simulink model "ABB_1010"  (R2024a)
(part 16 of 16)

et304 = Lx2*Lycm6*dQ1*dQ6*m6*t5*t6*t7*t9*-2.0+Lx2*Lycm6*dQ2*dQ4*m6*t3*t5*t9*t11*2.0+Lx2*Lycm6*dQ2*dQ5*m6*t3*t4*t10*t11*2.0+Lx2*Lycm6*dQ3*dQ4*m6*t3*t5*t9*t11*2.0+Lx2*Lycm6*dQ3*dQ5*m6*t3*t4*t10*t11*2.0+Lx2*Lycm6*dQ4*dQ6*m6*t5*t6*t8*t9*2.0+Lx2*Lycm6*dQ5*dQ6*m6*t4*t6*t8*t10*2.0+Lx2*Lycm6*dQ1*dQ5*m6*t7*t9*t10*t11*2.0-Lx2*Lycm6*dQ4*dQ5*m6*t8*t9*t10*t11*2.0;
et305 = t42+t45+t48+t49+t50+t51+t52+t53+t54+t55+t56+t57+t58+t59+t60+t61+t72+t73+t74+t75+t76+t77+t78+t79+t80+t81+t82+t83+t86+t92+t93+t95+t96+t97+t98+t99+t100+t101+t102+t103+t108+t109+t110+t111+t114+t115+t116+t117+t118+t127+t128+t131+t132+t137+t138+t139+t140+t141+t142+t143+t144+t145+t146+t147+t152+t153+t154+t157+t158+t160+t161+t163+t164+t165+t166+t167+t168+t169+t170+t171+t172+t173+t174+t175+t176+t177+t178+t179+t180+t181+t182+t183+t184+t185+t186+t187+t188+t189+t190+t191+t192+t199+t201+t208+t211+t212+t227+t228+t229+t230+t231+t232+t233+t234+t235+t236+t252+t253+t254+t255+t256+t257+t262+t263+t264+t265+t266+t277+t278+t279+t280+t281+t282+t289+t290+t291+t292+t293+t294+t295+t296+t297+t298+t299+t300+t301+t302+t303+t304+t305+t306+t307+t308+t309+t310+t311+t312+t313+t314+t316+t318+t320+t321+t322+t323+t324+t325+t326+t327+t328+t329+t330+t331+t332+t333+t334+t335+t336+t337+t338+t339+t340+t341+t342+t343+t344+t345+t346+t347+t348+t349+t350+t351+t352+t353+t354+t355+t356+t357+t358;
et306 = t363+t364+t365+t366+t369+t370+t371+t372+t380+t382+t383+t384+t385+t386+t387+t388+t389+t401+t402+t403+t404+t409+t410+t411+t412+t413+t414+t415+t416+t417+t418+t419+t420+t421+t422+t423+t424+t425+t426+t427+t428+t429+t430+t431+t436+t437+t438+t439+t440+t441+t442+t443+t446+t447+t450+t451+t454+t459+t460+t461+t463+t464+t465+t471+t472+t473+t474+t476+t477+t478+t479+t480+t481+t492+t493+t494+t495+t496+t497+t498+t499+t500+t501+t503+t506+t509+t510+t511+t512+t513+t516+t518+t519+t521+t522+t524+t525+t527+t528+t542+t543+t544+t545+t546+t547+t548+t549+t551+t552+t556+t557+t558+t559+t560+t561+t562+t563+t564+t565+t566+t567+t568+t569+t570+t571+t572+t573+t574+t575+t576+t577+t578+t579+t580+t581+t582+t583+t584+t585+t586+t587+t588+t589+t590+t591+t592+t593+t595+t596+t597+t598+t599+t600+t607+t608+t609+t610+t611+t612+t613+t614+t615+t616+t617+t618+t619+t620+t621+t622+t623+t624+t625+t626+t627+t628+t629+t630+t631+t632+t633+t634+t635+t636+t637+t638+t639+t640+t641+t642+t643+t644+t645+t646+t647+t648+t649+t650+t651+t654+t655;
et307 = t656+t657+t658+t659+t660+t668+t674+t675+t676+t677+t686+t687+t691+t692+t693+t694+t695+t696+t697+t701+t702+t703+t704+t705+t706+t707+t708+t709+t710+t711+t712+t713+t714+t715+t716+t724+t736+t737+t742+t743+t744+t745+t746+t747+t756+t757+t758+t761+t762+t763+t765+t767+t768+t770+t772+t773+t774+t776+t777+t778+t779+t780+t781+t782+t783+t787+t788+t789+t790+t791+t792+t793+t794+t795+t806+t807+t808+t809+t816+t819+t820+t821+t822+t823+t824+t825+t826+t827+t830+t833+t834+t836+t837+t843+t844+t845+t846+t847+t848+t849+t850+t851+t852+t853+t854+t855+t856+t857+t858+t859+t860+t861+t862+t863+t864+t865+t866+t867+t868+t869+t870+t871+t872+t873+t874+t875+t876+t877+t878+t879+t880+t881+t882+t883+t884+t885+t886+t887+t888+t889+t890+t891+t892+t893+t894+t895+t896+t897+t898+t899+t900+t901+t902+t903+t904+t905+t906+t907+t909+t910+t911+t912+t913+t914+t915+t916+t917+t918+t919+t920+t921+t922+t923+t924+t925+t926+t927+t928+t929+t930+t931+t932+t933+t934+t935+t936+t937+t938+t939+t940+t941+t942+t943+t944+t955+t957+t958+t960+t961+t967;
et308 = t968+t970+t973+t976+t979+t982+t983+t984+t985+t986+t987+t988+t989+t990+t991+t992+t993+t994+t995+t996+t997+t998+t999+t1000+t1001+t1002+t1003+t1004+t1005+t1006+t1007+t1008+t1009+t1010+t1015+t1016+t1017+t1018+t1019+t1020+t1023+t1024+t1031+t1032+t1033+t1034+t1039+t1042+t1043+t1044+t1045+t1046+t1049+t1050+t1058+t1059+t1060+t1061+t1062+t1063+t1066+t1067+t1068+t1069+t1070+t1071+t1074+t1077+t1079+t1082+t1083+t1084+t1085+t1086+t1087+t1088+t1090+t1091+t1092+t1093+t1094+t1095+t1096+t1097+t1098+t1099+t1100+t1101+t1102+t1103+t1104+t1105+t1106+t1107+t1108+t1109+t1110+t1111+t1112+t1113+t1114+t1115+t1125+t1126+t1127+t1128+t1129+t1130+t1131+t1132+t1133+t1134+t1135+t1136+t1137+t1140+t1143+t1144+t1147+t1150+t1151+t1152+t1153+t1154+t1155+t1156+t1174+t1175+t1177+t1178+t1182+t1183+t1185+t1186+t1187+t1188+t1189+t1190+t1197+t1200+t1201+t1202+t1203+t1204+t1205+t1206+t1207+t1208+t1209+t1210+t1211+t1212+t1213+t1214+t1215+t1216+t1218+t1219+t1220+t1221+t1222+t1223+t1224+t1225+t1226+t1227+t1228+t1229+t1230+t1231+t1232+t1233+t1234+t1235+t1245+t1246+t1247+t1248+t1249+t1250+t1251+t1252+t1253+t1254+t1258+t1260+t1263+t1264+t1265+t1266+t1267+t1268+t1269+t1270+t1271+t1272+t1273+t1274+t1275+t1276;
et309 = t1277+t1278+t1279+t1280+t1281+t1282+t1283+t1284+t1285+t1286+t1287+t1288+t1289+t1293+t1294+t1295+t1296+t1297+t1298+t1299+t1300+t1301+t1302+t1303+t1304+t1305+t1306+t1307+t1308+t1309+t1310+t1311+t1312+t1313+t1314+t1315+t1316+t1317+t1318+t1319+t1321+t1322+t1323+t1324+t1331+t1332+t1333+t1334+t1335+t1336+t1337+t1341+t1342+t1343+t1344+t1345+t1346+t1347+t1348+t1349+t1350+t1351+t1352+t1355+t1356+t1362+t1363+t1364+t1365+t1366+t1367+t1368+t1369+t1370+t1371+t1372+t1373+t1374+t1375+t1376+t1377+t1378+t1379+t1380+t1381+t1382+t1383+t1384+t1396+t1401+t1402+t1403+t1404+t1405+t1406+t1407+t1408+t1409+t1410+t1411+t1412+t1416+t1417+t1418+t1419+t1420+t1434+t1435+t1436+t1437+t1438+t1439+t1440+t1441+t1449+t1450+t1451+t1455+t1456+t1457+t1460+t1461+t1462+t1463+t1465+t1466+t1467+t1468+t1469+t1470+t1471+t1472+t1473+t1474+t1475+t1476+t1477+t1478+t1479+t1480+t1481+t1482+t1484+t1485+t1486+t1487+t1488+t1489+t1490+t1491+t1492+t1493+t1494+t1495+t1496+t1498+t1499+t1500+t1501+t1502+t1503+t1504+t1505+t1506+t1507+t1508+t1509+t1510+t1511+t1512+t1513+t1514+t1515+t1516+t1517+t1518+t1519+t1520+t1521+t1522+t1530+t1531+t1532+t1533+t1534+t1535+t1536+t1537+t1538+t1539+t1540+t1541+t1542+t1543+t1545+t1546+t1547+t1548+t1549+t1550;
et310 = t1557+t1558+t1561+t1562+t1563+t1564+t1565+t1566+t1573+t1574+t1575+t1578+t1579+t1580+t1586+t1587+t1594+t1595+t1596+t1597+t1598+t1599+t1600+t1601+t1602+t1603+t1604+t1605+t1606+t1607+t1608+t1609+t1610+t1611+t1612+t1613+t1614+t1615+t1618+t1619+t1620+t1621+t1622+t1623+t1624+t1625+t1626+t1627+t1628+t1629+t1645+t1646+t1647+t1648+t1649+t1650+t1651+t1652+t1653+t1654+t1655+t1656+t1657+t1658+t1662+t1663+t1664+t1665+t1667+t1668+t1669+t1670+t1671+t1676+t1677+t1678+t1683+t1685+t1686+t1687+t1688+t1689+t1690+t1691+t1692+t1693+t1694+t1695+t1696+t1697+t1698+t1699+t1700+t1701+t1706+t1707+t1708+t1709+t1710+t1711+t1712+t1713+t1714+t1715+t1716+t1717+t1718+t1719+t1720+t1721+t1722+t1727+t1728+t1729+t1730+t1731+t1732+t1735+t1736+t1737+t1738+t1739+t1740;
et311 = Ixx5*dQ2*dQ5*t9+Ixx5*dQ3*dQ5*t9+Ixx6*dQ2*dQ5*t9+Ixx6*dQ3*dQ5*t9+Ixx6*dQ5*dQ6*t10-Ixx4*dQ2*dQ3*t39+Ixx6*dQ2*dQ3*t39+Ixx5*dQ4*dQ5*t40-Ixx6*dQ4*dQ6*t41+Iyy5*dQ2*dQ5*t9+Iyy5*dQ3*dQ5*t9+Iyy6*dQ2*dQ5*t9+Iyy6*dQ3*dQ5*t9-Iyy6*dQ5*dQ6*t10+Iyy4*dQ2*dQ3*t39+Iyy5*dQ2*dQ3*t39+Iyy6*dQ4*dQ5*t40+Iyy6*dQ4*dQ6*t41-Izz5*dQ2*dQ5*t9-Izz5*dQ3*dQ5*t9-Izz6*dQ2*dQ5*t9-Izz6*dQ3*dQ5*t9-Izz6*dQ5*dQ6*t10-Izz5*dQ2*dQ3*t39-Izz6*dQ2*dQ3*t39-Izz5*dQ4*dQ5*t40-Izz6*dQ4*dQ5*t40-Lx4*Lycm4*dQ2*dQ3*m4*2.0-Lx4*Lycm5*dQ2*dQ3*m5*2.0-Lxcm4*Lycm4*dQ2*dQ3*m4*2.0-Lxcm6*Lycm6*dQ4*dQ6*m6*2.0-Lxcm5*Lzcm5*dQ4*dQ5*m5*2.0;
et312 = -Ixx4*dQ1*dQ2*t2*t8-Ixx4*dQ1*dQ2*t3*t7-Ixx4*dQ1*dQ3*t2*t8-Ixx4*dQ1*dQ3*t3*t7-Ixx5*dQ1*dQ2*t2*t8-Ixx5*dQ1*dQ2*t3*t7-Ixx5*dQ1*dQ3*t2*t8-Ixx5*dQ1*dQ3*t3*t7+Ixx6*dQ1*dQ2*t2*t8+Ixx6*dQ1*dQ2*t3*t7+Ixx6*dQ1*dQ3*t2*t8+Ixx6*dQ1*dQ3*t3*t7+Ixx6*dQ2*dQ6*t4*t10+Ixx6*dQ3*dQ6*t4*t10-Ixx5*dQ2*dQ5*t9*t35*2.0-Ixx5*dQ3*dQ5*t9*t35*2.0-Ixx6*dQ5*dQ6*t10*t36*2.0+Iyy4*dQ1*dQ2*t2*t8+Iyy4*dQ1*dQ2*t3*t7+Iyy4*dQ1*dQ3*t2*t8+Iyy4*dQ1*dQ3*t3*t7+Iyy5*dQ1*dQ2*t2*t8+Iyy5*dQ1*dQ2*t3*t7+Iyy5*dQ1*dQ3*t2*t8+Iyy5*dQ1*dQ3*t3*t7-Iyy6*dQ1*dQ2*t2*t8-Iyy6*dQ1*dQ2*t3*t7-Iyy6*dQ1*dQ3*t2*t8;
et313 = -Iyy6*dQ1*dQ3*t3*t7-Iyy6*dQ2*dQ6*t4*t10-Iyy6*dQ3*dQ6*t4*t10-Iyy6*dQ2*dQ5*t9*t35*2.0-Iyy6*dQ3*dQ5*t9*t35*2.0+Iyy6*dQ5*dQ6*t10*t36*2.0-Izz4*dQ1*dQ2*t2*t8-Izz4*dQ1*dQ2*t3*t7-Izz4*dQ1*dQ3*t2*t8-Izz4*dQ1*dQ3*t3*t7-Izz5*dQ1*dQ2*t2*t8-Izz5*dQ1*dQ2*t3*t7-Izz5*dQ1*dQ3*t2*t8-Izz5*dQ1*dQ3*t3*t7-Izz6*dQ1*dQ2*t2*t8-Izz6*dQ1*dQ2*t3*t7-Izz6*dQ1*dQ3*t2*t8-Izz6*dQ1*dQ3*t3*t7-Izz6*dQ2*dQ6*t4*t10-Izz6*dQ3*dQ6*t4*t10+Izz5*dQ2*dQ5*t9*t35*2.0+Izz5*dQ3*dQ5*t9*t35*2.0+Izz6*dQ2*dQ5*t9*t35*2.0+Izz6*dQ3*dQ5*t9*t35*2.0+dQ2*dQ5*m6*t9*t22*2.0;
et314 = dQ3*dQ5*m6*t9*t22*2.0-dQ5*dQ6*m6*t10*t18*2.0+dQ2*dQ5*m5*t9*t25*2.0+dQ3*dQ5*m5*t9*t25*2.0+dQ2*dQ5*m6*t9*t26*2.0+dQ3*dQ5*m6*t9*t26*2.0+dQ2*dQ3*m4*t14*t39+dQ2*dQ3*m5*t14*t39+dQ2*dQ3*m4*t16*t39+dQ2*dQ3*m6*t14*t39-dQ2*dQ3*m4*t19*t39-dQ2*dQ3*m6*t18*t39-dQ2*dQ3*m5*t20*t39-dQ4*dQ5*m5*t17*t40+dQ2*dQ3*m6*t22*t39+dQ2*dQ3*m5*t25*t39+dQ4*dQ6*m6*t18*t41+dQ2*dQ3*m6*t26*t39-dQ4*dQ5*m6*t21*t40+dQ4*dQ5*m6*t22*t40-dQ4*dQ6*m6*t21*t41+dQ4*dQ5*m5*t25*t40+dQ4*dQ5*m6*t26*t40-t4*t6*t10*t11*t149*2.0-t4*t6*t10*t11*t150*2.0+t4*t6*t10*t11*t153*2.0+t4*t6*t10*t11*t154*2.0+t4*t6*t10*t11*t595+t4*t6*t10*t11*t596;
et315 = Lx3*Lx4*dQ2*dQ3*m4*t9*2.0+Lx3*Lx4*dQ2*dQ3*m5*t9*2.0+Lx3*Lx4*dQ2*dQ3*m6*t9*2.0+Lx3*Lxcm4*dQ2*dQ3*m4*t9*2.0-Lx4*Lxcm6*dQ2*dQ3*m6*t11*2.0-Lx4*Lxcm5*dQ4*dQ5*m5*t10*2.0+Lx4*Lxcm4*dQ2*dQ3*m4*t39*2.0+Lx3*Lycm4*dQ2*dQ3*m4*t4*2.0+Lx3*Lycm5*dQ2*dQ3*m5*t4*2.0-Lx4*Lycm6*dQ2*dQ3*m6*t6*2.0+Lx4*Lycm4*dQ2*dQ3*m4*t34*4.0+Lx4*Lycm5*dQ2*dQ3*m5*t34*4.0-Lxcm5*Lycm5*dQ2*dQ3*m5*t5*2.0+Lxcm6*Lycm6*dQ2*dQ3*m6*t5*2.0+Lxcm4*Lycm4*dQ2*dQ3*m4*t34*4.0+Lxcm6*Lycm6*dQ4*dQ6*m6*t35*2.0+Lxcm6*Lycm6*dQ4*dQ6*m6*t36*4.0+Lx4*Lz6*dQ4*dQ5*m6*t5*2.0+Lx4*Lzcm5*dQ4*dQ5*m5*t5*2.0+Lx4*Lzcm6*dQ4*dQ5*m6*t5*2.0-Lxcm6*Lz6*dQ4*dQ5*m6*t6*2.0-Lxcm6*Lzcm6*dQ4*dQ5*m6*t6*2.0+Lxcm5*Lzcm5*dQ4*dQ5*m5*t35*4.0+Lycm6*Lz6*dQ4*dQ5*m6*t11*2.0;
et316 = Lycm5*Lzcm5*dQ2*dQ3*m5*t10*-2.0+Lycm6*Lzcm6*dQ4*dQ5*m6*t11*2.0+Lz6*Lzcm6*dQ2*dQ5*m6*t9*4.0+Lz6*Lzcm6*dQ3*dQ5*m6*t9*4.0+Lz6*Lzcm6*dQ2*dQ3*m6*t39*2.0+Lz6*Lzcm6*dQ4*dQ5*m6*t40*2.0-Ixx5*dQ1*dQ5*t2*t4*t8-Ixx5*dQ1*dQ5*t3*t4*t7-Ixx6*dQ1*dQ5*t2*t4*t8-Ixx6*dQ1*dQ5*t3*t4*t7+Ixx6*dQ2*dQ3*t5*t6*t11*2.0+Ixx4*dQ1*dQ2*t2*t8*t34*2.0+Ixx4*dQ1*dQ2*t3*t7*t34*2.0+Ixx4*dQ1*dQ3*t2*t8*t34*2.0+Ixx4*dQ1*dQ3*t3*t7*t34*2.0-Ixx6*dQ1*dQ2*t2*t8*t34*2.0-Ixx6*dQ1*dQ2*t3*t7*t34*2.0-Ixx6*dQ1*dQ3*t2*t8*t34*2.0-Ixx6*dQ1*dQ3*t3*t7*t34*2.0-Ixx6*dQ1*dQ2*t2*t8*t36*2.0-Ixx6*dQ1*dQ2*t3*t7*t36*2.0-Ixx6*dQ1*dQ3*t2*t8*t36*2.0-Ixx6*dQ1*dQ3*t3*t7*t36*2.0;
et317 = Ixx5*dQ2*dQ3*t4*t9*t35*-2.0-Ixx6*dQ2*dQ3*t4*t9*t36*2.0-Ixx6*dQ2*dQ6*t4*t10*t36*2.0-Ixx6*dQ3*dQ6*t4*t10*t36*2.0+Ixx6*dQ4*dQ5*t5*t10*t36*2.0+Ixx6*dQ4*dQ6*t6*t11*t35*2.0-Ixx6*dQ2*dQ5*t9*t35*t36*2.0-Ixx6*dQ3*dQ5*t9*t35*t36*2.0-Iyy5*dQ1*dQ5*t2*t4*t8-Iyy5*dQ1*dQ5*t3*t4*t7-Iyy6*dQ1*dQ5*t2*t4*t8-Iyy6*dQ1*dQ5*t3*t4*t7-Iyy6*dQ2*dQ3*t5*t6*t11*2.0-Iyy4*dQ1*dQ2*t2*t8*t34*2.0-Iyy4*dQ1*dQ2*t3*t7*t34*2.0-Iyy4*dQ1*dQ3*t2*t8*t34*2.0-Iyy4*dQ1*dQ3*t3*t7*t34*2.0-Iyy5*dQ1*dQ2*t2*t8*t34*2.0-Iyy5*dQ1*dQ2*t3*t7*t34*2.0-Iyy5*dQ1*dQ3*t2*t8*t34*2.0-Iyy5*dQ1*dQ3*t3*t7*t34*2.0+Iyy6*dQ1*dQ2*t2*t8*t36*2.0;
et318 = Iyy6*dQ1*dQ2*t3*t7*t36*2.0+Iyy6*dQ1*dQ3*t2*t8*t36*2.0+Iyy6*dQ1*dQ3*t3*t7*t36*2.0-Iyy6*dQ2*dQ3*t4*t9*t35*2.0+Iyy6*dQ2*dQ3*t4*t9*t36*2.0+Iyy6*dQ2*dQ6*t4*t10*t36*2.0+Iyy6*dQ3*dQ6*t4*t10*t36*2.0-Iyy6*dQ4*dQ5*t5*t10*t36*2.0-Iyy6*dQ4*dQ6*t6*t11*t35*2.0+Iyy6*dQ2*dQ5*t9*t35*t36*2.0+Iyy6*dQ3*dQ5*t9*t35*t36*2.0+Izz5*dQ1*dQ5*t2*t4*t8+Izz5*dQ1*dQ5*t3*t4*t7+Izz6*dQ1*dQ5*t2*t4*t8+Izz6*dQ1*dQ5*t3*t4*t7+Izz5*dQ1*dQ2*t2*t8*t34*2.0+Izz5*dQ1*dQ2*t3*t7*t34*2.0+Izz5*dQ1*dQ3*t2*t8*t34*2.0+Izz5*dQ1*dQ3*t3*t7*t34*2.0+Izz6*dQ1*dQ2*t2*t8*t34*2.0+Izz6*dQ1*dQ2*t3*t7*t34*2.0+Izz6*dQ1*dQ3*t2*t8*t34*2.0+Izz6*dQ1*dQ3*t3*t7*t34*2.0+Izz5*dQ2*dQ3*t4*t9*t35*2.0+Izz6*dQ2*dQ3*t4*t9*t35*2.0;
et319 = dQ1*dQ2*m4*t2*t8*t19*-2.0-dQ1*dQ2*m4*t3*t7*t19*2.0-dQ1*dQ2*m6*t2*t8*t18*2.0-dQ1*dQ2*m6*t3*t7*t18*2.0-dQ1*dQ3*m4*t2*t8*t19*2.0-dQ1*dQ3*m4*t3*t7*t19*2.0-dQ1*dQ2*m5*t2*t8*t20*2.0-dQ1*dQ2*m5*t3*t7*t20*2.0-dQ1*dQ3*m6*t2*t8*t18*2.0-dQ1*dQ3*m6*t3*t7*t18*2.0-dQ1*dQ3*m5*t2*t8*t20*2.0-dQ1*dQ3*m5*t3*t7*t20*2.0-dQ2*dQ6*m6*t4*t10*t18*2.0-dQ3*dQ6*m6*t4*t10*t18*2.0+dQ2*dQ5*m5*t9*t17*t35*2.0+dQ3*dQ5*m5*t9*t17*t35*2.0+dQ2*dQ5*m6*t9*t21*t35*2.0-dQ2*dQ5*m6*t9*t22*t35*2.0+dQ3*dQ5*m6*t9*t21*t35*2.0-dQ3*dQ5*m6*t9*t22*t35*2.0-dQ2*dQ5*m5*t9*t25*t35*2.0+dQ5*dQ6*m6*t10*t18*t36*2.0;
et320 = dQ3*dQ5*m5*t9*t25*t35*-2.0-dQ2*dQ5*m6*t9*t26*t35*2.0-dQ3*dQ5*m6*t9*t26*t35*2.0-dQ5*dQ6*m6*t10*t21*t36*2.0-Lx2*Lx4*dQ1*dQ2*m4*t4*t7*2.0-Lx2*Lx4*dQ1*dQ2*m5*t4*t7*2.0-Lx2*Lx4*dQ1*dQ2*m6*t4*t7*2.0-Lx2*Lxcm4*dQ1*dQ2*m4*t4*t7*2.0+Lx3*Lxcm5*dQ2*dQ3*m5*t5*t9*2.0+Lx3*Lxcm6*dQ2*dQ3*m6*t4*t11*2.0+Lx4*Lxcm5*dQ2*dQ5*m5*t5*t9*2.0+Lx4*Lxcm5*dQ3*dQ5*m5*t5*t9*2.0-Lx4*Lxcm6*dQ4*dQ5*m6*t6*t10*2.0-Lx4*Lxcm6*dQ4*dQ6*m6*t5*t11*2.0+Lx4*Lxcm6*dQ2*dQ3*m6*t11*t34*4.0+Lx2*Lycm4*dQ1*dQ2*m4*t7*t9*2.0+Lx3*Lycm6*dQ2*dQ3*m6*t4*t6*2.0+Lx2*Lycm5*dQ1*dQ2*m5*t7*t9*2.0-Lx4*Lycm6*dQ4*dQ6*m6*t5*t6*2.0+Lx4*Lycm6*dQ4*dQ5*m6*t10*t11*2.0+Lx4*Lycm6*dQ2*dQ3*m6*t6*t34*4.0;
et321 = Lxcm6*Lycm6*dQ1*dQ6*m6*t2*t3*-2.0+Lxcm5*Lycm5*dQ2*dQ5*m5*t4*t5*2.0+Lxcm5*Lycm5*dQ3*dQ5*m5*t4*t5*2.0-Lxcm6*Lycm6*dQ2*dQ5*m6*t4*t5*2.0-Lxcm6*Lycm6*dQ3*dQ5*m6*t4*t5*2.0+Lxcm6*Lycm6*dQ1*dQ6*m6*t7*t8*2.0+Lxcm5*Lycm5*dQ2*dQ3*m5*t5*t34*4.0-Lxcm6*Lycm6*dQ2*dQ3*m6*t5*t34*4.0-Lxcm6*Lycm6*dQ2*dQ3*m6*t5*t36*4.0-Lxcm6*Lycm6*dQ4*dQ6*m6*t35*t36*4.0+Lx3*Lz6*dQ2*dQ3*m6*t9*t10*2.0+Lx4*Lz6*dQ2*dQ5*m6*t9*t10*2.0+Lx4*Lz6*dQ3*dQ5*m6*t9*t10*2.0+Lx3*Lzcm5*dQ2*dQ3*m5*t9*t10*2.0+Lx3*Lzcm6*dQ2*dQ3*m6*t9*t10*2.0+Lx4*Lzcm5*dQ2*dQ5*m5*t9*t10*2.0+Lx4*Lzcm5*dQ3*dQ5*m5*t9*t10*2.0+Lx4*Lzcm6*dQ2*dQ5*m6*t9*t10*2.0+Lx4*Lzcm6*dQ3*dQ5*m6*t9*t10*2.0-Lxcm6*Lz6*dQ2*dQ3*m6*t10*t11*2.0-Lxcm6*Lz6*dQ2*dQ6*m6*t9*t11*2.0;
et322 = Lxcm6*Lz6*dQ3*dQ6*m6*t9*t11*-2.0+Lxcm6*Lz6*dQ4*dQ5*m6*t6*t35*4.0-Lxcm5*Lzcm5*dQ1*dQ5*m5*t2*t3*2.0+Lxcm5*Lzcm5*dQ1*dQ5*m5*t7*t8*2.0-Lxcm6*Lzcm6*dQ2*dQ3*m6*t10*t11*2.0-Lxcm6*Lzcm6*dQ2*dQ6*m6*t9*t11*2.0-Lxcm6*Lzcm6*dQ3*dQ6*m6*t9*t11*2.0+Lxcm6*Lzcm6*dQ4*dQ5*m6*t6*t35*4.0-Lycm6*Lz6*dQ2*dQ3*m6*t6*t10*2.0-Lycm6*Lz6*dQ2*dQ6*m6*t6*t9*2.0-Lycm6*Lz6*dQ3*dQ6*m6*t6*t9*2.0-Lycm6*Lz6*dQ4*dQ5*m6*t11*t35*4.0+Lycm5*Lzcm5*dQ2*dQ5*m5*t4*t10*2.0+Lycm5*Lzcm5*dQ3*dQ5*m5*t4*t10*2.0-Lycm6*Lzcm6*dQ2*dQ3*m6*t6*t10*2.0-Lycm6*Lzcm6*dQ2*dQ6*m6*t6*t9*2.0-Lycm6*Lzcm6*dQ3*dQ6*m6*t6*t9*2.0+Lycm5*Lzcm5*dQ2*dQ3*m5*t10*t34*4.0-Lycm6*Lzcm6*dQ4*dQ5*m6*t11*t35*4.0-Lz6*Lzcm6*dQ2*dQ5*m6*t9*t35*4.0;
et323 = Lz6*Lzcm6*dQ3*dQ5*m6*t9*t35*-4.0+Ixx5*dQ1*dQ5*t2*t3*t5*t10*2.0-Ixx6*dQ1*dQ6*t2*t3*t6*t11*2.0-Ixx6*dQ2*dQ5*t4*t5*t6*t11*2.0-Ixx6*dQ3*dQ5*t4*t5*t6*t11*2.0-Ixx5*dQ1*dQ5*t5*t7*t8*t10*2.0+Ixx6*dQ1*dQ6*t2*t8*t9*t10+Ixx6*dQ1*dQ6*t3*t7*t9*t10+Ixx6*dQ1*dQ6*t6*t7*t8*t11*2.0+Ixx5*dQ1*dQ5*t2*t4*t8*t35*2.0+Ixx5*dQ1*dQ5*t3*t4*t7*t35*2.0-Ixx6*dQ2*dQ3*t5*t6*t11*t34*4.0+Ixx5*dQ1*dQ2*t2*t8*t34*t35*2.0+Ixx5*dQ1*dQ2*t3*t7*t34*t35*2.0+Ixx5*dQ1*dQ3*t2*t8*t34*t35*2.0+Ixx5*dQ1*dQ3*t3*t7*t34*t35*2.0+Ixx6*dQ1*dQ2*t2*t8*t34*t36*2.0+Ixx6*dQ1*dQ2*t3*t7*t34*t36*2.0+Ixx6*dQ1*dQ3*t2*t8*t34*t36*2.0+Ixx6*dQ1*dQ3*t3*t7*t34*t36*2.0-Ixx6*dQ2*dQ3*t4*t9*t35*t36*2.0;
et324 = Iyy6*dQ1*dQ5*t2*t3*t5*t10*2.0+Iyy6*dQ1*dQ6*t2*t3*t6*t11*2.0+Iyy6*dQ2*dQ5*t4*t5*t6*t11*2.0+Iyy6*dQ3*dQ5*t4*t5*t6*t11*2.0-Iyy6*dQ1*dQ5*t5*t7*t8*t10*2.0-Iyy6*dQ1*dQ6*t2*t8*t9*t10-Iyy6*dQ1*dQ6*t3*t7*t9*t10-Iyy6*dQ1*dQ6*t6*t7*t8*t11*2.0+Iyy6*dQ1*dQ5*t2*t4*t8*t35*2.0+Iyy6*dQ1*dQ5*t3*t4*t7*t35*2.0+Iyy6*dQ2*dQ3*t5*t6*t11*t34*4.0+Iyy6*dQ1*dQ2*t2*t8*t34*t35*2.0+Iyy6*dQ1*dQ2*t3*t7*t34*t35*2.0-Iyy6*dQ1*dQ2*t2*t8*t34*t36*2.0-Iyy6*dQ1*dQ2*t3*t7*t34*t36*2.0+Iyy6*dQ1*dQ3*t2*t8*t34*t35*2.0+Iyy6*dQ1*dQ3*t3*t7*t34*t35*2.0-Iyy6*dQ1*dQ3*t2*t8*t34*t36*2.0-Iyy6*dQ1*dQ3*t3*t7*t34*t36*2.0+Iyy6*dQ2*dQ3*t4*t9*t35*t36*2.0-Izz5*dQ1*dQ5*t2*t3*t5*t10*2.0;
et325 = Izz6*dQ1*dQ5*t2*t3*t5*t10*-2.0+Izz5*dQ1*dQ5*t5*t7*t8*t10*2.0+Izz6*dQ1*dQ5*t5*t7*t8*t10*2.0-Izz6*dQ1*dQ6*t2*t8*t9*t10-Izz6*dQ1*dQ6*t3*t7*t9*t10-Izz5*dQ1*dQ5*t2*t4*t8*t35*2.0-Izz5*dQ1*dQ5*t3*t4*t7*t35*2.0-Izz6*dQ1*dQ5*t2*t4*t8*t35*2.0-Izz6*dQ1*dQ5*t3*t4*t7*t35*2.0-Izz5*dQ1*dQ2*t2*t8*t34*t35*2.0-Izz5*dQ1*dQ2*t3*t7*t34*t35*2.0-Izz5*dQ1*dQ3*t2*t8*t34*t35*2.0-Izz5*dQ1*dQ3*t3*t7*t34*t35*2.0-Izz6*dQ1*dQ2*t2*t8*t34*t35*2.0-Izz6*dQ1*dQ2*t3*t7*t34*t35*2.0-Izz6*dQ1*dQ3*t2*t8*t34*t35*2.0-Izz6*dQ1*dQ3*t3*t7*t34*t35*2.0-dQ1*dQ5*m6*t2*t4*t8*t22*2.0-dQ1*dQ5*m6*t3*t4*t7*t22*2.0-dQ1*dQ5*m5*t2*t4*t8*t25*2.0;
et326 = dQ1*dQ5*m5*t3*t4*t7*t25*-2.0-dQ2*dQ3*m6*t5*t6*t11*t18*2.0-dQ1*dQ5*m6*t2*t4*t8*t26*2.0-dQ1*dQ5*m6*t3*t4*t7*t26*2.0+dQ2*dQ3*m6*t5*t6*t11*t21*2.0-dQ1*dQ2*m4*t2*t8*t14*t34*2.0-dQ1*dQ2*m4*t3*t7*t14*t34*2.0-dQ1*dQ2*m5*t2*t8*t14*t34*2.0-dQ1*dQ2*m5*t3*t7*t14*t34*2.0-dQ1*dQ3*m4*t2*t8*t14*t34*2.0-dQ1*dQ3*m4*t3*t7*t14*t34*2.0-dQ1*dQ2*m4*t2*t8*t16*t34*2.0-dQ1*dQ2*m4*t3*t7*t16*t34*2.0-dQ1*dQ2*m6*t2*t8*t14*t34*2.0-dQ1*dQ2*m6*t3*t7*t14*t34*2.0-dQ1*dQ3*m5*t2*t8*t14*t34*2.0-dQ1*dQ3*m5*t3*t7*t14*t34*2.0-dQ1*dQ3*m4*t2*t8*t16*t34*2.0-dQ1*dQ3*m4*t3*t7*t16*t34*2.0-dQ1*dQ3*m6*t2*t8*t14*t34*2.0;
et327 = dQ1*dQ3*m6*t3*t7*t14*t34*-2.0+dQ1*dQ2*m4*t2*t8*t19*t34*2.0+dQ1*dQ2*m4*t3*t7*t19*t34*2.0+dQ1*dQ2*m6*t2*t8*t18*t34*2.0+dQ1*dQ2*m6*t3*t7*t18*t34*2.0+dQ1*dQ3*m4*t2*t8*t19*t34*2.0+dQ1*dQ3*m4*t3*t7*t19*t34*2.0+dQ1*dQ2*m5*t2*t8*t20*t34*2.0+dQ1*dQ2*m5*t3*t7*t20*t34*2.0+dQ1*dQ3*m6*t2*t8*t18*t34*2.0+dQ1*dQ3*m6*t3*t7*t18*t34*2.0+dQ1*dQ2*m6*t2*t8*t18*t36*2.0+dQ1*dQ2*m6*t3*t7*t18*t36*2.0+dQ1*dQ3*m5*t2*t8*t20*t34*2.0+dQ1*dQ3*m5*t3*t7*t20*t34*2.0+dQ1*dQ3*m6*t2*t8*t18*t36*2.0+dQ1*dQ3*m6*t3*t7*t18*t36*2.0-dQ1*dQ2*m6*t2*t8*t22*t34*2.0-dQ1*dQ2*m6*t3*t7*t22*t34*2.0+dQ2*dQ3*m5*t4*t9*t17*t35*2.0-dQ1*dQ2*m6*t2*t8*t21*t36*2.0;
et328 = dQ1*dQ2*m6*t3*t7*t21*t36*-2.0-dQ1*dQ3*m6*t2*t8*t22*t34*2.0-dQ1*dQ3*m6*t3*t7*t22*t34*2.0-dQ1*dQ2*m5*t2*t8*t25*t34*2.0-dQ1*dQ2*m5*t3*t7*t25*t34*2.0-dQ1*dQ3*m6*t2*t8*t21*t36*2.0-dQ1*dQ3*m6*t3*t7*t21*t36*2.0-dQ1*dQ3*m5*t2*t8*t25*t34*2.0-dQ1*dQ3*m5*t3*t7*t25*t34*2.0+dQ2*dQ3*m6*t4*t9*t18*t36*2.0-dQ1*dQ2*m6*t2*t8*t26*t34*2.0-dQ1*dQ2*m6*t3*t7*t26*t34*2.0-dQ1*dQ3*m6*t2*t8*t26*t34*2.0-dQ1*dQ3*m6*t3*t7*t26*t34*2.0+dQ2*dQ3*m6*t4*t9*t21*t35*2.0-dQ2*dQ3*m6*t4*t9*t21*t36*2.0-dQ2*dQ3*m6*t4*t9*t22*t35*2.0+dQ2*dQ6*m6*t4*t10*t18*t36*2.0-dQ2*dQ3*m5*t4*t9*t25*t35*2.0+dQ3*dQ6*m6*t4*t10*t18*t36*2.0;
et329 = dQ4*dQ5*m6*t5*t10*t18*t36*-2.0-dQ2*dQ3*m6*t4*t9*t26*t35*2.0-dQ2*dQ6*m6*t4*t10*t21*t36*2.0-dQ3*dQ6*m6*t4*t10*t21*t36*2.0-dQ4*dQ6*m6*t6*t11*t18*t35*2.0+dQ4*dQ5*m6*t5*t10*t21*t36*2.0+dQ4*dQ6*m6*t6*t11*t21*t35*2.0+dQ2*dQ5*m6*t9*t18*t35*t36*2.0+dQ3*dQ5*m6*t9*t18*t35*t36*2.0-dQ2*dQ5*m6*t9*t21*t35*t36*2.0-dQ3*dQ5*m6*t9*t21*t35*t36*2.0-Lx3*Lx4*dQ1*dQ2*m4*t2*t4*t8*2.0-Lx3*Lx4*dQ1*dQ2*m4*t3*t4*t7*2.0-Lx3*Lx4*dQ1*dQ2*m5*t2*t4*t8*2.0-Lx3*Lx4*dQ1*dQ2*m5*t3*t4*t7*2.0-Lx3*Lx4*dQ1*dQ3*m4*t2*t4*t8*2.0-Lx3*Lx4*dQ1*dQ3*m4*t3*t4*t7*2.0-Lx3*Lx4*dQ1*dQ2*m6*t2*t4*t8*2.0-Lx3*Lx4*dQ1*dQ2*m6*t3*t4*t7*2.0;
et330 = Lx3*Lx4*dQ1*dQ3*m5*t2*t4*t8*-2.0-Lx3*Lx4*dQ1*dQ3*m5*t3*t4*t7*2.0-Lx3*Lx4*dQ1*dQ3*m6*t2*t4*t8*2.0-Lx3*Lx4*dQ1*dQ3*m6*t3*t4*t7*2.0-Lx3*Lxcm4*dQ1*dQ2*m4*t2*t4*t8*2.0-Lx3*Lxcm4*dQ1*dQ2*m4*t3*t4*t7*2.0-Lx3*Lxcm4*dQ1*dQ3*m4*t2*t4*t8*2.0-Lx3*Lxcm4*dQ1*dQ3*m4*t3*t4*t7*2.0-Lx2*Lxcm5*dQ1*dQ2*m5*t4*t5*t7*2.0-Lx4*Lxcm5*dQ1*dQ5*m5*t2*t3*t10*2.0+Lx4*Lxcm5*dQ2*dQ3*m5*t4*t5*t9*4.0+Lx3*Lxcm6*dQ2*dQ3*m6*t5*t6*t9*2.0+Lx4*Lxcm6*dQ2*dQ5*m6*t5*t6*t9*2.0+Lx2*Lxcm6*dQ1*dQ2*m6*t7*t9*t11*2.0+Lx4*Lxcm6*dQ3*dQ5*m6*t5*t6*t9*2.0+Lx4*Lxcm5*dQ1*dQ5*m5*t7*t8*t10*2.0-Lx4*Lxcm6*dQ2*dQ6*m6*t9*t10*t11*2.0-Lx4*Lxcm6*dQ3*dQ6*m6*t9*t10*t11*2.0;
et331 = Lx4*Lxcm4*dQ1*dQ2*m4*t2*t8*t34*-4.0-Lx4*Lxcm4*dQ1*dQ2*m4*t3*t7*t34*4.0-Lx4*Lxcm4*dQ1*dQ3*m4*t2*t8*t34*4.0-Lx4*Lxcm4*dQ1*dQ3*m4*t3*t7*t34*4.0+Lx3*Lycm4*dQ1*dQ2*m4*t2*t8*t9*2.0+Lx3*Lycm4*dQ1*dQ2*m4*t3*t7*t9*2.0+Lx3*Lycm4*dQ1*dQ3*m4*t2*t8*t9*2.0+Lx3*Lycm4*dQ1*dQ3*m4*t3*t7*t9*2.0+Lx3*Lycm5*dQ1*dQ2*m5*t2*t8*t9*2.0+Lx3*Lycm5*dQ1*dQ2*m5*t3*t7*t9*2.0+Lx3*Lycm5*dQ1*dQ3*m5*t2*t8*t9*2.0+Lx3*Lycm5*dQ1*dQ3*m5*t3*t7*t9*2.0+Lx2*Lycm6*dQ1*dQ2*m6*t6*t7*t9*2.0-Lx3*Lycm6*dQ2*dQ3*m6*t5*t9*t11*2.0-Lx4*Lycm6*dQ2*dQ5*m6*t5*t9*t11*2.0-Lx4*Lycm6*dQ2*dQ6*m6*t6*t9*t10*2.0-Lx4*Lycm6*dQ3*dQ5*m6*t5*t9*t11*2.0-Lx4*Lycm6*dQ3*dQ6*m6*t6*t9*t10*2.0+Lxcm6*Lycm6*dQ2*dQ6*m6*t5*t9*t10*2.0;
et332 = Lxcm6*Lycm6*dQ3*dQ6*m6*t5*t9*t10*2.0-Lxcm6*Lycm6*dQ5*dQ6*m6*t6*t10*t11*4.0+Lxcm6*Lycm6*dQ1*dQ6*m6*t2*t3*t35*2.0+Lxcm6*Lycm6*dQ1*dQ6*m6*t2*t3*t36*4.0+Lxcm6*Lycm6*dQ2*dQ5*m6*t4*t5*t36*4.0+Lxcm6*Lycm6*dQ3*dQ5*m6*t4*t5*t36*4.0-Lxcm6*Lycm6*dQ1*dQ6*m6*t7*t8*t35*2.0-Lxcm6*Lycm6*dQ1*dQ6*m6*t7*t8*t36*4.0+Lxcm6*Lycm6*dQ2*dQ3*m6*t5*t34*t36*8.0+Lx4*Lz6*dQ1*dQ5*m6*t2*t3*t5*2.0-Lx2*Lz6*dQ1*dQ2*m6*t4*t7*t10*2.0-Lx4*Lz6*dQ1*dQ5*m6*t5*t7*t8*2.0+Lx4*Lz6*dQ2*dQ3*m6*t4*t9*t10*4.0+Lx4*Lzcm4*dQ1*dQ2*m4*t2*t3*t4*2.0+Lx4*Lzcm4*dQ1*dQ3*m4*t2*t3*t4*2.0+Lx4*Lzcm5*dQ1*dQ5*m5*t2*t3*t5*2.0+Lx4*Lzcm6*dQ1*dQ5*m6*t2*t3*t5*2.0-Lx4*Lzcm4*dQ1*dQ2*m4*t4*t7*t8*2.0-Lx4*Lzcm4*dQ1*dQ3*m4*t4*t7*t8*2.0;
et333 = Lxcm6*Lz6*dQ1*dQ5*m6*t2*t3*t6*-2.0-Lx2*Lzcm5*dQ1*dQ2*m5*t4*t7*t10*2.0-Lx2*Lzcm6*dQ1*dQ2*m6*t4*t7*t10*2.0-Lx4*Lzcm5*dQ1*dQ5*m5*t5*t7*t8*2.0+Lx4*Lzcm5*dQ2*dQ3*m5*t4*t9*t10*4.0-Lx4*Lzcm6*dQ1*dQ5*m6*t5*t7*t8*2.0+Lx4*Lzcm6*dQ2*dQ3*m6*t4*t9*t10*4.0+Lxcm6*Lz6*dQ1*dQ5*m6*t6*t7*t8*2.0+Lxcm6*Lz6*dQ2*dQ5*m6*t4*t10*t11*2.0+Lxcm6*Lz6*dQ3*dQ5*m6*t4*t10*t11*2.0-Lxcm6*Lz6*dQ4*dQ6*m6*t5*t10*t11*2.0+Lxcm6*Lz6*dQ2*dQ3*m6*t10*t11*t34*4.0+Lxcm6*Lz6*dQ2*dQ6*m6*t9*t11*t35*2.0+Lxcm6*Lz6*dQ3*dQ6*m6*t9*t11*t35*2.0+Lxcm4*Lzcm4*dQ1*dQ2*m4*t2*t3*t4*2.0+Lxcm4*Lzcm4*dQ1*dQ3*m4*t2*t3*t4*2.0-Lxcm5*Lzcm5*dQ1*dQ2*m5*t2*t3*t4*2.0-Lxcm5*Lzcm5*dQ1*dQ3*m5*t2*t3*t4*2.0-Lxcm4*Lzcm4*dQ1*dQ2*m4*t4*t7*t8*2.0;
et334 = Lxcm4*Lzcm4*dQ1*dQ3*m4*t4*t7*t8*-2.0-Lxcm6*Lzcm6*dQ1*dQ5*m6*t2*t3*t6*2.0+Lxcm5*Lzcm5*dQ1*dQ2*m5*t4*t7*t8*2.0+Lxcm5*Lzcm5*dQ1*dQ3*m5*t4*t7*t8*2.0+Lxcm6*Lzcm6*dQ1*dQ5*m6*t6*t7*t8*2.0+Lxcm5*Lzcm5*dQ2*dQ5*m5*t5*t9*t10*4.0+Lxcm5*Lzcm5*dQ3*dQ5*m5*t5*t9*t10*4.0+Lxcm6*Lzcm6*dQ2*dQ5*m6*t4*t10*t11*2.0+Lxcm6*Lzcm6*dQ3*dQ5*m6*t4*t10*t11*2.0-Lxcm6*Lzcm6*dQ4*dQ6*m6*t5*t10*t11*2.0+Lxcm5*Lzcm5*dQ1*dQ5*m5*t2*t3*t35*4.0-Lxcm5*Lzcm5*dQ1*dQ5*m5*t7*t8*t35*4.0+Lxcm6*Lzcm6*dQ2*dQ3*m6*t10*t11*t34*4.0+Lxcm6*Lzcm6*dQ2*dQ6*m6*t9*t11*t35*2.0+Lxcm6*Lzcm6*dQ3*dQ6*m6*t9*t11*t35*2.0+Lycm6*Lz6*dQ1*dQ5*m6*t2*t3*t11*2.0+Lycm6*Lz6*dQ2*dQ5*m6*t4*t6*t10*2.0+Lycm6*Lz6*dQ3*dQ5*m6*t4*t6*t10*2.0-Lycm6*Lz6*dQ4*dQ6*m6*t5*t6*t10*2.0;
et335 = Lycm6*Lz6*dQ1*dQ5*m6*t7*t8*t11*-2.0+Lycm6*Lz6*dQ2*dQ3*m6*t6*t10*t34*4.0+Lycm6*Lz6*dQ2*dQ6*m6*t6*t9*t35*2.0+Lycm6*Lz6*dQ3*dQ6*m6*t6*t9*t35*2.0-Lycm4*Lzcm4*dQ1*dQ2*m4*t2*t3*t9*2.0-Lycm4*Lzcm4*dQ1*dQ3*m4*t2*t3*t9*2.0+Lycm4*Lzcm4*dQ1*dQ2*m4*t7*t8*t9*2.0+Lycm4*Lzcm4*dQ1*dQ3*m4*t7*t8*t9*2.0+Lycm6*Lzcm6*dQ1*dQ5*m6*t2*t3*t11*2.0+Lycm6*Lzcm6*dQ2*dQ5*m6*t4*t6*t10*2.0+Lycm6*Lzcm6*dQ3*dQ5*m6*t4*t6*t10*2.0-Lycm6*Lzcm6*dQ4*dQ6*m6*t5*t6*t10*2.0-Lycm6*Lzcm6*dQ1*dQ5*m6*t7*t8*t11*2.0+Lycm6*Lzcm6*dQ2*dQ3*m6*t6*t10*t34*4.0+Lycm6*Lzcm6*dQ2*dQ6*m6*t6*t9*t35*2.0+Lycm6*Lzcm6*dQ3*dQ6*m6*t6*t9*t35*2.0-Lz6*Lzcm6*dQ1*dQ5*m6*t2*t4*t8*4.0-Lz6*Lzcm6*dQ1*dQ5*m6*t3*t4*t7*4.0-Lz6*Lzcm6*dQ1*dQ2*m6*t2*t8*t34*4.0;
et336 = Lz6*Lzcm6*dQ1*dQ2*m6*t3*t7*t34*-4.0-Lz6*Lzcm6*dQ1*dQ3*m6*t2*t8*t34*4.0-Lz6*Lzcm6*dQ1*dQ3*m6*t3*t7*t34*4.0-Lz6*Lzcm6*dQ2*dQ3*m6*t4*t9*t35*4.0+Ixx5*dQ1*dQ2*t2*t3*t4*t5*t10*2.0+Ixx5*dQ1*dQ3*t2*t3*t4*t5*t10*2.0-Ixx5*dQ1*dQ2*t4*t5*t7*t8*t10*2.0-Ixx5*dQ1*dQ3*t4*t5*t7*t8*t10*2.0+Ixx6*dQ2*dQ6*t5*t6*t9*t10*t11*2.0+Ixx6*dQ3*dQ6*t5*t6*t9*t10*t11*2.0+Ixx6*dQ1*dQ5*t2*t3*t5*t10*t36*2.0+Ixx6*dQ1*dQ6*t2*t3*t6*t11*t35*2.0-Ixx6*dQ1*dQ5*t5*t7*t8*t10*t36*2.0-Ixx6*dQ1*dQ6*t2*t8*t9*t10*t36*2.0-Ixx6*dQ1*dQ6*t3*t7*t9*t10*t36*2.0-Ixx6*dQ1*dQ6*t6*t7*t8*t11*t35*2.0+Ixx6*dQ1*dQ5*t2*t4*t8*t35*t36*2.0+Ixx6*dQ1*dQ5*t3*t4*t7*t35*t36*2.0+Ixx6*dQ1*dQ2*t2*t8*t34*t35*t36*2.0;
et337 = Ixx6*dQ1*dQ2*t3*t7*t34*t35*t36*2.0+Ixx6*dQ1*dQ3*t2*t8*t34*t35*t36*2.0+Ixx6*dQ1*dQ3*t3*t7*t34*t35*t36*2.0+Iyy6*dQ1*dQ2*t2*t3*t4*t5*t10*2.0+Iyy6*dQ1*dQ3*t2*t3*t4*t5*t10*2.0-Iyy6*dQ1*dQ2*t4*t5*t7*t8*t10*2.0-Iyy6*dQ1*dQ3*t4*t5*t7*t8*t10*2.0-Iyy6*dQ2*dQ6*t5*t6*t9*t10*t11*2.0-Iyy6*dQ3*dQ6*t5*t6*t9*t10*t11*2.0-Iyy6*dQ1*dQ5*t2*t3*t5*t10*t36*2.0-Iyy6*dQ1*dQ6*t2*t3*t6*t11*t35*2.0+Iyy6*dQ1*dQ5*t5*t7*t8*t10*t36*2.0+Iyy6*dQ1*dQ6*t2*t8*t9*t10*t36*2.0+Iyy6*dQ1*dQ6*t3*t7*t9*t10*t36*2.0+Iyy6*dQ1*dQ6*t6*t7*t8*t11*t35*2.0-Iyy6*dQ1*dQ5*t2*t4*t8*t35*t36*2.0-Iyy6*dQ1*dQ5*t3*t4*t7*t35*t36*2.0-Iyy6*dQ1*dQ2*t2*t8*t34*t35*t36*2.0-Iyy6*dQ1*dQ2*t3*t7*t34*t35*t36*2.0;
et338 = Iyy6*dQ1*dQ3*t2*t8*t34*t35*t36*-2.0-Iyy6*dQ1*dQ3*t3*t7*t34*t35*t36*2.0-Izz5*dQ1*dQ2*t2*t3*t4*t5*t10*2.0-Izz5*dQ1*dQ3*t2*t3*t4*t5*t10*2.0-Izz6*dQ1*dQ2*t2*t3*t4*t5*t10*2.0-Izz6*dQ1*dQ3*t2*t3*t4*t5*t10*2.0+Izz5*dQ1*dQ2*t4*t5*t7*t8*t10*2.0+Izz5*dQ1*dQ3*t4*t5*t7*t8*t10*2.0+Izz6*dQ1*dQ2*t4*t5*t7*t8*t10*2.0+Izz6*dQ1*dQ3*t4*t5*t7*t8*t10*2.0-dQ1*dQ5*m5*t2*t3*t5*t10*t17*2.0-dQ1*dQ5*m6*t2*t3*t5*t10*t21*2.0+dQ1*dQ6*m6*t2*t3*t6*t11*t18*2.0+dQ1*dQ5*m6*t2*t3*t5*t10*t22*2.0+dQ1*dQ5*m5*t2*t3*t5*t10*t25*2.0-dQ1*dQ6*m6*t2*t3*t6*t11*t21*2.0+dQ2*dQ5*m6*t4*t5*t6*t11*t18*2.0+dQ1*dQ5*m5*t5*t7*t8*t10*t17*2.0+dQ1*dQ5*m6*t2*t3*t5*t10*t26*2.0;
et339 = dQ3*dQ5*m6*t4*t5*t6*t11*t18*2.0-dQ1*dQ6*m6*t2*t8*t9*t10*t18*2.0-dQ1*dQ6*m6*t3*t7*t9*t10*t18*2.0-dQ2*dQ5*m6*t4*t5*t6*t11*t21*2.0-dQ3*dQ5*m6*t4*t5*t6*t11*t21*2.0+dQ1*dQ5*m6*t5*t7*t8*t10*t21*2.0-dQ1*dQ6*m6*t6*t7*t8*t11*t18*2.0-dQ1*dQ5*m6*t5*t7*t8*t10*t22*2.0-dQ1*dQ5*m5*t5*t7*t8*t10*t25*2.0+dQ1*dQ6*m6*t6*t7*t8*t11*t21*2.0-dQ1*dQ5*m6*t5*t7*t8*t10*t26*2.0-dQ1*dQ5*m5*t2*t4*t8*t17*t35*2.0-dQ1*dQ5*m5*t3*t4*t7*t17*t35*2.0-dQ1*dQ5*m6*t2*t4*t8*t21*t35*2.0-dQ1*dQ5*m6*t3*t4*t7*t21*t35*2.0+dQ1*dQ5*m6*t2*t4*t8*t22*t35*2.0+dQ1*dQ5*m6*t3*t4*t7*t22*t35*2.0+dQ1*dQ5*m5*t2*t4*t8*t25*t35*2.0;
et340 = dQ1*dQ5*m5*t3*t4*t7*t25*t35*2.0+dQ2*dQ3*m6*t5*t6*t11*t18*t34*4.0+dQ1*dQ5*m6*t2*t4*t8*t26*t35*2.0+dQ1*dQ5*m6*t3*t4*t7*t26*t35*2.0-dQ2*dQ3*m6*t5*t6*t11*t21*t34*4.0-dQ1*dQ2*m5*t2*t8*t17*t34*t35*2.0-dQ1*dQ2*m5*t3*t7*t17*t34*t35*2.0-dQ1*dQ3*m5*t2*t8*t17*t34*t35*2.0-dQ1*dQ3*m5*t3*t7*t17*t34*t35*2.0-dQ1*dQ2*m6*t2*t8*t18*t34*t36*2.0-dQ1*dQ2*m6*t3*t7*t18*t34*t36*2.0-dQ1*dQ3*m6*t2*t8*t18*t34*t36*2.0-dQ1*dQ3*m6*t3*t7*t18*t34*t36*2.0-dQ1*dQ2*m6*t2*t8*t21*t34*t35*2.0-dQ1*dQ2*m6*t3*t7*t21*t34*t35*2.0+dQ1*dQ2*m6*t2*t8*t21*t34*t36*2.0+dQ1*dQ2*m6*t2*t8*t22*t34*t35*2.0+dQ1*dQ2*m6*t3*t7*t21*t34*t36*2.0;
et341 = dQ1*dQ2*m6*t3*t7*t22*t34*t35*2.0-dQ1*dQ3*m6*t2*t8*t21*t34*t35*2.0-dQ1*dQ3*m6*t3*t7*t21*t34*t35*2.0+dQ1*dQ3*m6*t2*t8*t21*t34*t36*2.0+dQ1*dQ3*m6*t2*t8*t22*t34*t35*2.0+dQ1*dQ3*m6*t3*t7*t21*t34*t36*2.0+dQ1*dQ3*m6*t3*t7*t22*t34*t35*2.0+dQ1*dQ2*m5*t2*t8*t25*t34*t35*2.0+dQ1*dQ2*m5*t3*t7*t25*t34*t35*2.0+dQ1*dQ3*m5*t2*t8*t25*t34*t35*2.0+dQ1*dQ3*m5*t3*t7*t25*t34*t35*2.0+dQ2*dQ3*m6*t4*t9*t18*t35*t36*2.0+dQ1*dQ2*m6*t2*t8*t26*t34*t35*2.0+dQ1*dQ2*m6*t3*t7*t26*t34*t35*2.0+dQ1*dQ3*m6*t2*t8*t26*t34*t35*2.0+dQ1*dQ3*m6*t3*t7*t26*t34*t35*2.0-dQ2*dQ3*m6*t4*t9*t21*t35*t36*2.0-Ixx6*dQ1*dQ2*t2*t3*t6*t9*t10*t11*2.0-Ixx6*dQ1*dQ3*t2*t3*t6*t9*t10*t11*2.0;
et342 = Ixx6*dQ1*dQ5*t2*t5*t6*t8*t9*t11*-2.0-Ixx6*dQ1*dQ5*t3*t5*t6*t7*t9*t11*2.0+Ixx6*dQ1*dQ2*t6*t7*t8*t9*t10*t11*2.0+Ixx6*dQ1*dQ3*t6*t7*t8*t9*t10*t11*2.0+Ixx6*dQ1*dQ2*t2*t3*t4*t5*t10*t36*2.0+Ixx6*dQ1*dQ3*t2*t3*t4*t5*t10*t36*2.0-Ixx6*dQ1*dQ2*t4*t5*t7*t8*t10*t36*2.0-Ixx6*dQ1*dQ3*t4*t5*t7*t8*t10*t36*2.0+Iyy6*dQ1*dQ2*t2*t3*t6*t9*t10*t11*2.0+Iyy6*dQ1*dQ3*t2*t3*t6*t9*t10*t11*2.0+Iyy6*dQ1*dQ5*t2*t5*t6*t8*t9*t11*2.0+Iyy6*dQ1*dQ5*t3*t5*t6*t7*t9*t11*2.0-Iyy6*dQ1*dQ2*t6*t7*t8*t9*t10*t11*2.0-Iyy6*dQ1*dQ3*t6*t7*t8*t9*t10*t11*2.0-Iyy6*dQ1*dQ2*t2*t3*t4*t5*t10*t36*2.0-Iyy6*dQ1*dQ3*t2*t3*t4*t5*t10*t36*2.0+Iyy6*dQ1*dQ2*t4*t5*t7*t8*t10*t36*2.0;
et343 = Iyy6*dQ1*dQ3*t4*t5*t7*t8*t10*t36*2.0-dQ1*dQ2*m5*t2*t3*t4*t5*t10*t17*2.0-dQ1*dQ3*m5*t2*t3*t4*t5*t10*t17*2.0-dQ1*dQ2*m6*t2*t3*t4*t5*t10*t21*2.0+dQ1*dQ2*m6*t2*t3*t4*t5*t10*t22*2.0-dQ1*dQ3*m6*t2*t3*t4*t5*t10*t21*2.0+dQ1*dQ3*m6*t2*t3*t4*t5*t10*t22*2.0+dQ1*dQ2*m5*t2*t3*t4*t5*t10*t25*2.0+dQ1*dQ3*m5*t2*t3*t4*t5*t10*t25*2.0+dQ1*dQ2*m5*t4*t5*t7*t8*t10*t17*2.0+dQ1*dQ2*m6*t2*t3*t4*t5*t10*t26*2.0+dQ1*dQ3*m5*t4*t5*t7*t8*t10*t17*2.0+dQ1*dQ3*m6*t2*t3*t4*t5*t10*t26*2.0+dQ1*dQ2*m6*t4*t5*t7*t8*t10*t21*2.0-dQ1*dQ2*m6*t4*t5*t7*t8*t10*t22*2.0+dQ1*dQ3*m6*t4*t5*t7*t8*t10*t21*2.0-dQ1*dQ3*m6*t4*t5*t7*t8*t10*t22*2.0;
et344 = dQ1*dQ2*m5*t4*t5*t7*t8*t10*t25*-2.0-dQ1*dQ3*m5*t4*t5*t7*t8*t10*t25*2.0-dQ1*dQ2*m6*t4*t5*t7*t8*t10*t26*2.0-dQ1*dQ3*m6*t4*t5*t7*t8*t10*t26*2.0-dQ2*dQ6*m6*t5*t6*t9*t10*t11*t18*2.0-dQ3*dQ6*m6*t5*t6*t9*t10*t11*t18*2.0+dQ2*dQ6*m6*t5*t6*t9*t10*t11*t21*2.0+dQ3*dQ6*m6*t5*t6*t9*t10*t11*t21*2.0-dQ1*dQ5*m6*t2*t3*t5*t10*t18*t36*2.0-dQ1*dQ6*m6*t2*t3*t6*t11*t18*t35*2.0+dQ1*dQ5*m6*t2*t3*t5*t10*t21*t36*2.0+dQ1*dQ6*m6*t2*t3*t6*t11*t21*t35*2.0+dQ1*dQ5*m6*t5*t7*t8*t10*t18*t36*2.0+dQ1*dQ6*m6*t2*t8*t9*t10*t18*t36*2.0+dQ1*dQ6*m6*t3*t7*t9*t10*t18*t36*2.0+dQ1*dQ6*m6*t6*t7*t8*t11*t18*t35*2.0-dQ1*dQ5*m6*t5*t7*t8*t10*t21*t36*2.0;
et345 = dQ1*dQ6*m6*t2*t8*t9*t10*t21*t36*-2.0-dQ1*dQ6*m6*t3*t7*t9*t10*t21*t36*2.0-dQ1*dQ6*m6*t6*t7*t8*t11*t21*t35*2.0-dQ1*dQ5*m6*t2*t4*t8*t18*t35*t36*2.0-dQ1*dQ5*m6*t3*t4*t7*t18*t35*t36*2.0+dQ1*dQ5*m6*t2*t4*t8*t21*t35*t36*2.0+dQ1*dQ5*m6*t3*t4*t7*t21*t35*t36*2.0-dQ1*dQ2*m6*t2*t8*t18*t34*t35*t36*2.0-dQ1*dQ2*m6*t3*t7*t18*t34*t35*t36*2.0-dQ1*dQ3*m6*t2*t8*t18*t34*t35*t36*2.0-dQ1*dQ3*m6*t3*t7*t18*t34*t35*t36*2.0+dQ1*dQ2*m6*t2*t8*t21*t34*t35*t36*2.0+dQ1*dQ2*m6*t3*t7*t21*t34*t35*t36*2.0+dQ1*dQ3*m6*t2*t8*t21*t34*t35*t36*2.0+dQ1*dQ3*m6*t3*t7*t21*t34*t35*t36*2.0-Lx3*Lxcm5*dQ1*dQ2*m5*t2*t4*t5*t8*2.0-Lx3*Lxcm5*dQ1*dQ2*m5*t3*t4*t5*t7*2.0;
et346 = Lx3*Lxcm5*dQ1*dQ3*m5*t2*t4*t5*t8*-2.0-Lx3*Lxcm5*dQ1*dQ3*m5*t3*t4*t5*t7*2.0-Lx4*Lxcm5*dQ1*dQ2*m5*t2*t3*t4*t10*2.0-Lx4*Lxcm5*dQ1*dQ3*m5*t2*t3*t4*t10*2.0-Lx2*Lxcm6*dQ1*dQ2*m6*t4*t5*t6*t7*2.0-Lx4*Lxcm5*dQ1*dQ5*m5*t2*t4*t5*t8*2.0-Lx4*Lxcm5*dQ1*dQ5*m5*t3*t4*t5*t7*2.0-Lx4*Lxcm6*dQ1*dQ5*m6*t2*t3*t6*t10*2.0-Lx4*Lxcm6*dQ1*dQ6*m6*t2*t3*t5*t11*2.0+Lx4*Lxcm6*dQ2*dQ3*m6*t4*t5*t6*t9*4.0+Lx4*Lxcm5*dQ1*dQ2*m5*t4*t7*t8*t10*2.0+Lx4*Lxcm5*dQ1*dQ3*m5*t4*t7*t8*t10*2.0+Lx3*Lxcm6*dQ1*dQ2*m6*t2*t8*t9*t11*2.0+Lx3*Lxcm6*dQ1*dQ2*m6*t3*t7*t9*t11*2.0+Lx3*Lxcm6*dQ1*dQ3*m6*t2*t8*t9*t11*2.0+Lx3*Lxcm6*dQ1*dQ3*m6*t3*t7*t9*t11*2.0+Lx4*Lxcm6*dQ1*dQ5*m6*t6*t7*t8*t10*2.0;
et347 = Lx4*Lxcm6*dQ1*dQ6*m6*t5*t7*t8*t11*2.0-Lx4*Lxcm5*dQ1*dQ2*m5*t2*t5*t8*t34*4.0-Lx4*Lxcm5*dQ1*dQ2*m5*t3*t5*t7*t34*4.0-Lx4*Lxcm5*dQ1*dQ3*m5*t2*t5*t8*t34*4.0-Lx4*Lxcm5*dQ1*dQ3*m5*t3*t5*t7*t34*4.0+Lx4*Lycm4*dQ1*dQ2*m4*t2*t4*t8*t9*4.0+Lx4*Lycm4*dQ1*dQ2*m4*t3*t4*t7*t9*4.0+Lx4*Lycm4*dQ1*dQ3*m4*t2*t4*t8*t9*4.0+Lx4*Lycm4*dQ1*dQ3*m4*t3*t4*t7*t9*4.0-Lx4*Lycm6*dQ1*dQ6*m6*t2*t3*t5*t6*2.0+Lx4*Lycm5*dQ1*dQ2*m5*t2*t4*t8*t9*4.0+Lx4*Lycm5*dQ1*dQ2*m5*t3*t4*t7*t9*4.0+Lx4*Lycm5*dQ1*dQ3*m5*t2*t4*t8*t9*4.0+Lx4*Lycm5*dQ1*dQ3*m5*t3*t4*t7*t9*4.0+Lx3*Lycm6*dQ1*dQ2*m6*t2*t6*t8*t9*2.0+Lx3*Lycm6*dQ1*dQ2*m6*t3*t6*t7*t9*2.0+Lx2*Lycm6*dQ1*dQ2*m6*t4*t5*t7*t11*2.0;
et348 = Lx3*Lycm6*dQ1*dQ3*m6*t2*t6*t8*t9*2.0+Lx3*Lycm6*dQ1*dQ3*m6*t3*t6*t7*t9*2.0+Lx4*Lycm6*dQ1*dQ5*m6*t2*t3*t10*t11*2.0+Lx4*Lycm6*dQ1*dQ6*m6*t5*t6*t7*t8*2.0-Lx4*Lycm6*dQ2*dQ3*m6*t4*t5*t9*t11*4.0-Lx4*Lycm6*dQ1*dQ5*m6*t7*t8*t10*t11*2.0+Lxcm4*Lycm4*dQ1*dQ2*m4*t2*t4*t8*t9*4.0+Lxcm4*Lycm4*dQ1*dQ2*m4*t3*t4*t7*t9*4.0+Lxcm4*Lycm4*dQ1*dQ3*m4*t2*t4*t8*t9*4.0+Lxcm4*Lycm4*dQ1*dQ3*m4*t3*t4*t7*t9*4.0+Lxcm5*Lycm5*dQ1*dQ2*m5*t2*t3*t9*t10*2.0+Lxcm5*Lycm5*dQ1*dQ3*m5*t2*t3*t9*t10*2.0+Lxcm5*Lycm5*dQ1*dQ5*m5*t2*t5*t8*t9*2.0+Lxcm5*Lycm5*dQ1*dQ5*m5*t3*t5*t7*t9*2.0-Lxcm6*Lycm6*dQ1*dQ2*m6*t2*t3*t9*t10*2.0-Lxcm6*Lycm6*dQ1*dQ3*m6*t2*t3*t9*t10*2.0-Lxcm6*Lycm6*dQ1*dQ2*m6*t2*t6*t8*t11*4.0;
et349 = Lxcm6*Lycm6*dQ1*dQ2*m6*t3*t6*t7*t11*-4.0-Lxcm6*Lycm6*dQ1*dQ5*m6*t2*t5*t8*t9*2.0-Lxcm6*Lycm6*dQ1*dQ5*m6*t3*t5*t7*t9*2.0-Lxcm6*Lycm6*dQ1*dQ3*m6*t2*t6*t8*t11*4.0-Lxcm6*Lycm6*dQ1*dQ3*m6*t3*t6*t7*t11*4.0-Lxcm5*Lycm5*dQ1*dQ2*m5*t7*t8*t9*t10*2.0-Lxcm5*Lycm5*dQ1*dQ3*m5*t7*t8*t9*t10*2.0-Lxcm6*Lycm6*dQ2*dQ3*m6*t4*t6*t9*t11*4.0+Lxcm6*Lycm6*dQ1*dQ2*m6*t7*t8*t9*t10*2.0+Lxcm6*Lycm6*dQ1*dQ3*m6*t7*t8*t9*t10*2.0-Lxcm6*Lycm6*dQ2*dQ6*m6*t4*t6*t10*t11*4.0-Lxcm6*Lycm6*dQ3*dQ6*m6*t4*t6*t10*t11*4.0+Lxcm6*Lycm6*dQ4*dQ5*m6*t5*t6*t10*t11*4.0-Lxcm6*Lycm6*dQ2*dQ5*m6*t6*t9*t11*t35*4.0-Lxcm6*Lycm6*dQ2*dQ6*m6*t5*t9*t10*t36*4.0-Lxcm6*Lycm6*dQ3*dQ5*m6*t6*t9*t11*t35*4.0;
et350 = Lxcm6*Lycm6*dQ3*dQ6*m6*t5*t9*t10*t36*-4.0-Lxcm6*Lycm6*dQ1*dQ6*m6*t2*t3*t35*t36*4.0+Lxcm6*Lycm6*dQ1*dQ6*m6*t7*t8*t35*t36*4.0+Lx4*Lz6*dQ1*dQ2*m6*t2*t3*t4*t5*2.0+Lx4*Lz6*dQ1*dQ3*m6*t2*t3*t4*t5*2.0-Lx3*Lz6*dQ1*dQ2*m6*t2*t4*t8*t10*2.0-Lx3*Lz6*dQ1*dQ2*m6*t3*t4*t7*t10*2.0-Lx3*Lz6*dQ1*dQ3*m6*t2*t4*t8*t10*2.0-Lx3*Lz6*dQ1*dQ3*m6*t3*t4*t7*t10*2.0-Lx4*Lz6*dQ1*dQ2*m6*t4*t5*t7*t8*2.0-Lx4*Lz6*dQ1*dQ3*m6*t4*t5*t7*t8*2.0-Lx4*Lz6*dQ1*dQ5*m6*t2*t4*t8*t10*2.0-Lx4*Lz6*dQ1*dQ5*m6*t3*t4*t7*t10*2.0-Lx4*Lz6*dQ1*dQ2*m6*t2*t8*t10*t34*4.0-Lx4*Lz6*dQ1*dQ2*m6*t3*t7*t10*t34*4.0-Lx4*Lz6*dQ1*dQ3*m6*t2*t8*t10*t34*4.0;
out1 = ft_4({Ixx5,Ixx6,Iyy5,Iyy6,Izz5,Izz6,Lx2,Lx3,Lx4,Lxcm5,Lxcm6,Lycm5,Lycm6,Lz6,Lzcm5,Lzcm6,dQ1,dQ2,dQ3,dQ4,dQ5,dQ6,et290,et291,et292,et293,et294,et295,et296,et297,et298,et299,et300,et301,et302,et303,et304,et305,et306,et307,et308,et309,et310,et311,et312,et313,et314,et315,et316,et317,et318,et319,et320,et321,et322,et323,et324,et325,et326,et327,et328,et329,et330,et331,et332,et333,et334,et335,et336,et337,et338,et339,et340,et341,et342,et343,et344,et345,et346,et347,et348,et349,et350,m5,m6,t10,t100,t101,t108,t109,t1092,t1093,t11,t112,t113,t115,t116,t117,t118,t1239,t1240,t127,t128,t149,t150,t153,t154,t157,t158,t17,t171,t172,t18,t2,t21,t22,t25,t26,t260,t261,t265,t266,t3,t34,t349,t35,t350,t36,t4,t40,t41,t473,t474,t494,t495,t5,t514,t515,t599,t6,t600,t605,t606,t694,t695,t7,t8,t800,t801,t82,t83,t84,t85,t9,t90,t91,t92,t93,t947,t948,t967,t968,t98,t99});
end
function out1 = ft_4(ct)
[Ixx5,Ixx6,Iyy5,Iyy6,Izz5,Izz6,Lx2,Lx3,Lx4,Lxcm5,Lxcm6,Lycm5,Lycm6,Lz6,Lzcm5,Lzcm6,dQ1,dQ2,dQ3,dQ4,dQ5,dQ6,et290,et291,et292,et293,et294,et295,et296,et297,et298,et299,et300,et301,et302,et303,et304,et305,et306,et307,et308,et309,et310,et311,et312,et313,et314,et315,et316,et317,et318,et319,et320,et321,et322,et323,et324,et325,et326,et327,et328,et329,et330,et331,et332,et333,et334,et335,et336,et337,et338,et339,et340,et341,et342,et343,et344,et345,et346,et347,et348,et349,et350,m5,m6,t10,t100,t101,t108,t109,t1092,t1093,t11,t112,t113,t115,t116,t117,t118,t1239,t1240,t127,t128,t149,t150,t153,t154,t157,t158,t17,t171,t172,t18,t2,t21,t22,t25,t26,t260,t261,t265,t266,t3,t34,t349,t35,t350,t36,t4,t40,t41,t473,t474,t494,t495,t5,t514,t515,t599,t6,t600,t605,t606,t694,t695,t7,t8,t800,t801,t82,t83,t84,t85,t9,t90,t91,t92,t93,t947,t948,t967,t968,t98,t99] = ct{:};
et351 = Lx4*Lz6*dQ1*dQ3*m6*t3*t7*t10*t34*-4.0+Lx4*Lzcm5*dQ1*dQ2*m5*t2*t3*t4*t5*2.0+Lx4*Lzcm5*dQ1*dQ3*m5*t2*t3*t4*t5*2.0+Lx4*Lzcm6*dQ1*dQ2*m6*t2*t3*t4*t5*2.0+Lx4*Lzcm6*dQ1*dQ3*m6*t2*t3*t4*t5*2.0-Lxcm6*Lz6*dQ1*dQ2*m6*t2*t3*t4*t6*2.0-Lxcm6*Lz6*dQ1*dQ3*m6*t2*t3*t4*t6*2.0-Lx3*Lzcm5*dQ1*dQ2*m5*t2*t4*t8*t10*2.0-Lx3*Lzcm5*dQ1*dQ2*m5*t3*t4*t7*t10*2.0-Lx3*Lzcm5*dQ1*dQ3*m5*t2*t4*t8*t10*2.0-Lx3*Lzcm5*dQ1*dQ3*m5*t3*t4*t7*t10*2.0-Lx4*Lzcm5*dQ1*dQ2*m5*t4*t5*t7*t8*2.0-Lx3*Lzcm6*dQ1*dQ2*m6*t2*t4*t8*t10*2.0-Lx3*Lzcm6*dQ1*dQ2*m6*t3*t4*t7*t10*2.0-Lx4*Lzcm5*dQ1*dQ3*m5*t4*t5*t7*t8*2.0-Lx3*Lzcm6*dQ1*dQ3*m6*t2*t4*t8*t10*2.0-Lx3*Lzcm6*dQ1*dQ3*m6*t3*t4*t7*t10*2.0;
et352 = Lx4*Lzcm6*dQ1*dQ2*m6*t4*t5*t7*t8*-2.0-Lx4*Lzcm5*dQ1*dQ5*m5*t2*t4*t8*t10*2.0-Lx4*Lzcm5*dQ1*dQ5*m5*t3*t4*t7*t10*2.0-Lx4*Lzcm6*dQ1*dQ3*m6*t4*t5*t7*t8*2.0-Lx4*Lzcm6*dQ1*dQ5*m6*t2*t4*t8*t10*2.0-Lx4*Lzcm6*dQ1*dQ5*m6*t3*t4*t7*t10*2.0+Lxcm6*Lz6*dQ1*dQ2*m6*t4*t6*t7*t8*2.0+Lxcm6*Lz6*dQ1*dQ3*m6*t4*t6*t7*t8*2.0+Lxcm6*Lz6*dQ1*dQ6*m6*t2*t4*t8*t11*2.0+Lxcm6*Lz6*dQ1*dQ6*m6*t3*t4*t7*t11*2.0+Lxcm6*Lz6*dQ2*dQ5*m6*t5*t6*t9*t10*4.0+Lxcm6*Lz6*dQ3*dQ5*m6*t5*t6*t9*t10*4.0+Lxcm6*Lz6*dQ1*dQ5*m6*t2*t3*t6*t35*4.0-Lx4*Lzcm5*dQ1*dQ2*m5*t2*t8*t10*t34*4.0-Lx4*Lzcm5*dQ1*dQ2*m5*t3*t7*t10*t34*4.0-Lx4*Lzcm5*dQ1*dQ3*m5*t2*t8*t10*t34*4.0-Lx4*Lzcm5*dQ1*dQ3*m5*t3*t7*t10*t34*4.0;
et353 = Lx4*Lzcm6*dQ1*dQ2*m6*t2*t8*t10*t34*-4.0-Lx4*Lzcm6*dQ1*dQ2*m6*t3*t7*t10*t34*4.0-Lx4*Lzcm6*dQ1*dQ3*m6*t2*t8*t10*t34*4.0-Lx4*Lzcm6*dQ1*dQ3*m6*t3*t7*t10*t34*4.0-Lxcm6*Lz6*dQ1*dQ5*m6*t6*t7*t8*t35*4.0-Lxcm6*Lzcm6*dQ1*dQ2*m6*t2*t3*t4*t6*2.0-Lxcm6*Lzcm6*dQ1*dQ3*m6*t2*t3*t4*t6*2.0+Lxcm6*Lzcm6*dQ1*dQ2*m6*t4*t6*t7*t8*2.0+Lxcm6*Lzcm6*dQ1*dQ3*m6*t4*t6*t7*t8*2.0+Lxcm5*Lzcm5*dQ2*dQ3*m5*t4*t5*t9*t10*4.0+Lxcm6*Lzcm6*dQ1*dQ6*m6*t2*t4*t8*t11*2.0+Lxcm6*Lzcm6*dQ1*dQ6*m6*t3*t4*t7*t11*2.0+Lxcm6*Lzcm6*dQ2*dQ5*m6*t5*t6*t9*t10*4.0+Lxcm6*Lzcm6*dQ3*dQ5*m6*t5*t6*t9*t10*4.0+Lxcm5*Lzcm5*dQ1*dQ2*m5*t2*t3*t4*t35*4.0+Lxcm5*Lzcm5*dQ1*dQ3*m5*t2*t3*t4*t35*4.0+Lxcm6*Lzcm6*dQ1*dQ5*m6*t2*t3*t6*t35*4.0;
et354 = Lxcm5*Lzcm5*dQ1*dQ2*m5*t4*t7*t8*t35*-4.0-Lxcm5*Lzcm5*dQ1*dQ3*m5*t4*t7*t8*t35*4.0-Lxcm6*Lzcm6*dQ1*dQ5*m6*t6*t7*t8*t35*4.0+Lycm6*Lz6*dQ1*dQ2*m6*t2*t3*t4*t11*2.0+Lycm6*Lz6*dQ1*dQ3*m6*t2*t3*t4*t11*2.0+Lycm6*Lz6*dQ1*dQ6*m6*t2*t4*t6*t8*2.0+Lycm6*Lz6*dQ1*dQ6*m6*t3*t4*t6*t7*2.0-Lycm6*Lz6*dQ1*dQ2*m6*t4*t7*t8*t11*2.0-Lycm6*Lz6*dQ1*dQ3*m6*t4*t7*t8*t11*2.0-Lycm6*Lz6*dQ2*dQ5*m6*t5*t9*t10*t11*4.0-Lycm6*Lz6*dQ3*dQ5*m6*t5*t9*t10*t11*4.0-Lycm6*Lz6*dQ1*dQ5*m6*t2*t3*t11*t35*4.0+Lycm6*Lz6*dQ1*dQ5*m6*t7*t8*t11*t35*4.0-Lycm5*Lzcm5*dQ1*dQ2*m5*t2*t3*t5*t9*2.0-Lycm5*Lzcm5*dQ1*dQ3*m5*t2*t3*t5*t9*2.0+Lycm6*Lzcm6*dQ1*dQ2*m6*t2*t3*t4*t11*2.0+Lycm6*Lzcm6*dQ1*dQ3*m6*t2*t3*t4*t11*2.0;
et355 = Lycm6*Lzcm6*dQ1*dQ6*m6*t2*t4*t6*t8*2.0+Lycm6*Lzcm6*dQ1*dQ6*m6*t3*t4*t6*t7*2.0+Lycm5*Lzcm5*dQ1*dQ2*m5*t5*t7*t8*t9*2.0+Lycm5*Lzcm5*dQ1*dQ3*m5*t5*t7*t8*t9*2.0+Lycm5*Lzcm5*dQ1*dQ5*m5*t2*t8*t9*t10*2.0+Lycm5*Lzcm5*dQ1*dQ5*m5*t3*t7*t9*t10*2.0-Lycm6*Lzcm6*dQ1*dQ2*m6*t4*t7*t8*t11*2.0-Lycm6*Lzcm6*dQ1*dQ3*m6*t4*t7*t8*t11*2.0-Lycm6*Lzcm6*dQ2*dQ5*m6*t5*t9*t10*t11*4.0-Lycm6*Lzcm6*dQ3*dQ5*m6*t5*t9*t10*t11*4.0-Lycm6*Lzcm6*dQ1*dQ5*m6*t2*t3*t11*t35*4.0+Lycm6*Lzcm6*dQ1*dQ5*m6*t7*t8*t11*t35*4.0+Lz6*Lzcm6*dQ1*dQ5*m6*t2*t3*t5*t10*4.0-Lz6*Lzcm6*dQ1*dQ5*m6*t5*t7*t8*t10*4.0+Lz6*Lzcm6*dQ1*dQ5*m6*t2*t4*t8*t35*4.0+Lz6*Lzcm6*dQ1*dQ5*m6*t3*t4*t7*t35*4.0+Lz6*Lzcm6*dQ1*dQ2*m6*t2*t8*t34*t35*4.0;
et356 = Lz6*Lzcm6*dQ1*dQ2*m6*t3*t7*t34*t35*4.0+Lz6*Lzcm6*dQ1*dQ3*m6*t2*t8*t34*t35*4.0+Lz6*Lzcm6*dQ1*dQ3*m6*t3*t7*t34*t35*4.0-Lx3*Lxcm6*dQ1*dQ2*m6*t2*t4*t5*t6*t8*2.0-Lx3*Lxcm6*dQ1*dQ2*m6*t3*t4*t5*t6*t7*2.0-Lx3*Lxcm6*dQ1*dQ3*m6*t2*t4*t5*t6*t8*2.0-Lx3*Lxcm6*dQ1*dQ3*m6*t3*t4*t5*t6*t7*2.0-Lx4*Lxcm6*dQ1*dQ2*m6*t2*t3*t4*t6*t10*2.0-Lx4*Lxcm6*dQ1*dQ3*m6*t2*t3*t4*t6*t10*2.0-Lx4*Lxcm6*dQ1*dQ5*m6*t2*t4*t5*t6*t8*2.0-Lx4*Lxcm6*dQ1*dQ5*m6*t3*t4*t5*t6*t7*2.0+Lx4*Lxcm6*dQ1*dQ2*m6*t2*t4*t8*t9*t11*4.0+Lx4*Lxcm6*dQ1*dQ2*m6*t3*t4*t7*t9*t11*4.0+Lx4*Lxcm6*dQ1*dQ2*m6*t4*t6*t7*t8*t10*2.0+Lx4*Lxcm6*dQ1*dQ3*m6*t2*t4*t8*t9*t11*4.0+Lx4*Lxcm6*dQ1*dQ3*m6*t3*t4*t7*t9*t11*4.0;
et357 = Lx4*Lxcm6*dQ1*dQ3*m6*t4*t6*t7*t8*t10*2.0+Lx4*Lxcm6*dQ1*dQ6*m6*t2*t4*t8*t10*t11*2.0+Lx4*Lxcm6*dQ1*dQ6*m6*t3*t4*t7*t10*t11*2.0-Lx4*Lxcm6*dQ1*dQ2*m6*t2*t5*t6*t8*t34*4.0-Lx4*Lxcm6*dQ1*dQ2*m6*t3*t5*t6*t7*t34*4.0-Lx4*Lxcm6*dQ1*dQ3*m6*t2*t5*t6*t8*t34*4.0-Lx4*Lxcm6*dQ1*dQ3*m6*t3*t5*t6*t7*t34*4.0+Lx3*Lycm6*dQ1*dQ2*m6*t2*t4*t5*t8*t11*2.0+Lx3*Lycm6*dQ1*dQ2*m6*t3*t4*t5*t7*t11*2.0+Lx4*Lycm6*dQ1*dQ2*m6*t2*t4*t6*t8*t9*4.0+Lx4*Lycm6*dQ1*dQ2*m6*t3*t4*t6*t7*t9*4.0+Lx3*Lycm6*dQ1*dQ3*m6*t2*t4*t5*t8*t11*2.0+Lx3*Lycm6*dQ1*dQ3*m6*t3*t4*t5*t7*t11*2.0+Lx4*Lycm6*dQ1*dQ2*m6*t2*t3*t4*t10*t11*2.0+Lx4*Lycm6*dQ1*dQ3*m6*t2*t4*t6*t8*t9*4.0+Lx4*Lycm6*dQ1*dQ3*m6*t3*t4*t6*t7*t9*4.0;
et358 = Lx4*Lycm6*dQ1*dQ3*m6*t2*t3*t4*t10*t11*2.0+Lx4*Lycm6*dQ1*dQ5*m6*t2*t4*t5*t8*t11*2.0+Lx4*Lycm6*dQ1*dQ5*m6*t3*t4*t5*t7*t11*2.0+Lx4*Lycm6*dQ1*dQ6*m6*t2*t4*t6*t8*t10*2.0+Lx4*Lycm6*dQ1*dQ6*m6*t3*t4*t6*t7*t10*2.0-Lx4*Lycm6*dQ1*dQ2*m6*t4*t7*t8*t10*t11*2.0-Lx4*Lycm6*dQ1*dQ3*m6*t4*t7*t8*t10*t11*2.0+Lx4*Lycm6*dQ1*dQ2*m6*t2*t5*t8*t11*t34*4.0+Lx4*Lycm6*dQ1*dQ2*m6*t3*t5*t7*t11*t34*4.0+Lx4*Lycm6*dQ1*dQ3*m6*t2*t5*t8*t11*t34*4.0+Lx4*Lycm6*dQ1*dQ3*m6*t3*t5*t7*t11*t34*4.0+Lxcm5*Lycm5*dQ1*dQ2*m5*t2*t4*t5*t8*t9*4.0+Lxcm5*Lycm5*dQ1*dQ2*m5*t3*t4*t5*t7*t9*4.0+Lxcm5*Lycm5*dQ1*dQ3*m5*t2*t4*t5*t8*t9*4.0+Lxcm5*Lycm5*dQ1*dQ3*m5*t3*t4*t5*t7*t9*4.0-Lxcm6*Lycm6*dQ1*dQ2*m6*t2*t4*t5*t8*t9*4.0;
et359 = Lxcm6*Lycm6*dQ1*dQ2*m6*t3*t4*t5*t7*t9*-4.0-Lxcm6*Lycm6*dQ1*dQ3*m6*t2*t4*t5*t8*t9*4.0-Lxcm6*Lycm6*dQ1*dQ3*m6*t3*t4*t5*t7*t9*4.0-Lxcm6*Lycm6*dQ1*dQ6*m6*t2*t4*t5*t8*t10*2.0-Lxcm6*Lycm6*dQ1*dQ6*m6*t3*t4*t5*t7*t10*2.0+Lxcm6*Lycm6*dQ1*dQ2*m6*t2*t3*t9*t10*t36*4.0+Lxcm6*Lycm6*dQ1*dQ2*m6*t2*t6*t8*t11*t34*4.0+Lxcm6*Lycm6*dQ1*dQ2*m6*t3*t6*t7*t11*t34*4.0+Lxcm6*Lycm6*dQ1*dQ3*m6*t2*t3*t9*t10*t36*4.0+Lxcm6*Lycm6*dQ1*dQ3*m6*t2*t6*t8*t11*t34*4.0+Lxcm6*Lycm6*dQ1*dQ3*m6*t3*t6*t7*t11*t34*4.0+Lxcm6*Lycm6*dQ1*dQ5*m6*t2*t5*t8*t9*t36*4.0+Lxcm6*Lycm6*dQ1*dQ5*m6*t3*t5*t7*t9*t36*4.0-Lxcm6*Lycm6*dQ2*dQ3*m6*t4*t6*t9*t11*t35*4.0-Lxcm6*Lycm6*dQ1*dQ2*m6*t7*t8*t9*t10*t36*4.0-Lxcm6*Lycm6*dQ1*dQ3*m6*t7*t8*t9*t10*t36*4.0;
et360 = Lxcm6*Lz6*dQ1*dQ2*m6*t2*t3*t5*t9*t11*-2.0-Lxcm6*Lz6*dQ1*dQ3*m6*t2*t3*t5*t9*t11*2.0-Lxcm6*Lz6*dQ1*dQ6*m6*t2*t3*t5*t10*t11*2.0+Lxcm6*Lz6*dQ2*dQ3*m6*t4*t5*t6*t9*t10*4.0+Lxcm6*Lz6*dQ1*dQ2*m6*t5*t7*t8*t9*t11*2.0+Lxcm6*Lz6*dQ1*dQ3*m6*t5*t7*t8*t9*t11*2.0+Lxcm6*Lz6*dQ1*dQ5*m6*t2*t8*t9*t10*t11*2.0+Lxcm6*Lz6*dQ1*dQ5*m6*t3*t7*t9*t10*t11*2.0+Lxcm6*Lz6*dQ1*dQ6*m6*t5*t7*t8*t10*t11*2.0+Lxcm6*Lz6*dQ1*dQ2*m6*t2*t3*t4*t6*t35*4.0+Lxcm6*Lz6*dQ1*dQ3*m6*t2*t3*t4*t6*t35*4.0-Lxcm6*Lz6*dQ1*dQ2*m6*t4*t6*t7*t8*t35*4.0-Lxcm6*Lz6*dQ1*dQ3*m6*t4*t6*t7*t8*t35*4.0-Lxcm6*Lz6*dQ1*dQ6*m6*t2*t4*t8*t11*t35*2.0-Lxcm6*Lz6*dQ1*dQ6*m6*t3*t4*t7*t11*t35*2.0-Lxcm5*Lzcm5*dQ1*dQ5*m5*t2*t4*t5*t8*t10*4.0;
et361 = Lxcm5*Lzcm5*dQ1*dQ5*m5*t3*t4*t5*t7*t10*-4.0-Lxcm6*Lzcm6*dQ1*dQ2*m6*t2*t3*t5*t9*t11*2.0-Lxcm6*Lzcm6*dQ1*dQ3*m6*t2*t3*t5*t9*t11*2.0-Lxcm6*Lzcm6*dQ1*dQ6*m6*t2*t3*t5*t10*t11*2.0+Lxcm6*Lzcm6*dQ2*dQ3*m6*t4*t5*t6*t9*t10*4.0+Lxcm6*Lzcm6*dQ1*dQ2*m6*t5*t7*t8*t9*t11*2.0+Lxcm6*Lzcm6*dQ1*dQ3*m6*t5*t7*t8*t9*t11*2.0+Lxcm6*Lzcm6*dQ1*dQ5*m6*t2*t8*t9*t10*t11*2.0+Lxcm6*Lzcm6*dQ1*dQ5*m6*t3*t7*t9*t10*t11*2.0+Lxcm6*Lzcm6*dQ1*dQ6*m6*t5*t7*t8*t10*t11*2.0+Lxcm6*Lzcm6*dQ1*dQ2*m6*t2*t3*t4*t6*t35*4.0+Lxcm6*Lzcm6*dQ1*dQ3*m6*t2*t3*t4*t6*t35*4.0-Lxcm5*Lzcm5*dQ1*dQ2*m5*t2*t5*t8*t10*t34*4.0-Lxcm5*Lzcm5*dQ1*dQ2*m5*t3*t5*t7*t10*t34*4.0-Lxcm5*Lzcm5*dQ1*dQ3*m5*t2*t5*t8*t10*t34*4.0-Lxcm5*Lzcm5*dQ1*dQ3*m5*t3*t5*t7*t10*t34*4.0;
et362 = Lxcm6*Lzcm6*dQ1*dQ2*m6*t4*t6*t7*t8*t35*-4.0-Lxcm6*Lzcm6*dQ1*dQ3*m6*t4*t6*t7*t8*t35*4.0-Lxcm6*Lzcm6*dQ1*dQ6*m6*t2*t4*t8*t11*t35*2.0-Lxcm6*Lzcm6*dQ1*dQ6*m6*t3*t4*t7*t11*t35*2.0-Lycm6*Lz6*dQ1*dQ2*m6*t2*t3*t5*t6*t9*2.0-Lycm6*Lz6*dQ1*dQ3*m6*t2*t3*t5*t6*t9*2.0-Lycm6*Lz6*dQ1*dQ6*m6*t2*t3*t5*t6*t10*2.0+Lycm6*Lz6*dQ1*dQ2*m6*t5*t6*t7*t8*t9*2.0+Lycm6*Lz6*dQ1*dQ3*m6*t5*t6*t7*t8*t9*2.0+Lycm6*Lz6*dQ1*dQ5*m6*t2*t6*t8*t9*t10*2.0+Lycm6*Lz6*dQ1*dQ5*m6*t3*t6*t7*t9*t10*2.0+Lycm6*Lz6*dQ1*dQ6*m6*t5*t6*t7*t8*t10*2.0-Lycm6*Lz6*dQ2*dQ3*m6*t4*t5*t9*t10*t11*4.0-Lycm6*Lz6*dQ1*dQ2*m6*t2*t3*t4*t11*t35*4.0-Lycm6*Lz6*dQ1*dQ3*m6*t2*t3*t4*t11*t35*4.0;
et363 = Lycm6*Lz6*dQ1*dQ6*m6*t2*t4*t6*t8*t35*-2.0-Lycm6*Lz6*dQ1*dQ6*m6*t3*t4*t6*t7*t35*2.0+Lycm6*Lz6*dQ1*dQ2*m6*t4*t7*t8*t11*t35*4.0+Lycm6*Lz6*dQ1*dQ3*m6*t4*t7*t8*t11*t35*4.0-Lycm6*Lzcm6*dQ1*dQ2*m6*t2*t3*t5*t6*t9*2.0-Lycm6*Lzcm6*dQ1*dQ3*m6*t2*t3*t5*t6*t9*2.0+Lycm5*Lzcm5*dQ1*dQ2*m5*t2*t4*t8*t9*t10*4.0+Lycm5*Lzcm5*dQ1*dQ2*m5*t3*t4*t7*t9*t10*4.0-Lycm6*Lzcm6*dQ1*dQ6*m6*t2*t3*t5*t6*t10*2.0+Lycm5*Lzcm5*dQ1*dQ3*m5*t2*t4*t8*t9*t10*4.0+Lycm5*Lzcm5*dQ1*dQ3*m5*t3*t4*t7*t9*t10*4.0+Lycm6*Lzcm6*dQ1*dQ2*m6*t5*t6*t7*t8*t9*2.0+Lycm6*Lzcm6*dQ1*dQ3*m6*t5*t6*t7*t8*t9*2.0+Lycm6*Lzcm6*dQ1*dQ5*m6*t2*t6*t8*t9*t10*2.0+Lycm6*Lzcm6*dQ1*dQ5*m6*t3*t6*t7*t9*t10*2.0+Lycm6*Lzcm6*dQ1*dQ6*m6*t5*t6*t7*t8*t10*2.0;
et364 = Lycm6*Lzcm6*dQ2*dQ3*m6*t4*t5*t9*t10*t11*-4.0-Lycm6*Lzcm6*dQ1*dQ2*m6*t2*t3*t4*t11*t35*4.0-Lycm6*Lzcm6*dQ1*dQ3*m6*t2*t3*t4*t11*t35*4.0-Lycm6*Lzcm6*dQ1*dQ6*m6*t2*t4*t6*t8*t35*2.0-Lycm6*Lzcm6*dQ1*dQ6*m6*t3*t4*t6*t7*t35*2.0+Lycm6*Lzcm6*dQ1*dQ2*m6*t4*t7*t8*t11*t35*4.0+Lycm6*Lzcm6*dQ1*dQ3*m6*t4*t7*t8*t11*t35*4.0+Lz6*Lzcm6*dQ1*dQ2*m6*t2*t3*t4*t5*t10*4.0+Lz6*Lzcm6*dQ1*dQ3*m6*t2*t3*t4*t5*t10*4.0-Lz6*Lzcm6*dQ1*dQ2*m6*t4*t5*t7*t8*t10*4.0-Lz6*Lzcm6*dQ1*dQ3*m6*t4*t5*t7*t8*t10*4.0-Ixx6*dQ1*dQ2*t2*t4*t5*t6*t8*t9*t11*4.0-Ixx6*dQ1*dQ2*t3*t4*t5*t6*t7*t9*t11*4.0-Ixx6*dQ1*dQ3*t2*t4*t5*t6*t8*t9*t11*4.0-Ixx6*dQ1*dQ3*t3*t4*t5*t6*t7*t9*t11*4.0;
et365 = Iyy6*dQ1*dQ2*t2*t4*t5*t6*t8*t9*t11*4.0+Iyy6*dQ1*dQ2*t3*t4*t5*t6*t7*t9*t11*4.0+Iyy6*dQ1*dQ3*t2*t4*t5*t6*t8*t9*t11*4.0+Iyy6*dQ1*dQ3*t3*t4*t5*t6*t7*t9*t11*4.0+dQ1*dQ2*m6*t2*t3*t6*t9*t10*t11*t18*2.0+dQ1*dQ3*m6*t2*t3*t6*t9*t10*t11*t18*2.0-dQ1*dQ2*m6*t2*t3*t6*t9*t10*t11*t21*2.0+dQ1*dQ5*m6*t2*t5*t6*t8*t9*t11*t18*2.0+dQ1*dQ5*m6*t3*t5*t6*t7*t9*t11*t18*2.0-dQ1*dQ3*m6*t2*t3*t6*t9*t10*t11*t21*2.0-dQ1*dQ5*m6*t2*t5*t6*t8*t9*t11*t21*2.0-dQ1*dQ5*m6*t3*t5*t6*t7*t9*t11*t21*2.0-dQ1*dQ2*m6*t6*t7*t8*t9*t10*t11*t18*2.0-dQ1*dQ3*m6*t6*t7*t8*t9*t10*t11*t18*2.0+dQ1*dQ2*m6*t6*t7*t8*t9*t10*t11*t21*2.0+dQ1*dQ3*m6*t6*t7*t8*t9*t10*t11*t21*2.0;
et366 = dQ1*dQ2*m6*t2*t3*t4*t5*t10*t18*t36*-2.0-dQ1*dQ3*m6*t2*t3*t4*t5*t10*t18*t36*2.0+dQ1*dQ2*m6*t2*t3*t4*t5*t10*t21*t36*2.0+dQ1*dQ3*m6*t2*t3*t4*t5*t10*t21*t36*2.0+dQ1*dQ2*m6*t4*t5*t7*t8*t10*t18*t36*2.0+dQ1*dQ3*m6*t4*t5*t7*t8*t10*t18*t36*2.0-dQ1*dQ2*m6*t4*t5*t7*t8*t10*t21*t36*2.0-dQ1*dQ3*m6*t4*t5*t7*t8*t10*t21*t36*2.0+dQ1*dQ2*m6*t2*t4*t5*t6*t8*t9*t11*t18*4.0+dQ1*dQ2*m6*t3*t4*t5*t6*t7*t9*t11*t18*4.0+dQ1*dQ3*m6*t2*t4*t5*t6*t8*t9*t11*t18*4.0+dQ1*dQ3*m6*t3*t4*t5*t6*t7*t9*t11*t18*4.0-dQ1*dQ2*m6*t2*t4*t5*t6*t8*t9*t11*t21*4.0-dQ1*dQ2*m6*t3*t4*t5*t6*t7*t9*t11*t21*4.0-dQ1*dQ3*m6*t2*t4*t5*t6*t8*t9*t11*t21*4.0;
et367 = dQ1*dQ3*m6*t3*t4*t5*t6*t7*t9*t11*t21*-4.0-dQ1*dQ6*m6*t2*t4*t5*t6*t8*t10*t11*t21*2.0-dQ1*dQ6*m6*t3*t4*t5*t6*t7*t10*t11*t21*2.0+Lxcm6*Lycm6*dQ1*dQ5*m6*t2*t3*t5*t6*t10*t11*4.0-Lxcm6*Lycm6*dQ1*dQ5*m6*t5*t6*t7*t8*t10*t11*4.0-Lxcm6*Lycm6*dQ1*dQ6*m6*t2*t6*t8*t9*t10*t11*4.0-Lxcm6*Lycm6*dQ1*dQ6*m6*t3*t6*t7*t9*t10*t11*4.0+Lxcm6*Lycm6*dQ1*dQ2*m6*t2*t4*t5*t8*t9*t36*8.0+Lxcm6*Lycm6*dQ1*dQ2*m6*t3*t4*t5*t7*t9*t36*8.0+Lxcm6*Lycm6*dQ1*dQ3*m6*t2*t4*t5*t8*t9*t36*8.0+Lxcm6*Lycm6*dQ1*dQ3*m6*t3*t4*t5*t7*t9*t36*8.0+Lxcm6*Lycm6*dQ1*dQ5*m6*t2*t4*t6*t8*t11*t35*4.0+Lxcm6*Lycm6*dQ1*dQ5*m6*t3*t4*t6*t7*t11*t35*4.0+Lxcm6*Lycm6*dQ1*dQ6*m6*t2*t4*t5*t8*t10*t36*4.0;
et368 = Lxcm6*Lycm6*dQ1*dQ6*m6*t3*t4*t5*t7*t10*t36*4.0+Lxcm6*Lycm6*dQ1*dQ2*m6*t2*t6*t8*t11*t34*t35*4.0+Lxcm6*Lycm6*dQ1*dQ2*m6*t3*t6*t7*t11*t34*t35*4.0+Lxcm6*Lycm6*dQ1*dQ3*m6*t2*t6*t8*t11*t34*t35*4.0+Lxcm6*Lycm6*dQ1*dQ3*m6*t3*t6*t7*t11*t34*t35*4.0-Lxcm6*Lz6*dQ1*dQ5*m6*t2*t4*t5*t6*t8*t10*4.0-Lxcm6*Lz6*dQ1*dQ5*m6*t3*t4*t5*t6*t7*t10*4.0+Lxcm6*Lz6*dQ1*dQ2*m6*t2*t4*t8*t9*t10*t11*4.0+Lxcm6*Lz6*dQ1*dQ2*m6*t3*t4*t7*t9*t10*t11*4.0+Lxcm6*Lz6*dQ1*dQ3*m6*t2*t4*t8*t9*t10*t11*4.0+Lxcm6*Lz6*dQ1*dQ3*m6*t3*t4*t7*t9*t10*t11*4.0-Lxcm6*Lz6*dQ1*dQ2*m6*t2*t5*t6*t8*t10*t34*4.0-Lxcm6*Lz6*dQ1*dQ2*m6*t3*t5*t6*t7*t10*t34*4.0-Lxcm6*Lz6*dQ1*dQ3*m6*t2*t5*t6*t8*t10*t34*4.0;
et369 = Lxcm6*Lz6*dQ1*dQ3*m6*t3*t5*t6*t7*t10*t34*-4.0-Lxcm6*Lzcm6*dQ1*dQ5*m6*t2*t4*t5*t6*t8*t10*4.0-Lxcm6*Lzcm6*dQ1*dQ5*m6*t3*t4*t5*t6*t7*t10*4.0+Lxcm6*Lzcm6*dQ1*dQ2*m6*t2*t4*t8*t9*t10*t11*4.0+Lxcm6*Lzcm6*dQ1*dQ2*m6*t3*t4*t7*t9*t10*t11*4.0+Lxcm6*Lzcm6*dQ1*dQ3*m6*t2*t4*t8*t9*t10*t11*4.0+Lxcm6*Lzcm6*dQ1*dQ3*m6*t3*t4*t7*t9*t10*t11*4.0-Lxcm6*Lzcm6*dQ1*dQ2*m6*t2*t5*t6*t8*t10*t34*4.0-Lxcm6*Lzcm6*dQ1*dQ2*m6*t3*t5*t6*t7*t10*t34*4.0-Lxcm6*Lzcm6*dQ1*dQ3*m6*t2*t5*t6*t8*t10*t34*4.0-Lxcm6*Lzcm6*dQ1*dQ3*m6*t3*t5*t6*t7*t10*t34*4.0+Lycm6*Lz6*dQ1*dQ2*m6*t2*t4*t6*t8*t9*t10*4.0+Lycm6*Lz6*dQ1*dQ2*m6*t3*t4*t6*t7*t9*t10*4.0+Lycm6*Lz6*dQ1*dQ3*m6*t2*t4*t6*t8*t9*t10*4.0;
et370 = Lycm6*Lz6*dQ1*dQ3*m6*t3*t4*t6*t7*t9*t10*4.0+Lycm6*Lz6*dQ1*dQ5*m6*t2*t4*t5*t8*t10*t11*4.0+Lycm6*Lz6*dQ1*dQ5*m6*t3*t4*t5*t7*t10*t11*4.0+Lycm6*Lz6*dQ1*dQ2*m6*t2*t5*t8*t10*t11*t34*4.0+Lycm6*Lz6*dQ1*dQ2*m6*t3*t5*t7*t10*t11*t34*4.0+Lycm6*Lz6*dQ1*dQ3*m6*t2*t5*t8*t10*t11*t34*4.0+Lycm6*Lz6*dQ1*dQ3*m6*t3*t5*t7*t10*t11*t34*4.0+Lycm6*Lzcm6*dQ1*dQ2*m6*t2*t4*t6*t8*t9*t10*4.0+Lycm6*Lzcm6*dQ1*dQ2*m6*t3*t4*t6*t7*t9*t10*4.0+Lycm6*Lzcm6*dQ1*dQ3*m6*t2*t4*t6*t8*t9*t10*4.0+Lycm6*Lzcm6*dQ1*dQ3*m6*t3*t4*t6*t7*t9*t10*4.0+Lycm6*Lzcm6*dQ1*dQ5*m6*t2*t4*t5*t8*t10*t11*4.0+Lycm6*Lzcm6*dQ1*dQ5*m6*t3*t4*t5*t7*t10*t11*4.0+Lycm6*Lzcm6*dQ1*dQ2*m6*t2*t5*t8*t10*t11*t34*4.0+Lycm6*Lzcm6*dQ1*dQ2*m6*t3*t5*t7*t10*t11*t34*4.0;
et371 = Lycm6*Lzcm6*dQ1*dQ3*m6*t2*t5*t8*t10*t11*t34*4.0+Lycm6*Lzcm6*dQ1*dQ3*m6*t3*t5*t7*t10*t11*t34*4.0+Lxcm6*Lycm6*dQ1*dQ2*m6*t2*t3*t4*t5*t6*t10*t11*4.0+Lxcm6*Lycm6*dQ1*dQ3*m6*t2*t3*t4*t5*t6*t10*t11*4.0-Lxcm6*Lycm6*dQ1*dQ2*m6*t4*t5*t6*t7*t8*t10*t11*4.0-Lxcm6*Lycm6*dQ1*dQ3*m6*t4*t5*t6*t7*t8*t10*t11*4.0;
et372 = t4*t82+t4*t83+t4*t84+t4*t85+t4*t90+t4*t91+t4*t92+t4*t93-t4*t98-t4*t99-t4*t100-t4*t101+t4*t112+t4*t113+t4*t149+t4*t150-t4*t153-t4*t154+t4*t157+t4*t158+t4*t260+t4*t261+t4*t605+t4*t606+t4*t800+t4*t801+t4*t1239+t4*t1240-t4*t35*t82*2.0-t4*t35*t83*2.0-t4*t35*t92*2.0-t4*t35*t93*2.0+t4*t35*t98*2.0+t4*t35*t99*2.0+t4*t35*t100*2.0+t4*t35*t101*2.0-t4*t36*t149*2.0-t4*t36*t150*2.0+t4*t35*t514+t4*t35*t515+t4*t35*t947+t4*t35*t948-t4*t35*t36*t84*2.0-t4*t35*t36*t85*2.0-Ixx5*dQ2*dQ4*t9-Ixx5*dQ3*dQ4*t9;
et373 = -Ixx6*dQ2*dQ4*t9-Ixx6*dQ3*dQ4*t9+Ixx6*dQ4*dQ6*t10+Ixx5*dQ2*dQ3*t40+Ixx6*dQ5*dQ6*t41-Iyy5*dQ2*dQ4*t9-Iyy5*dQ3*dQ4*t9-Iyy6*dQ2*dQ4*t9-Iyy6*dQ3*dQ4*t9-Iyy6*dQ4*dQ6*t10+Iyy6*dQ2*dQ3*t40-Iyy6*dQ5*dQ6*t41+Izz5*dQ2*dQ4*t9+Izz5*dQ3*dQ4*t9+Izz6*dQ2*dQ4*t9+Izz6*dQ3*dQ4*t9+Izz6*dQ4*dQ6*t10-Izz5*dQ2*dQ3*t40-Izz6*dQ2*dQ3*t40+Lxcm6*Lycm6*dQ5*dQ6*m6*2.0-Lxcm5*Lzcm5*dQ2*dQ3*m5*2.0-Ixx6*dQ2*dQ6*t5*t9-Ixx6*dQ3*dQ6*t5*t9+Ixx5*dQ2*dQ4*t9*t35*2.0+Ixx5*dQ3*dQ4*t9*t35*2.0-Ixx6*dQ4*dQ6*t10*t36*2.0+Iyy6*dQ2*dQ6*t5*t9+Iyy6*dQ3*dQ6*t5*t9+Iyy6*dQ2*dQ4*t9*t35*2.0+Iyy6*dQ3*dQ4*t9*t35*2.0;
et374 = Iyy6*dQ4*dQ6*t10*t36*2.0-Izz6*dQ2*dQ6*t5*t9-Izz6*dQ3*dQ6*t5*t9-Izz5*dQ2*dQ4*t9*t35*2.0-Izz5*dQ3*dQ4*t9*t35*2.0-Izz6*dQ2*dQ4*t9*t35*2.0-Izz6*dQ3*dQ4*t9*t35*2.0-dQ2*dQ4*m6*t9*t22*2.0-dQ3*dQ4*m6*t9*t22*2.0-dQ2*dQ4*m5*t9*t25*2.0-dQ3*dQ4*m5*t9*t25*2.0-dQ2*dQ4*m6*t9*t26*2.0+dQ4*dQ6*m6*t10*t21*2.0-dQ3*dQ4*m6*t9*t26*2.0-dQ2*dQ3*m5*t17*t40-dQ2*dQ3*m6*t21*t40+dQ2*dQ3*m6*t22*t40+dQ2*dQ3*m5*t25*t40-dQ5*dQ6*m6*t18*t41+dQ2*dQ3*m6*t26*t40+dQ5*dQ6*m6*t21*t41+t5*t6*t9*t11*t84*2.0+t5*t6*t9*t11*t85*2.0-t5*t6*t9*t11*t92*2.0-t5*t6*t9*t11*t93*2.0+Lxcm6*Lycm6*dQ2*dQ6*m6*t4*2.0;
et375 = Lxcm6*Lycm6*dQ3*dQ6*m6*t4*2.0-Lxcm6*Lycm6*dQ5*dQ6*m6*t36*4.0-Lxcm6*Lz6*dQ2*dQ3*m6*t6*2.0-Lxcm6*Lzcm6*dQ2*dQ3*m6*t6*2.0+Lxcm5*Lzcm5*dQ2*dQ3*m5*t34*2.0+Lxcm5*Lzcm5*dQ2*dQ3*m5*t35*4.0+Lycm6*Lz6*dQ2*dQ3*m6*t11*2.0+Lycm6*Lzcm6*dQ2*dQ3*m6*t11*2.0-Lz6*Lzcm6*dQ2*dQ4*m6*t9*4.0-Lz6*Lzcm6*dQ3*dQ4*m6*t9*4.0+Lz6*Lzcm6*dQ2*dQ3*m6*t40*2.0-Ixx5*dQ1*dQ2*t2*t3*t9-Ixx5*dQ1*dQ3*t2*t3*t9+Ixx6*dQ1*dQ2*t2*t3*t9+Ixx6*dQ1*dQ3*t2*t3*t9+Ixx6*dQ1*dQ6*t2*t3*t10+Ixx5*dQ1*dQ2*t7*t8*t9+Ixx5*dQ1*dQ3*t7*t8*t9-Ixx6*dQ1*dQ2*t7*t8*t9-Ixx6*dQ1*dQ3*t7*t8*t9+Ixx6*dQ2*dQ6*t4*t6*t11*2.0+Ixx6*dQ3*dQ6*t4*t6*t11*2.0-Ixx6*dQ1*dQ6*t7*t8*t10-Ixx5*dQ2*dQ3*t5*t10*t34*2.0;
et376 = Ixx6*dQ2*dQ3*t5*t10*t36*2.0+Ixx6*dQ2*dQ6*t5*t9*t36*2.0+Ixx6*dQ3*dQ6*t5*t9*t36*2.0+Ixx6*dQ2*dQ4*t9*t35*t36*2.0+Ixx6*dQ3*dQ4*t9*t35*t36*2.0+Iyy5*dQ1*dQ2*t2*t3*t9+Iyy5*dQ1*dQ3*t2*t3*t9-Iyy6*dQ1*dQ2*t2*t3*t9-Iyy6*dQ1*dQ3*t2*t3*t9-Iyy6*dQ1*dQ6*t2*t3*t10-Iyy5*dQ1*dQ2*t7*t8*t9-Iyy5*dQ1*dQ3*t7*t8*t9+Iyy6*dQ1*dQ2*t7*t8*t9+Iyy6*dQ1*dQ3*t7*t8*t9-Iyy6*dQ2*dQ6*t4*t6*t11*2.0-Iyy6*dQ3*dQ6*t4*t6*t11*2.0+Iyy6*dQ1*dQ6*t7*t8*t10-Iyy6*dQ2*dQ3*t5*t10*t34*2.0-Iyy6*dQ2*dQ3*t5*t10*t36*2.0-Iyy6*dQ2*dQ6*t5*t9*t36*2.0-Iyy6*dQ3*dQ6*t5*t9*t36*2.0-Iyy6*dQ2*dQ4*t9*t35*t36*2.0-Iyy6*dQ3*dQ4*t9*t35*t36*2.0+Izz5*dQ1*dQ2*t2*t3*t9;
et377 = Izz5*dQ1*dQ3*t2*t3*t9+Izz6*dQ1*dQ2*t2*t3*t9+Izz6*dQ1*dQ3*t2*t3*t9+Izz6*dQ1*dQ6*t2*t3*t10-Izz5*dQ1*dQ2*t7*t8*t9-Izz5*dQ1*dQ3*t7*t8*t9-Izz6*dQ1*dQ2*t7*t8*t9-Izz6*dQ1*dQ3*t7*t8*t9-Izz6*dQ1*dQ6*t7*t8*t10+Izz5*dQ2*dQ3*t5*t10*t34*2.0+Izz6*dQ2*dQ3*t5*t10*t34*2.0-dQ2*dQ6*m6*t5*t9*t21*2.0-dQ3*dQ6*m6*t5*t9*t21*2.0-dQ2*dQ4*m5*t9*t17*t35*2.0-dQ3*dQ4*m5*t9*t17*t35*2.0-dQ2*dQ4*m6*t9*t21*t35*2.0+dQ2*dQ4*m6*t9*t22*t35*2.0-dQ3*dQ4*m6*t9*t21*t35*2.0+dQ3*dQ4*m6*t9*t22*t35*2.0+dQ2*dQ4*m5*t9*t25*t35*2.0+dQ4*dQ6*m6*t10*t18*t36*2.0+dQ3*dQ4*m5*t9*t25*t35*2.0+dQ2*dQ4*m6*t9*t26*t35*2.0+dQ3*dQ4*m6*t9*t26*t35*2.0;
et378 = dQ4*dQ6*m6*t10*t21*t36*-2.0+Lx3*Lxcm5*dQ2*dQ3*m5*t4*t10*2.0-Lx4*Lxcm5*dQ2*dQ4*m5*t5*t9*2.0-Lx4*Lxcm5*dQ3*dQ4*m5*t5*t9*2.0+Lx4*Lxcm5*dQ2*dQ3*m5*t10*t34*2.0-Lxcm5*Lycm5*dQ2*dQ4*m5*t4*t5*2.0-Lxcm5*Lycm5*dQ3*dQ4*m5*t4*t5*2.0-Lxcm6*Lycm6*dQ2*dQ6*m6*t4*t36*4.0-Lxcm6*Lycm6*dQ3*dQ6*m6*t4*t36*4.0-Lx3*Lz6*dQ2*dQ3*m6*t4*t5*2.0-Lx4*Lz6*dQ2*dQ4*m6*t9*t10*2.0-Lx4*Lz6*dQ3*dQ4*m6*t9*t10*2.0-Lx4*Lz6*dQ2*dQ3*m6*t5*t34*2.0-Lx3*Lzcm5*dQ2*dQ3*m5*t4*t5*2.0-Lx3*Lzcm6*dQ2*dQ3*m6*t4*t5*2.0-Lx4*Lzcm5*dQ2*dQ4*m5*t9*t10*2.0-Lxcm6*Lz6*dQ4*dQ6*m6*t5*t6*2.0-Lx4*Lzcm5*dQ3*dQ4*m5*t9*t10*2.0-Lx4*Lzcm6*dQ2*dQ4*m6*t9*t10*2.0-Lx4*Lzcm6*dQ3*dQ4*m6*t9*t10*2.0;
et379 = Lx4*Lzcm5*dQ2*dQ3*m5*t5*t34*-2.0-Lx4*Lzcm6*dQ2*dQ3*m6*t5*t34*2.0+Lxcm6*Lz6*dQ2*dQ3*m6*t6*t34*2.0+Lxcm6*Lz6*dQ2*dQ3*m6*t6*t35*4.0+Lxcm5*Lzcm5*dQ1*dQ4*m5*t2*t3*2.0-Lxcm5*Lzcm5*dQ1*dQ4*m5*t7*t8*2.0-Lxcm6*Lzcm6*dQ4*dQ6*m6*t5*t6*2.0+Lxcm6*Lzcm6*dQ2*dQ3*m6*t6*t34*2.0+Lxcm6*Lzcm6*dQ2*dQ3*m6*t6*t35*4.0-Lxcm5*Lzcm5*dQ2*dQ3*m5*t34*t35*4.0+Lycm6*Lz6*dQ4*dQ6*m6*t5*t11*2.0-Lycm6*Lz6*dQ2*dQ3*m6*t11*t34*2.0-Lycm6*Lz6*dQ2*dQ3*m6*t11*t35*4.0-Lycm5*Lzcm5*dQ2*dQ4*m5*t4*t10*2.0-Lycm5*Lzcm5*dQ3*dQ4*m5*t4*t10*2.0+Lycm6*Lzcm6*dQ4*dQ6*m6*t5*t11*2.0-Lycm6*Lzcm6*dQ2*dQ3*m6*t11*t34*2.0-Lycm6*Lzcm6*dQ2*dQ3*m6*t11*t35*4.0+Lz6*Lzcm6*dQ2*dQ4*m6*t9*t35*4.0+Lz6*Lzcm6*dQ3*dQ4*m6*t9*t35*4.0;
et380 = Ixx5*dQ1*dQ4*t2*t3*t5*t10*-2.0+Ixx5*dQ1*dQ4*t5*t7*t8*t10*2.0+Ixx5*dQ1*dQ2*t2*t3*t9*t35*2.0+Ixx5*dQ1*dQ3*t2*t3*t9*t35*2.0-Ixx6*dQ1*dQ2*t2*t3*t9*t36*2.0-Ixx6*dQ1*dQ3*t2*t3*t9*t36*2.0-Ixx6*dQ1*dQ6*t2*t3*t10*t36*2.0-Ixx5*dQ1*dQ2*t7*t8*t9*t35*2.0-Ixx5*dQ1*dQ3*t7*t8*t9*t35*2.0+Ixx6*dQ1*dQ2*t7*t8*t9*t36*2.0+Ixx6*dQ1*dQ3*t7*t8*t9*t36*2.0+Ixx6*dQ1*dQ6*t7*t8*t10*t36*2.0-Ixx6*dQ2*dQ3*t5*t10*t34*t36*2.0-Iyy6*dQ1*dQ4*t2*t3*t5*t10*2.0-Iyy6*dQ2*dQ4*t4*t5*t6*t11*2.0-Iyy6*dQ3*dQ4*t4*t5*t6*t11*2.0+Iyy6*dQ1*dQ4*t5*t7*t8*t10*2.0+Iyy6*dQ1*dQ2*t2*t3*t9*t35*2.0+Iyy6*dQ1*dQ2*t2*t3*t9*t36*2.0+Iyy6*dQ1*dQ3*t2*t3*t9*t35*2.0+Iyy6*dQ1*dQ3*t2*t3*t9*t36*2.0;
et381 = Iyy6*dQ1*dQ6*t2*t3*t10*t36*2.0-Iyy6*dQ1*dQ2*t7*t8*t9*t35*2.0-Iyy6*dQ1*dQ2*t7*t8*t9*t36*2.0-Iyy6*dQ1*dQ3*t7*t8*t9*t35*2.0-Iyy6*dQ1*dQ3*t7*t8*t9*t36*2.0-Iyy6*dQ1*dQ6*t7*t8*t10*t36*2.0+Iyy6*dQ2*dQ3*t5*t10*t34*t36*2.0+Izz5*dQ1*dQ4*t2*t3*t5*t10*2.0+Izz6*dQ1*dQ4*t2*t3*t5*t10*2.0-Izz5*dQ1*dQ4*t5*t7*t8*t10*2.0-Izz6*dQ1*dQ4*t5*t7*t8*t10*2.0-Izz5*dQ1*dQ2*t2*t3*t9*t35*2.0-Izz5*dQ1*dQ3*t2*t3*t9*t35*2.0-Izz6*dQ1*dQ2*t2*t3*t9*t35*2.0-Izz6*dQ1*dQ3*t2*t3*t9*t35*2.0+Izz5*dQ1*dQ2*t7*t8*t9*t35*2.0+Izz5*dQ1*dQ3*t7*t8*t9*t35*2.0+Izz6*dQ1*dQ2*t7*t8*t9*t35*2.0+Izz6*dQ1*dQ3*t7*t8*t9*t35*2.0+dQ1*dQ2*m5*t2*t3*t9*t17*2.0+dQ1*dQ3*m5*t2*t3*t9*t17*2.0;
et382 = dQ1*dQ2*m6*t2*t3*t9*t21*2.0+dQ1*dQ3*m6*t2*t3*t9*t21*2.0+dQ1*dQ4*m6*t2*t4*t8*t22*2.0+dQ1*dQ4*m6*t3*t4*t7*t22*2.0-dQ1*dQ2*m5*t7*t8*t9*t17*2.0+dQ1*dQ4*m5*t2*t4*t8*t25*2.0+dQ1*dQ4*m5*t3*t4*t7*t25*2.0+dQ1*dQ6*m6*t2*t3*t10*t21*2.0-dQ1*dQ3*m5*t7*t8*t9*t17*2.0+dQ1*dQ4*m6*t2*t4*t8*t26*2.0+dQ1*dQ4*m6*t3*t4*t7*t26*2.0-dQ2*dQ6*m6*t4*t6*t11*t18*2.0-dQ1*dQ2*m6*t7*t8*t9*t21*2.0-dQ3*dQ6*m6*t4*t6*t11*t18*2.0-dQ1*dQ3*m6*t7*t8*t9*t21*2.0+dQ2*dQ6*m6*t4*t6*t11*t21*2.0+dQ3*dQ6*m6*t4*t6*t11*t21*2.0-dQ1*dQ6*m6*t7*t8*t10*t21*2.0+dQ2*dQ3*m5*t5*t10*t17*t34*2.0-dQ2*dQ3*m6*t5*t10*t18*t36*2.0+dQ2*dQ3*m6*t5*t10*t21*t34*2.0;
et383 = dQ2*dQ3*m6*t5*t10*t22*t34*-2.0-dQ2*dQ6*m6*t5*t9*t18*t36*2.0+dQ2*dQ3*m6*t5*t10*t21*t36*2.0-dQ3*dQ6*m6*t5*t9*t18*t36*2.0-dQ2*dQ3*m5*t5*t10*t25*t34*2.0+dQ2*dQ6*m6*t5*t9*t21*t36*2.0-dQ2*dQ3*m6*t5*t10*t26*t34*2.0+dQ3*dQ6*m6*t5*t9*t21*t36*2.0-dQ2*dQ4*m6*t9*t18*t35*t36*2.0-dQ3*dQ4*m6*t9*t18*t35*t36*2.0+dQ2*dQ4*m6*t9*t21*t35*t36*2.0+dQ3*dQ4*m6*t9*t21*t35*t36*2.0+Lx4*Lxcm5*dQ1*dQ4*m5*t2*t3*t10*2.0+Lx3*Lxcm6*dQ2*dQ3*m6*t4*t6*t10*2.0+Lx2*Lxcm5*dQ1*dQ2*m5*t7*t9*t10*2.0-Lx4*Lxcm6*dQ2*dQ4*m6*t5*t6*t9*2.0-Lx4*Lxcm6*dQ3*dQ4*m6*t5*t6*t9*2.0-Lx4*Lxcm5*dQ1*dQ4*m5*t7*t8*t10*2.0+Lx4*Lxcm6*dQ2*dQ3*m6*t6*t10*t34*2.0-Lx3*Lycm6*dQ2*dQ3*m6*t4*t10*t11*2.0;
et384 = Lx4*Lycm6*dQ2*dQ4*m6*t5*t9*t11*2.0+Lx4*Lycm6*dQ3*dQ4*m6*t5*t9*t11*2.0-Lx4*Lycm6*dQ2*dQ3*m6*t10*t11*t34*2.0-Lxcm5*Lycm5*dQ1*dQ2*m5*t2*t8*t10*2.0-Lxcm5*Lycm5*dQ1*dQ2*m5*t3*t7*t10*2.0-Lxcm5*Lycm5*dQ1*dQ3*m5*t2*t8*t10*2.0-Lxcm5*Lycm5*dQ1*dQ3*m5*t3*t7*t10*2.0+Lxcm6*Lycm6*dQ1*dQ2*m6*t2*t8*t10*2.0+Lxcm6*Lycm6*dQ1*dQ2*m6*t3*t7*t10*2.0+Lxcm6*Lycm6*dQ1*dQ3*m6*t2*t8*t10*2.0+Lxcm6*Lycm6*dQ1*dQ3*m6*t3*t7*t10*2.0-Lxcm5*Lycm5*dQ2*dQ3*m5*t4*t9*t10*2.0+Lxcm6*Lycm6*dQ1*dQ6*m6*t2*t8*t9*2.0+Lxcm6*Lycm6*dQ1*dQ6*m6*t3*t7*t9*2.0+Lxcm6*Lycm6*dQ2*dQ3*m6*t4*t9*t10*2.0-Lxcm6*Lycm6*dQ4*dQ6*m6*t6*t10*t11*4.0-Lxcm6*Lycm6*dQ2*dQ4*m6*t4*t5*t36*4.0-Lxcm6*Lycm6*dQ3*dQ4*m6*t4*t5*t36*4.0-Lx4*Lz6*dQ1*dQ4*m6*t2*t3*t5*2.0;
et385 = Lx2*Lz6*dQ1*dQ2*m6*t5*t7*t9*-2.0+Lx4*Lz6*dQ1*dQ4*m6*t5*t7*t8*2.0-Lx4*Lzcm5*dQ1*dQ4*m5*t2*t3*t5*2.0-Lx4*Lzcm6*dQ1*dQ4*m6*t2*t3*t5*2.0+Lxcm6*Lz6*dQ1*dQ4*m6*t2*t3*t6*2.0-Lx2*Lzcm5*dQ1*dQ2*m5*t5*t7*t9*2.0-Lx2*Lzcm6*dQ1*dQ2*m6*t5*t7*t9*2.0+Lx4*Lzcm5*dQ1*dQ4*m5*t5*t7*t8*2.0+Lx4*Lzcm6*dQ1*dQ4*m6*t5*t7*t8*2.0-Lxcm6*Lz6*dQ1*dQ4*m6*t6*t7*t8*2.0-Lxcm6*Lz6*dQ2*dQ4*m6*t4*t10*t11*2.0-Lxcm6*Lz6*dQ3*dQ4*m6*t4*t10*t11*2.0-Lxcm6*Lz6*dQ2*dQ6*m6*t6*t9*t10*2.0-Lxcm6*Lz6*dQ3*dQ6*m6*t6*t9*t10*2.0-Lxcm6*Lz6*dQ2*dQ3*m6*t6*t34*t35*4.0+Lxcm6*Lzcm6*dQ1*dQ4*m6*t2*t3*t6*2.0-Lxcm6*Lzcm6*dQ1*dQ4*m6*t6*t7*t8*2.0-Lxcm5*Lzcm5*dQ2*dQ4*m5*t5*t9*t10*4.0;
et386 = Lxcm5*Lzcm5*dQ3*dQ4*m5*t5*t9*t10*-4.0-Lxcm6*Lzcm6*dQ2*dQ4*m6*t4*t10*t11*2.0-Lxcm6*Lzcm6*dQ3*dQ4*m6*t4*t10*t11*2.0-Lxcm6*Lzcm6*dQ2*dQ6*m6*t6*t9*t10*2.0-Lxcm6*Lzcm6*dQ3*dQ6*m6*t6*t9*t10*2.0-Lxcm5*Lzcm5*dQ1*dQ4*m5*t2*t3*t35*4.0+Lxcm5*Lzcm5*dQ1*dQ4*m5*t7*t8*t35*4.0-Lxcm6*Lzcm6*dQ2*dQ3*m6*t6*t34*t35*4.0-Lycm6*Lz6*dQ1*dQ4*m6*t2*t3*t11*2.0-Lycm6*Lz6*dQ2*dQ4*m6*t4*t6*t10*2.0-Lycm6*Lz6*dQ3*dQ4*m6*t4*t6*t10*2.0+Lycm6*Lz6*dQ1*dQ4*m6*t7*t8*t11*2.0+Lycm6*Lz6*dQ2*dQ6*m6*t9*t10*t11*2.0+Lycm6*Lz6*dQ3*dQ6*m6*t9*t10*t11*2.0+Lycm6*Lz6*dQ2*dQ3*m6*t11*t34*t35*4.0+Lycm5*Lzcm5*dQ1*dQ2*m5*t2*t5*t8*2.0+Lycm5*Lzcm5*dQ1*dQ2*m5*t3*t5*t7*2.0+Lycm5*Lzcm5*dQ1*dQ3*m5*t2*t5*t8*2.0+Lycm5*Lzcm5*dQ1*dQ3*m5*t3*t5*t7*2.0;
et387 = Lycm5*Lzcm5*dQ2*dQ3*m5*t4*t5*t9*2.0-Lycm6*Lzcm6*dQ1*dQ4*m6*t2*t3*t11*2.0-Lycm6*Lzcm6*dQ2*dQ4*m6*t4*t6*t10*2.0-Lycm6*Lzcm6*dQ3*dQ4*m6*t4*t6*t10*2.0+Lycm6*Lzcm6*dQ1*dQ4*m6*t7*t8*t11*2.0+Lycm6*Lzcm6*dQ2*dQ6*m6*t9*t10*t11*2.0+Lycm6*Lzcm6*dQ3*dQ6*m6*t9*t10*t11*2.0+Lycm6*Lzcm6*dQ2*dQ3*m6*t11*t34*t35*4.0+Lz6*Lzcm6*dQ1*dQ4*m6*t2*t4*t8*4.0+Lz6*Lzcm6*dQ1*dQ4*m6*t3*t4*t7*4.0-Lz6*Lzcm6*dQ2*dQ3*m6*t5*t10*t34*4.0+Ixx6*dQ1*dQ2*t2*t6*t8*t10*t11*2.0+Ixx6*dQ1*dQ2*t3*t6*t7*t10*t11*2.0+Ixx6*dQ1*dQ3*t2*t6*t8*t10*t11*2.0+Ixx6*dQ1*dQ3*t3*t6*t7*t10*t11*2.0+Ixx6*dQ1*dQ6*t2*t6*t8*t9*t11*2.0+Ixx6*dQ1*dQ6*t3*t6*t7*t9*t11*2.0+Ixx6*dQ2*dQ3*t4*t6*t9*t10*t11*2.0-Ixx6*dQ1*dQ4*t2*t3*t5*t10*t36*2.0;
et388 = Ixx6*dQ1*dQ4*t5*t7*t8*t10*t36*2.0+Ixx6*dQ1*dQ2*t2*t3*t9*t35*t36*2.0+Ixx6*dQ1*dQ3*t2*t3*t9*t35*t36*2.0-Ixx6*dQ1*dQ2*t7*t8*t9*t35*t36*2.0-Ixx6*dQ1*dQ3*t7*t8*t9*t35*t36*2.0-Iyy6*dQ1*dQ2*t2*t6*t8*t10*t11*2.0-Iyy6*dQ1*dQ2*t3*t6*t7*t10*t11*2.0-Iyy6*dQ1*dQ3*t2*t6*t8*t10*t11*2.0-Iyy6*dQ1*dQ3*t3*t6*t7*t10*t11*2.0-Iyy6*dQ1*dQ6*t2*t6*t8*t9*t11*2.0-Iyy6*dQ1*dQ6*t3*t6*t7*t9*t11*2.0-Iyy6*dQ2*dQ3*t4*t6*t9*t10*t11*2.0+Iyy6*dQ1*dQ4*t2*t3*t5*t10*t36*2.0-Iyy6*dQ1*dQ4*t5*t7*t8*t10*t36*2.0-Iyy6*dQ1*dQ2*t2*t3*t9*t35*t36*2.0-Iyy6*dQ1*dQ3*t2*t3*t9*t35*t36*2.0+Iyy6*dQ1*dQ2*t7*t8*t9*t35*t36*2.0+Iyy6*dQ1*dQ3*t7*t8*t9*t35*t36*2.0;
et389 = dQ1*dQ4*m5*t2*t3*t5*t10*t17*2.0+dQ1*dQ4*m6*t2*t3*t5*t10*t21*2.0-dQ1*dQ4*m6*t2*t3*t5*t10*t22*2.0+dQ1*dQ6*m6*t2*t4*t5*t8*t21*2.0+dQ1*dQ6*m6*t3*t4*t5*t7*t21*2.0-dQ1*dQ4*m5*t2*t3*t5*t10*t25*2.0-dQ2*dQ4*m6*t4*t5*t6*t11*t18*2.0-dQ1*dQ4*m5*t5*t7*t8*t10*t17*2.0-dQ1*dQ4*m6*t2*t3*t5*t10*t26*2.0-dQ3*dQ4*m6*t4*t5*t6*t11*t18*2.0-dQ1*dQ4*m6*t5*t7*t8*t10*t21*2.0+dQ1*dQ4*m6*t5*t7*t8*t10*t22*2.0+dQ1*dQ4*m5*t5*t7*t8*t10*t25*2.0+dQ1*dQ4*m6*t5*t7*t8*t10*t26*2.0-dQ1*dQ2*m5*t2*t3*t9*t17*t35*2.0-dQ1*dQ3*m5*t2*t3*t9*t17*t35*2.0+dQ1*dQ4*m5*t2*t4*t8*t17*t35*2.0+dQ1*dQ4*m5*t3*t4*t7*t17*t35*2.0+dQ1*dQ2*m6*t2*t3*t9*t18*t36*2.0;
et390 = dQ1*dQ3*m6*t2*t3*t9*t18*t36*2.0-dQ1*dQ2*m6*t2*t3*t9*t21*t35*2.0-dQ1*dQ2*m6*t2*t3*t9*t21*t36*2.0+dQ1*dQ2*m6*t2*t3*t9*t22*t35*2.0-dQ1*dQ3*m6*t2*t3*t9*t21*t35*2.0-dQ1*dQ3*m6*t2*t3*t9*t21*t36*2.0+dQ1*dQ3*m6*t2*t3*t9*t22*t35*2.0+dQ1*dQ4*m6*t2*t4*t8*t21*t35*2.0+dQ1*dQ4*m6*t3*t4*t7*t21*t35*2.0+dQ1*dQ2*m5*t2*t3*t9*t25*t35*2.0-dQ1*dQ4*m6*t2*t4*t8*t22*t35*2.0-dQ1*dQ4*m6*t3*t4*t7*t22*t35*2.0+dQ1*dQ6*m6*t2*t3*t10*t18*t36*2.0+dQ1*dQ3*m5*t2*t3*t9*t25*t35*2.0+dQ1*dQ2*m5*t7*t8*t9*t17*t35*2.0+dQ1*dQ2*m6*t2*t3*t9*t26*t35*2.0-dQ1*dQ4*m5*t2*t4*t8*t25*t35*2.0-dQ1*dQ4*m5*t3*t4*t7*t25*t35*2.0+dQ1*dQ3*m5*t7*t8*t9*t17*t35*2.0;
et391 = dQ1*dQ3*m6*t2*t3*t9*t26*t35*2.0-dQ1*dQ6*m6*t2*t3*t10*t21*t36*2.0-dQ1*dQ4*m6*t2*t4*t8*t26*t35*2.0-dQ1*dQ4*m6*t3*t4*t7*t26*t35*2.0-dQ1*dQ2*m6*t7*t8*t9*t18*t36*2.0-dQ1*dQ3*m6*t7*t8*t9*t18*t36*2.0+dQ1*dQ2*m6*t7*t8*t9*t21*t35*2.0+dQ1*dQ2*m6*t7*t8*t9*t21*t36*2.0-dQ1*dQ2*m6*t7*t8*t9*t22*t35*2.0+dQ1*dQ3*m6*t7*t8*t9*t21*t35*2.0+dQ1*dQ3*m6*t7*t8*t9*t21*t36*2.0-dQ1*dQ3*m6*t7*t8*t9*t22*t35*2.0-dQ1*dQ2*m5*t7*t8*t9*t25*t35*2.0-dQ1*dQ6*m6*t7*t8*t10*t18*t36*2.0-dQ1*dQ3*m5*t7*t8*t9*t25*t35*2.0-dQ1*dQ2*m6*t7*t8*t9*t26*t35*2.0-dQ1*dQ3*m6*t7*t8*t9*t26*t35*2.0+dQ1*dQ6*m6*t7*t8*t10*t21*t36*2.0;
et392 = dQ2*dQ3*m6*t5*t10*t18*t34*t36*2.0-dQ2*dQ3*m6*t5*t10*t21*t34*t36*2.0-Ixx5*dQ1*dQ2*t2*t4*t5*t8*t9*t10*2.0-Ixx5*dQ1*dQ2*t3*t4*t5*t7*t9*t10*2.0-Ixx5*dQ1*dQ3*t2*t4*t5*t8*t9*t10*2.0-Ixx5*dQ1*dQ3*t3*t4*t5*t7*t9*t10*2.0-Ixx6*dQ1*dQ2*t2*t6*t8*t10*t11*t34*2.0-Ixx6*dQ1*dQ2*t3*t6*t7*t10*t11*t34*2.0-Ixx6*dQ1*dQ3*t2*t6*t8*t10*t11*t34*2.0-Ixx6*dQ1*dQ3*t3*t6*t7*t10*t11*t34*2.0-Iyy6*dQ1*dQ2*t2*t4*t5*t8*t9*t10*2.0-Iyy6*dQ1*dQ2*t3*t4*t5*t7*t9*t10*2.0-Iyy6*dQ1*dQ3*t2*t4*t5*t8*t9*t10*2.0-Iyy6*dQ1*dQ3*t3*t4*t5*t7*t9*t10*2.0+Iyy6*dQ1*dQ2*t2*t6*t8*t10*t11*t34*2.0+Iyy6*dQ1*dQ2*t3*t6*t7*t10*t11*t34*2.0+Iyy6*dQ1*dQ3*t2*t6*t8*t10*t11*t34*2.0;
et393 = Iyy6*dQ1*dQ3*t3*t6*t7*t10*t11*t34*2.0+Izz5*dQ1*dQ2*t2*t4*t5*t8*t9*t10*2.0+Izz5*dQ1*dQ2*t3*t4*t5*t7*t9*t10*2.0+Izz5*dQ1*dQ3*t2*t4*t5*t8*t9*t10*2.0+Izz5*dQ1*dQ3*t3*t4*t5*t7*t9*t10*2.0+Izz6*dQ1*dQ2*t2*t4*t5*t8*t9*t10*2.0+Izz6*dQ1*dQ2*t3*t4*t5*t7*t9*t10*2.0+Izz6*dQ1*dQ3*t2*t4*t5*t8*t9*t10*2.0+Izz6*dQ1*dQ3*t3*t4*t5*t7*t9*t10*2.0-dQ1*dQ2*m6*t2*t6*t8*t10*t11*t18*2.0-dQ1*dQ2*m6*t3*t6*t7*t10*t11*t18*2.0-dQ1*dQ3*m6*t2*t6*t8*t10*t11*t18*2.0-dQ1*dQ3*m6*t3*t6*t7*t10*t11*t18*2.0+dQ1*dQ2*m6*t2*t6*t8*t10*t11*t21*2.0+dQ1*dQ2*m6*t3*t6*t7*t10*t11*t21*2.0-dQ1*dQ6*m6*t2*t6*t8*t9*t11*t18*2.0-dQ1*dQ6*m6*t3*t6*t7*t9*t11*t18*2.0;
et394 = dQ1*dQ3*m6*t2*t6*t8*t10*t11*t21*2.0+dQ1*dQ3*m6*t3*t6*t7*t10*t11*t21*2.0-dQ2*dQ3*m6*t4*t6*t9*t10*t11*t18*2.0+dQ1*dQ6*m6*t2*t6*t8*t9*t11*t21*2.0+dQ1*dQ6*m6*t3*t6*t7*t9*t11*t21*2.0+dQ2*dQ3*m6*t4*t6*t9*t10*t11*t21*2.0+dQ1*dQ4*m6*t2*t3*t5*t10*t18*t36*2.0-dQ1*dQ4*m6*t2*t3*t5*t10*t21*t36*2.0-dQ1*dQ6*m6*t2*t4*t5*t8*t21*t36*2.0-dQ1*dQ6*m6*t3*t4*t5*t7*t21*t36*2.0-dQ1*dQ4*m6*t5*t7*t8*t10*t18*t36*2.0+dQ1*dQ4*m6*t5*t7*t8*t10*t21*t36*2.0-dQ1*dQ2*m6*t2*t3*t9*t18*t35*t36*2.0-dQ1*dQ3*m6*t2*t3*t9*t18*t35*t36*2.0+dQ1*dQ2*m6*t2*t3*t9*t21*t35*t36*2.0+dQ1*dQ3*m6*t2*t3*t9*t21*t35*t36*2.0-dQ1*dQ4*m6*t2*t4*t8*t21*t35*t36*2.0;
et395 = dQ1*dQ4*m6*t3*t4*t7*t21*t35*t36*-2.0+dQ1*dQ2*m6*t7*t8*t9*t18*t35*t36*2.0+dQ1*dQ3*m6*t7*t8*t9*t18*t35*t36*2.0-dQ1*dQ2*m6*t7*t8*t9*t21*t35*t36*2.0-dQ1*dQ3*m6*t7*t8*t9*t21*t35*t36*2.0+Lx4*Lxcm5*dQ1*dQ4*m5*t2*t4*t5*t8*2.0+Lx4*Lxcm5*dQ1*dQ4*m5*t3*t4*t5*t7*2.0+Lx4*Lxcm6*dQ1*dQ4*m6*t2*t3*t6*t10*2.0+Lx3*Lxcm5*dQ1*dQ2*m5*t2*t8*t9*t10*2.0+Lx3*Lxcm5*dQ1*dQ2*m5*t3*t7*t9*t10*2.0+Lx3*Lxcm5*dQ1*dQ3*m5*t2*t8*t9*t10*2.0+Lx3*Lxcm5*dQ1*dQ3*m5*t3*t7*t9*t10*2.0+Lx2*Lxcm6*dQ1*dQ2*m6*t6*t7*t9*t10*2.0-Lx4*Lxcm6*dQ1*dQ4*m6*t6*t7*t8*t10*2.0-Lx4*Lycm6*dQ1*dQ4*m6*t2*t3*t10*t11*2.0-Lx2*Lycm6*dQ1*dQ2*m6*t7*t9*t10*t11*2.0+Lx4*Lycm6*dQ1*dQ4*m6*t7*t8*t10*t11*2.0;
et396 = Lxcm5*Lycm5*dQ1*dQ4*m5*t2*t5*t8*t9*-2.0-Lxcm5*Lycm5*dQ1*dQ4*m5*t3*t5*t7*t9*2.0+Lxcm6*Lycm6*dQ1*dQ4*m6*t2*t5*t8*t9*2.0+Lxcm6*Lycm6*dQ1*dQ4*m6*t3*t5*t7*t9*2.0+Lxcm6*Lycm6*dQ2*dQ3*m6*t5*t6*t10*t11*4.0+Lxcm6*Lycm6*dQ2*dQ6*m6*t5*t6*t9*t11*4.0+Lxcm6*Lycm6*dQ3*dQ6*m6*t5*t6*t9*t11*4.0+Lxcm5*Lycm5*dQ1*dQ2*m5*t2*t8*t10*t34*2.0+Lxcm5*Lycm5*dQ1*dQ2*m5*t3*t7*t10*t34*2.0+Lxcm5*Lycm5*dQ1*dQ3*m5*t2*t8*t10*t34*2.0+Lxcm5*Lycm5*dQ1*dQ3*m5*t3*t7*t10*t34*2.0-Lxcm6*Lycm6*dQ1*dQ2*m6*t2*t8*t10*t34*2.0-Lxcm6*Lycm6*dQ1*dQ2*m6*t3*t7*t10*t34*2.0-Lxcm6*Lycm6*dQ1*dQ3*m6*t2*t8*t10*t34*2.0-Lxcm6*Lycm6*dQ1*dQ3*m6*t3*t7*t10*t34*2.0-Lxcm6*Lycm6*dQ1*dQ2*m6*t2*t8*t10*t36*4.0-Lxcm6*Lycm6*dQ1*dQ2*m6*t3*t7*t10*t36*4.0;
et397 = Lxcm6*Lycm6*dQ1*dQ3*m6*t2*t8*t10*t36*-4.0-Lxcm6*Lycm6*dQ1*dQ3*m6*t3*t7*t10*t36*4.0-Lxcm6*Lycm6*dQ1*dQ6*m6*t2*t8*t9*t36*4.0-Lxcm6*Lycm6*dQ1*dQ6*m6*t3*t7*t9*t36*4.0-Lxcm6*Lycm6*dQ2*dQ3*m6*t4*t9*t10*t36*4.0+Lxcm6*Lycm6*dQ2*dQ4*m6*t6*t9*t11*t35*4.0+Lxcm6*Lycm6*dQ3*dQ4*m6*t6*t9*t11*t35*4.0-Lx3*Lz6*dQ1*dQ2*m6*t2*t5*t8*t9*2.0-Lx3*Lz6*dQ1*dQ2*m6*t3*t5*t7*t9*2.0-Lx3*Lz6*dQ1*dQ3*m6*t2*t5*t8*t9*2.0-Lx3*Lz6*dQ1*dQ3*m6*t3*t5*t7*t9*2.0+Lx4*Lz6*dQ1*dQ4*m6*t2*t4*t8*t10*2.0+Lx4*Lz6*dQ1*dQ4*m6*t3*t4*t7*t10*2.0-Lx3*Lzcm5*dQ1*dQ2*m5*t2*t5*t8*t9*2.0-Lx3*Lzcm5*dQ1*dQ2*m5*t3*t5*t7*t9*2.0-Lx3*Lzcm5*dQ1*dQ3*m5*t2*t5*t8*t9*2.0-Lx3*Lzcm5*dQ1*dQ3*m5*t3*t5*t7*t9*2.0;
et398 = Lxcm6*Lz6*dQ1*dQ6*m6*t2*t3*t5*t6*-2.0-Lx3*Lzcm6*dQ1*dQ2*m6*t2*t5*t8*t9*2.0-Lx3*Lzcm6*dQ1*dQ2*m6*t3*t5*t7*t9*2.0-Lx3*Lzcm6*dQ1*dQ3*m6*t2*t5*t8*t9*2.0-Lx3*Lzcm6*dQ1*dQ3*m6*t3*t5*t7*t9*2.0+Lx4*Lzcm5*dQ1*dQ4*m5*t2*t4*t8*t10*2.0+Lx4*Lzcm5*dQ1*dQ4*m5*t3*t4*t7*t10*2.0+Lx4*Lzcm6*dQ1*dQ4*m6*t2*t4*t8*t10*2.0+Lx4*Lzcm6*dQ1*dQ4*m6*t3*t4*t7*t10*2.0+Lxcm6*Lz6*dQ1*dQ2*m6*t2*t5*t8*t11*2.0+Lxcm6*Lz6*dQ1*dQ2*m6*t3*t5*t7*t11*2.0+Lxcm6*Lz6*dQ1*dQ3*m6*t2*t5*t8*t11*2.0+Lxcm6*Lz6*dQ1*dQ3*m6*t3*t5*t7*t11*2.0+Lxcm6*Lz6*dQ1*dQ6*m6*t5*t6*t7*t8*2.0+Lxcm6*Lz6*dQ2*dQ3*m6*t4*t5*t9*t11*2.0-Lxcm6*Lz6*dQ2*dQ4*m6*t5*t6*t9*t10*4.0-Lxcm6*Lz6*dQ3*dQ4*m6*t5*t6*t9*t10*4.0;
et399 = Lxcm6*Lz6*dQ1*dQ4*m6*t2*t3*t6*t35*-4.0+Lxcm6*Lz6*dQ1*dQ4*m6*t6*t7*t8*t35*4.0+Lxcm5*Lzcm5*dQ1*dQ2*m5*t2*t4*t8*t9*2.0+Lxcm5*Lzcm5*dQ1*dQ2*m5*t3*t4*t7*t9*2.0-Lxcm6*Lzcm6*dQ1*dQ6*m6*t2*t3*t5*t6*2.0+Lxcm5*Lzcm5*dQ1*dQ3*m5*t2*t4*t8*t9*2.0+Lxcm5*Lzcm5*dQ1*dQ3*m5*t3*t4*t7*t9*2.0+Lxcm6*Lzcm6*dQ1*dQ2*m6*t2*t5*t8*t11*2.0+Lxcm6*Lzcm6*dQ1*dQ2*m6*t3*t5*t7*t11*2.0+Lxcm6*Lzcm6*dQ1*dQ3*m6*t2*t5*t8*t11*2.0+Lxcm6*Lzcm6*dQ1*dQ3*m6*t3*t5*t7*t11*2.0+Lxcm6*Lzcm6*dQ1*dQ6*m6*t5*t6*t7*t8*2.0+Lxcm6*Lzcm6*dQ2*dQ3*m6*t4*t5*t9*t11*2.0-Lxcm6*Lzcm6*dQ2*dQ4*m6*t5*t6*t9*t10*4.0-Lxcm6*Lzcm6*dQ3*dQ4*m6*t5*t6*t9*t10*4.0-Lxcm6*Lzcm6*dQ1*dQ4*m6*t2*t3*t6*t35*4.0+Lxcm6*Lzcm6*dQ1*dQ4*m6*t6*t7*t8*t35*4.0;
et400 = Lycm6*Lz6*dQ1*dQ2*m6*t2*t5*t6*t8*2.0+Lycm6*Lz6*dQ1*dQ2*m6*t3*t5*t6*t7*2.0+Lycm6*Lz6*dQ1*dQ3*m6*t2*t5*t6*t8*2.0+Lycm6*Lz6*dQ1*dQ3*m6*t3*t5*t6*t7*2.0+Lycm6*Lz6*dQ1*dQ6*m6*t2*t3*t5*t11*2.0+Lycm6*Lz6*dQ2*dQ3*m6*t4*t5*t6*t9*2.0-Lycm6*Lz6*dQ1*dQ6*m6*t5*t7*t8*t11*2.0+Lycm6*Lz6*dQ2*dQ4*m6*t5*t9*t10*t11*4.0+Lycm6*Lz6*dQ3*dQ4*m6*t5*t9*t10*t11*4.0+Lycm6*Lz6*dQ1*dQ4*m6*t2*t3*t11*t35*4.0-Lycm6*Lz6*dQ1*dQ4*m6*t7*t8*t11*t35*4.0+Lycm6*Lzcm6*dQ1*dQ2*m6*t2*t5*t6*t8*2.0+Lycm6*Lzcm6*dQ1*dQ2*m6*t3*t5*t6*t7*2.0+Lycm6*Lzcm6*dQ1*dQ3*m6*t2*t5*t6*t8*2.0+Lycm6*Lzcm6*dQ1*dQ3*m6*t3*t5*t6*t7*2.0+Lycm6*Lzcm6*dQ1*dQ6*m6*t2*t3*t5*t11*2.0+Lycm6*Lzcm6*dQ2*dQ3*m6*t4*t5*t6*t9*2.0;
et401 = Lycm5*Lzcm5*dQ1*dQ4*m5*t2*t8*t9*t10*-2.0-Lycm5*Lzcm5*dQ1*dQ4*m5*t3*t7*t9*t10*2.0-Lycm6*Lzcm6*dQ1*dQ6*m6*t5*t7*t8*t11*2.0+Lycm6*Lzcm6*dQ2*dQ4*m6*t5*t9*t10*t11*4.0+Lycm6*Lzcm6*dQ3*dQ4*m6*t5*t9*t10*t11*4.0-Lycm5*Lzcm5*dQ1*dQ2*m5*t2*t5*t8*t34*2.0-Lycm5*Lzcm5*dQ1*dQ2*m5*t3*t5*t7*t34*2.0-Lycm5*Lzcm5*dQ1*dQ3*m5*t2*t5*t8*t34*2.0-Lycm5*Lzcm5*dQ1*dQ3*m5*t3*t5*t7*t34*2.0+Lycm6*Lzcm6*dQ1*dQ4*m6*t2*t3*t11*t35*4.0-Lycm6*Lzcm6*dQ1*dQ4*m6*t7*t8*t11*t35*4.0-Lz6*Lzcm6*dQ1*dQ4*m6*t2*t3*t5*t10*4.0+Lz6*Lzcm6*dQ1*dQ4*m6*t5*t7*t8*t10*4.0+Lz6*Lzcm6*dQ1*dQ2*m6*t2*t3*t9*t35*4.0+Lz6*Lzcm6*dQ1*dQ3*m6*t2*t3*t9*t35*4.0-Lz6*Lzcm6*dQ1*dQ4*m6*t2*t4*t8*t35*4.0-Lz6*Lzcm6*dQ1*dQ4*m6*t3*t4*t7*t35*4.0;
et402 = Lz6*Lzcm6*dQ1*dQ2*m6*t7*t8*t9*t35*-4.0-Lz6*Lzcm6*dQ1*dQ3*m6*t7*t8*t9*t35*4.0+Lx4*Lxcm6*dQ1*dQ4*m6*t2*t4*t5*t6*t8*2.0+Lx4*Lxcm6*dQ1*dQ4*m6*t3*t4*t5*t6*t7*2.0+Lx4*Lxcm5*dQ1*dQ2*m5*t2*t4*t8*t9*t10*2.0+Lx4*Lxcm5*dQ1*dQ2*m5*t3*t4*t7*t9*t10*2.0+Lx4*Lxcm5*dQ1*dQ3*m5*t2*t4*t8*t9*t10*2.0+Lx4*Lxcm5*dQ1*dQ3*m5*t3*t4*t7*t9*t10*2.0+Lx3*Lxcm6*dQ1*dQ2*m6*t2*t6*t8*t9*t10*2.0+Lx3*Lxcm6*dQ1*dQ2*m6*t3*t6*t7*t9*t10*2.0+Lx3*Lxcm6*dQ1*dQ3*m6*t2*t6*t8*t9*t10*2.0+Lx3*Lxcm6*dQ1*dQ3*m6*t3*t6*t7*t9*t10*2.0-Lx4*Lycm6*dQ1*dQ4*m6*t2*t4*t5*t8*t11*2.0-Lx4*Lycm6*dQ1*dQ4*m6*t3*t4*t5*t7*t11*2.0-Lx3*Lycm6*dQ1*dQ2*m6*t2*t8*t9*t10*t11*2.0-Lx3*Lycm6*dQ1*dQ2*m6*t3*t7*t9*t10*t11*2.0;
et403 = Lx3*Lycm6*dQ1*dQ3*m6*t2*t8*t9*t10*t11*-2.0-Lx3*Lycm6*dQ1*dQ3*m6*t3*t7*t9*t10*t11*2.0-Lxcm6*Lycm6*dQ1*dQ2*m6*t2*t3*t6*t9*t11*4.0-Lxcm6*Lycm6*dQ1*dQ3*m6*t2*t3*t6*t9*t11*4.0-Lxcm6*Lycm6*dQ1*dQ6*m6*t2*t3*t6*t10*t11*4.0+Lxcm6*Lycm6*dQ1*dQ2*m6*t6*t7*t8*t9*t11*4.0+Lxcm6*Lycm6*dQ1*dQ3*m6*t6*t7*t8*t9*t11*4.0+Lxcm6*Lycm6*dQ1*dQ6*m6*t6*t7*t8*t10*t11*4.0-Lxcm6*Lycm6*dQ1*dQ4*m6*t2*t5*t8*t9*t36*4.0-Lxcm6*Lycm6*dQ1*dQ4*m6*t3*t5*t7*t9*t36*4.0-Lxcm6*Lycm6*dQ2*dQ3*m6*t5*t6*t10*t11*t34*4.0+Lxcm6*Lycm6*dQ1*dQ2*m6*t2*t8*t10*t34*t36*4.0+Lxcm6*Lycm6*dQ1*dQ2*m6*t3*t7*t10*t34*t36*4.0+Lxcm6*Lycm6*dQ1*dQ3*m6*t2*t8*t10*t34*t36*4.0+Lxcm6*Lycm6*dQ1*dQ3*m6*t3*t7*t10*t34*t36*4.0;
et404 = Lx4*Lz6*dQ1*dQ2*m6*t2*t4*t5*t8*t9*-2.0-Lx4*Lz6*dQ1*dQ2*m6*t3*t4*t5*t7*t9*2.0-Lx4*Lz6*dQ1*dQ3*m6*t2*t4*t5*t8*t9*2.0-Lx4*Lz6*dQ1*dQ3*m6*t3*t4*t5*t7*t9*2.0-Lx4*Lzcm5*dQ1*dQ2*m5*t2*t4*t5*t8*t9*2.0-Lx4*Lzcm5*dQ1*dQ2*m5*t3*t4*t5*t7*t9*2.0-Lx4*Lzcm5*dQ1*dQ3*m5*t2*t4*t5*t8*t9*2.0-Lx4*Lzcm5*dQ1*dQ3*m5*t3*t4*t5*t7*t9*2.0-Lx4*Lzcm6*dQ1*dQ2*m6*t2*t4*t5*t8*t9*2.0-Lx4*Lzcm6*dQ1*dQ2*m6*t3*t4*t5*t7*t9*2.0-Lx4*Lzcm6*dQ1*dQ3*m6*t2*t4*t5*t8*t9*2.0-Lx4*Lzcm6*dQ1*dQ3*m6*t3*t4*t5*t7*t9*2.0+Lxcm6*Lz6*dQ1*dQ2*m6*t2*t4*t6*t8*t9*2.0+Lxcm6*Lz6*dQ1*dQ2*m6*t3*t4*t6*t7*t9*2.0+Lxcm6*Lz6*dQ1*dQ3*m6*t2*t4*t6*t8*t9*2.0;
et405 = Lxcm6*Lz6*dQ1*dQ3*m6*t3*t4*t6*t7*t9*2.0+Lxcm6*Lz6*dQ1*dQ6*m6*t2*t4*t6*t8*t10*2.0+Lxcm6*Lz6*dQ1*dQ6*m6*t3*t4*t6*t7*t10*2.0-Lxcm6*Lz6*dQ1*dQ4*m6*t2*t8*t9*t10*t11*2.0-Lxcm6*Lz6*dQ1*dQ4*m6*t3*t7*t9*t10*t11*2.0-Lxcm6*Lz6*dQ1*dQ2*m6*t2*t5*t8*t11*t34*2.0-Lxcm6*Lz6*dQ1*dQ2*m6*t3*t5*t7*t11*t34*2.0-Lxcm6*Lz6*dQ1*dQ3*m6*t2*t5*t8*t11*t34*2.0-Lxcm6*Lz6*dQ1*dQ3*m6*t3*t5*t7*t11*t34*2.0-Lxcm5*Lzcm5*dQ1*dQ2*m5*t2*t3*t5*t9*t10*4.0-Lxcm5*Lzcm5*dQ1*dQ3*m5*t2*t3*t5*t9*t10*4.0+Lxcm5*Lzcm5*dQ1*dQ4*m5*t2*t4*t5*t8*t10*4.0+Lxcm5*Lzcm5*dQ1*dQ4*m5*t3*t4*t5*t7*t10*4.0+Lxcm6*Lzcm6*dQ1*dQ2*m6*t2*t4*t6*t8*t9*2.0+Lxcm6*Lzcm6*dQ1*dQ2*m6*t3*t4*t6*t7*t9*2.0+Lxcm6*Lzcm6*dQ1*dQ3*m6*t2*t4*t6*t8*t9*2.0;
et406 = Lxcm6*Lzcm6*dQ1*dQ3*m6*t3*t4*t6*t7*t9*2.0+Lxcm6*Lzcm6*dQ1*dQ6*m6*t2*t4*t6*t8*t10*2.0+Lxcm6*Lzcm6*dQ1*dQ6*m6*t3*t4*t6*t7*t10*2.0+Lxcm5*Lzcm5*dQ1*dQ2*m5*t5*t7*t8*t9*t10*4.0+Lxcm5*Lzcm5*dQ1*dQ3*m5*t5*t7*t8*t9*t10*4.0-Lxcm6*Lzcm6*dQ1*dQ4*m6*t2*t8*t9*t10*t11*2.0-Lxcm6*Lzcm6*dQ1*dQ4*m6*t3*t7*t9*t10*t11*2.0-Lxcm5*Lzcm5*dQ1*dQ2*m5*t2*t4*t8*t9*t35*4.0-Lxcm5*Lzcm5*dQ1*dQ2*m5*t3*t4*t7*t9*t35*4.0-Lxcm5*Lzcm5*dQ1*dQ3*m5*t2*t4*t8*t9*t35*4.0-Lxcm5*Lzcm5*dQ1*dQ3*m5*t3*t4*t7*t9*t35*4.0-Lxcm6*Lzcm6*dQ1*dQ2*m6*t2*t5*t8*t11*t34*2.0-Lxcm6*Lzcm6*dQ1*dQ2*m6*t3*t5*t7*t11*t34*2.0-Lxcm6*Lzcm6*dQ1*dQ3*m6*t2*t5*t8*t11*t34*2.0-Lxcm6*Lzcm6*dQ1*dQ3*m6*t3*t5*t7*t11*t34*2.0;
et407 = Lycm6*Lz6*dQ1*dQ2*m6*t2*t4*t8*t9*t11*-2.0-Lycm6*Lz6*dQ1*dQ2*m6*t3*t4*t7*t9*t11*2.0-Lycm6*Lz6*dQ1*dQ3*m6*t2*t4*t8*t9*t11*2.0-Lycm6*Lz6*dQ1*dQ3*m6*t3*t4*t7*t9*t11*2.0-Lycm6*Lz6*dQ1*dQ4*m6*t2*t6*t8*t9*t10*2.0-Lycm6*Lz6*dQ1*dQ4*m6*t3*t6*t7*t9*t10*2.0-Lycm6*Lz6*dQ1*dQ6*m6*t2*t4*t8*t10*t11*2.0-Lycm6*Lz6*dQ1*dQ6*m6*t3*t4*t7*t10*t11*2.0-Lycm6*Lz6*dQ1*dQ2*m6*t2*t5*t6*t8*t34*2.0-Lycm6*Lz6*dQ1*dQ2*m6*t3*t5*t6*t7*t34*2.0-Lycm6*Lz6*dQ1*dQ3*m6*t2*t5*t6*t8*t34*2.0-Lycm6*Lz6*dQ1*dQ3*m6*t3*t5*t6*t7*t34*2.0-Lycm6*Lzcm6*dQ1*dQ2*m6*t2*t4*t8*t9*t11*2.0-Lycm6*Lzcm6*dQ1*dQ2*m6*t3*t4*t7*t9*t11*2.0-Lycm6*Lzcm6*dQ1*dQ3*m6*t2*t4*t8*t9*t11*2.0;
et408 = Lycm6*Lzcm6*dQ1*dQ3*m6*t3*t4*t7*t9*t11*-2.0-Lycm6*Lzcm6*dQ1*dQ4*m6*t2*t6*t8*t9*t10*2.0-Lycm6*Lzcm6*dQ1*dQ4*m6*t3*t6*t7*t9*t10*2.0-Lycm6*Lzcm6*dQ1*dQ6*m6*t2*t4*t8*t10*t11*2.0-Lycm6*Lzcm6*dQ1*dQ6*m6*t3*t4*t7*t10*t11*2.0-Lycm6*Lzcm6*dQ1*dQ2*m6*t2*t5*t6*t8*t34*2.0-Lycm6*Lzcm6*dQ1*dQ2*m6*t3*t5*t6*t7*t34*2.0-Lycm6*Lzcm6*dQ1*dQ3*m6*t2*t5*t6*t8*t34*2.0-Lycm6*Lzcm6*dQ1*dQ3*m6*t3*t5*t6*t7*t34*2.0-Ixx6*dQ1*dQ2*t2*t4*t5*t8*t9*t10*t36*2.0-Ixx6*dQ1*dQ2*t3*t4*t5*t7*t9*t10*t36*2.0-Ixx6*dQ1*dQ3*t2*t4*t5*t8*t9*t10*t36*2.0-Ixx6*dQ1*dQ3*t3*t4*t5*t7*t9*t10*t36*2.0+Iyy6*dQ1*dQ2*t2*t4*t5*t8*t9*t10*t36*2.0+Iyy6*dQ1*dQ2*t3*t4*t5*t7*t9*t10*t36*2.0;
et409 = Iyy6*dQ1*dQ3*t2*t4*t5*t8*t9*t10*t36*2.0+Iyy6*dQ1*dQ3*t3*t4*t5*t7*t9*t10*t36*2.0+dQ1*dQ2*m5*t2*t4*t5*t8*t9*t10*t17*2.0+dQ1*dQ2*m5*t3*t4*t5*t7*t9*t10*t17*2.0+dQ1*dQ3*m5*t2*t4*t5*t8*t9*t10*t17*2.0+dQ1*dQ3*m5*t3*t4*t5*t7*t9*t10*t17*2.0+dQ1*dQ2*m6*t2*t4*t5*t8*t9*t10*t21*2.0+dQ1*dQ2*m6*t3*t4*t5*t7*t9*t10*t21*2.0-dQ1*dQ2*m6*t2*t4*t5*t8*t9*t10*t22*2.0-dQ1*dQ2*m6*t3*t4*t5*t7*t9*t10*t22*2.0+dQ1*dQ3*m6*t2*t4*t5*t8*t9*t10*t21*2.0+dQ1*dQ3*m6*t3*t4*t5*t7*t9*t10*t21*2.0-dQ1*dQ3*m6*t2*t4*t5*t8*t9*t10*t22*2.0-dQ1*dQ3*m6*t3*t4*t5*t7*t9*t10*t22*2.0-dQ1*dQ4*m6*t2*t5*t6*t8*t9*t11*t18*2.0-dQ1*dQ4*m6*t3*t5*t6*t7*t9*t11*t18*2.0;
et410 = dQ1*dQ2*m5*t2*t4*t5*t8*t9*t10*t25*-2.0-dQ1*dQ2*m5*t3*t4*t5*t7*t9*t10*t25*2.0-dQ1*dQ3*m5*t2*t4*t5*t8*t9*t10*t25*2.0-dQ1*dQ3*m5*t3*t4*t5*t7*t9*t10*t25*2.0-dQ1*dQ2*m6*t2*t4*t5*t8*t9*t10*t26*2.0-dQ1*dQ2*m6*t3*t4*t5*t7*t9*t10*t26*2.0+dQ1*dQ4*m6*t2*t5*t6*t8*t9*t11*t21*2.0+dQ1*dQ4*m6*t3*t5*t6*t7*t9*t11*t21*2.0-dQ1*dQ3*m6*t2*t4*t5*t8*t9*t10*t26*2.0-dQ1*dQ3*m6*t3*t4*t5*t7*t9*t10*t26*2.0+dQ1*dQ2*m6*t2*t6*t8*t10*t11*t18*t34*2.0+dQ1*dQ2*m6*t3*t6*t7*t10*t11*t18*t34*2.0+dQ1*dQ3*m6*t2*t6*t8*t10*t11*t18*t34*2.0+dQ1*dQ3*m6*t3*t6*t7*t10*t11*t18*t34*2.0-dQ1*dQ2*m6*t2*t6*t8*t10*t11*t21*t34*2.0;
et411 = dQ1*dQ2*m6*t3*t6*t7*t10*t11*t21*t34*-2.0-dQ1*dQ3*m6*t2*t6*t8*t10*t11*t21*t34*2.0-dQ1*dQ3*m6*t3*t6*t7*t10*t11*t21*t34*2.0+dQ1*dQ2*m6*t2*t4*t5*t8*t9*t10*t18*t36*2.0+dQ1*dQ2*m6*t3*t4*t5*t7*t9*t10*t18*t36*2.0+dQ1*dQ3*m6*t2*t4*t5*t8*t9*t10*t18*t36*2.0+dQ1*dQ3*m6*t3*t4*t5*t7*t9*t10*t18*t36*2.0-dQ1*dQ2*m6*t2*t4*t5*t8*t9*t10*t21*t36*2.0-dQ1*dQ2*m6*t3*t4*t5*t7*t9*t10*t21*t36*2.0-dQ1*dQ3*m6*t2*t4*t5*t8*t9*t10*t21*t36*2.0-dQ1*dQ3*m6*t3*t4*t5*t7*t9*t10*t21*t36*2.0+Lx4*Lxcm6*dQ1*dQ2*m6*t2*t4*t6*t8*t9*t10*2.0+Lx4*Lxcm6*dQ1*dQ2*m6*t3*t4*t6*t7*t9*t10*2.0+Lx4*Lxcm6*dQ1*dQ3*m6*t2*t4*t6*t8*t9*t10*2.0+Lx4*Lxcm6*dQ1*dQ3*m6*t3*t4*t6*t7*t9*t10*2.0;
et412 = Lx4*Lycm6*dQ1*dQ2*m6*t2*t4*t8*t9*t10*t11*-2.0-Lx4*Lycm6*dQ1*dQ2*m6*t3*t4*t7*t9*t10*t11*2.0-Lx4*Lycm6*dQ1*dQ3*m6*t2*t4*t8*t9*t10*t11*2.0-Lx4*Lycm6*dQ1*dQ3*m6*t3*t4*t7*t9*t10*t11*2.0-Lxcm6*Lycm6*dQ1*dQ4*m6*t2*t3*t5*t6*t10*t11*4.0-Lxcm6*Lycm6*dQ1*dQ6*m6*t2*t4*t5*t6*t8*t11*4.0-Lxcm6*Lycm6*dQ1*dQ6*m6*t3*t4*t5*t6*t7*t11*4.0+Lxcm6*Lycm6*dQ1*dQ4*m6*t5*t6*t7*t8*t10*t11*4.0+Lxcm6*Lycm6*dQ1*dQ2*m6*t2*t3*t6*t9*t11*t35*4.0+Lxcm6*Lycm6*dQ1*dQ3*m6*t2*t3*t6*t9*t11*t35*4.0-Lxcm6*Lycm6*dQ1*dQ4*m6*t2*t4*t6*t8*t11*t35*4.0-Lxcm6*Lycm6*dQ1*dQ4*m6*t3*t4*t6*t7*t11*t35*4.0-Lxcm6*Lycm6*dQ1*dQ2*m6*t6*t7*t8*t9*t11*t35*4.0-Lxcm6*Lycm6*dQ1*dQ3*m6*t6*t7*t8*t9*t11*t35*4.0;
et413 = Lxcm6*Lz6*dQ1*dQ2*m6*t2*t3*t5*t6*t9*t10*-4.0-Lxcm6*Lz6*dQ1*dQ3*m6*t2*t3*t5*t6*t9*t10*4.0+Lxcm6*Lz6*dQ1*dQ4*m6*t2*t4*t5*t6*t8*t10*4.0+Lxcm6*Lz6*dQ1*dQ4*m6*t3*t4*t5*t6*t7*t10*4.0+Lxcm6*Lz6*dQ1*dQ2*m6*t5*t6*t7*t8*t9*t10*4.0+Lxcm6*Lz6*dQ1*dQ3*m6*t5*t6*t7*t8*t9*t10*4.0-Lxcm6*Lz6*dQ1*dQ2*m6*t2*t4*t6*t8*t9*t35*4.0-Lxcm6*Lz6*dQ1*dQ2*m6*t3*t4*t6*t7*t9*t35*4.0-Lxcm6*Lz6*dQ1*dQ3*m6*t2*t4*t6*t8*t9*t35*4.0-Lxcm6*Lz6*dQ1*dQ3*m6*t3*t4*t6*t7*t9*t35*4.0-Lxcm6*Lzcm6*dQ1*dQ2*m6*t2*t3*t5*t6*t9*t10*4.0-Lxcm6*Lzcm6*dQ1*dQ3*m6*t2*t3*t5*t6*t9*t10*4.0+Lxcm6*Lzcm6*dQ1*dQ4*m6*t2*t4*t5*t6*t8*t10*4.0+Lxcm6*Lzcm6*dQ1*dQ4*m6*t3*t4*t5*t6*t7*t10*4.0;
et414 = Lxcm6*Lzcm6*dQ1*dQ2*m6*t5*t6*t7*t8*t9*t10*4.0+Lxcm6*Lzcm6*dQ1*dQ3*m6*t5*t6*t7*t8*t9*t10*4.0-Lxcm6*Lzcm6*dQ1*dQ2*m6*t2*t4*t6*t8*t9*t35*4.0-Lxcm6*Lzcm6*dQ1*dQ2*m6*t3*t4*t6*t7*t9*t35*4.0-Lxcm6*Lzcm6*dQ1*dQ3*m6*t2*t4*t6*t8*t9*t35*4.0-Lxcm6*Lzcm6*dQ1*dQ3*m6*t3*t4*t6*t7*t9*t35*4.0+Lycm6*Lz6*dQ1*dQ2*m6*t2*t3*t5*t9*t10*t11*4.0+Lycm6*Lz6*dQ1*dQ3*m6*t2*t3*t5*t9*t10*t11*4.0-Lycm6*Lz6*dQ1*dQ4*m6*t2*t4*t5*t8*t10*t11*4.0-Lycm6*Lz6*dQ1*dQ4*m6*t3*t4*t5*t7*t10*t11*4.0-Lycm6*Lz6*dQ1*dQ2*m6*t5*t7*t8*t9*t10*t11*4.0-Lycm6*Lz6*dQ1*dQ3*m6*t5*t7*t8*t9*t10*t11*4.0+Lycm6*Lz6*dQ1*dQ2*m6*t2*t4*t8*t9*t11*t35*4.0+Lycm6*Lz6*dQ1*dQ2*m6*t3*t4*t7*t9*t11*t35*4.0;
et415 = Lycm6*Lz6*dQ1*dQ3*m6*t2*t4*t8*t9*t11*t35*4.0+Lycm6*Lz6*dQ1*dQ3*m6*t3*t4*t7*t9*t11*t35*4.0+Lycm6*Lzcm6*dQ1*dQ2*m6*t2*t3*t5*t9*t10*t11*4.0+Lycm6*Lzcm6*dQ1*dQ3*m6*t2*t3*t5*t9*t10*t11*4.0-Lycm6*Lzcm6*dQ1*dQ4*m6*t2*t4*t5*t8*t10*t11*4.0-Lycm6*Lzcm6*dQ1*dQ4*m6*t3*t4*t5*t7*t10*t11*4.0-Lycm6*Lzcm6*dQ1*dQ2*m6*t5*t7*t8*t9*t10*t11*4.0-Lycm6*Lzcm6*dQ1*dQ3*m6*t5*t7*t8*t9*t10*t11*4.0+Lycm6*Lzcm6*dQ1*dQ2*m6*t2*t4*t8*t9*t11*t35*4.0+Lycm6*Lzcm6*dQ1*dQ2*m6*t3*t4*t7*t9*t11*t35*4.0+Lycm6*Lzcm6*dQ1*dQ3*m6*t2*t4*t8*t9*t11*t35*4.0+Lycm6*Lzcm6*dQ1*dQ3*m6*t3*t4*t7*t9*t11*t35*4.0-Lz6*Lzcm6*dQ1*dQ2*m6*t2*t4*t5*t8*t9*t10*4.0-Lz6*Lzcm6*dQ1*dQ2*m6*t3*t4*t5*t7*t9*t10*4.0;
et416 = Lz6*Lzcm6*dQ1*dQ3*m6*t2*t4*t5*t8*t9*t10*-4.0-Lz6*Lzcm6*dQ1*dQ3*m6*t3*t4*t5*t7*t9*t10*4.0-Lxcm6*Lycm6*dQ1*dQ2*m6*t2*t4*t5*t6*t8*t9*t10*t11*4.0-Lxcm6*Lycm6*dQ1*dQ2*m6*t3*t4*t5*t6*t7*t9*t10*t11*4.0-Lxcm6*Lycm6*dQ1*dQ3*m6*t2*t4*t5*t6*t8*t9*t10*t11*4.0-Lxcm6*Lycm6*dQ1*dQ3*m6*t3*t4*t5*t6*t7*t9*t10*t11*4.0;
et417 = t9*t10*t92+t9*t10*t93+t9*t10*t100+t9*t10*t101+t9*t10*t108+t9*t10*t109+t9*t10*t115+t9*t10*t116+t9*t10*t117+t9*t10*t118+t9*t10*t127+t9*t10*t128+t9*t10*t171+t9*t10*t172+t9*t10*t265+t9*t10*t266+t9*t10*t349+t9*t10*t350+t9*t10*t473+t9*t10*t474+t9*t10*t494+t9*t10*t495+t9*t10*t599+t9*t10*t600+t9*t10*t694+t9*t10*t695+t9*t10*t967+t9*t10*t968+t9*t10*t1092+t9*t10*t1093-t9*t10*t36*t92*2.0-t9*t10*t36*t93*2.0-Ixx6*dQ4*dQ5*t10+Iyy6*dQ4*dQ5*t10-Izz6*dQ4*dQ5*t10-Ixx6*dQ2*dQ4*t4*t10+Ixx6*dQ2*dQ5*t5*t9-Ixx6*dQ3*dQ4*t4*t10+Ixx6*dQ3*dQ5*t5*t9+Ixx6*dQ4*dQ5*t10*t36*2.0+Iyy6*dQ2*dQ4*t4*t10;
et418 = -Iyy6*dQ2*dQ5*t5*t9+Iyy6*dQ3*dQ4*t4*t10-Iyy6*dQ3*dQ5*t5*t9-Iyy6*dQ4*dQ5*t10*t36*2.0+Izz6*dQ2*dQ4*t4*t10+Izz6*dQ2*dQ5*t5*t9+Izz6*dQ3*dQ4*t4*t10+Izz6*dQ3*dQ5*t5*t9-dQ4*dQ5*m6*t10*t21*2.0+t4*t5*t6*t10*t11*t84*2.0+t4*t5*t6*t10*t11*t85*2.0-t4*t5*t6*t10*t11*t92*2.0-t4*t5*t6*t10*t11*t93*2.0-Lxcm6*Lycm6*dQ2*dQ5*m6*t4*2.0-Lxcm6*Lycm6*dQ3*dQ5*m6*t4*2.0-Lxcm6*Lycm6*dQ2*dQ3*m6*t34*2.0+Lxcm6*Lycm6*dQ2*dQ3*m6*t35*2.0+Ixx6*dQ1*dQ2*t2*t5*t8+Ixx6*dQ1*dQ2*t3*t5*t7+Ixx6*dQ1*dQ3*t2*t5*t8+Ixx6*dQ1*dQ3*t3*t5*t7-Ixx6*dQ1*dQ5*t2*t3*t10+Ixx6*dQ2*dQ3*t4*t5*t9*2.0-Ixx6*dQ2*dQ5*t4*t6*t11*2.0-Ixx6*dQ3*dQ5*t4*t6*t11*2.0;
et419 = Ixx6*dQ1*dQ5*t7*t8*t10-Ixx6*dQ2*dQ3*t6*t11*t34*2.0+Ixx6*dQ2*dQ4*t4*t10*t36*2.0+Ixx6*dQ2*dQ3*t6*t11*t35*2.0-Ixx6*dQ2*dQ5*t5*t9*t36*2.0+Ixx6*dQ3*dQ4*t4*t10*t36*2.0-Ixx6*dQ3*dQ5*t5*t9*t36*2.0-Iyy6*dQ1*dQ2*t2*t5*t8-Iyy6*dQ1*dQ2*t3*t5*t7-Iyy6*dQ1*dQ3*t2*t5*t8-Iyy6*dQ1*dQ3*t3*t5*t7+Iyy6*dQ1*dQ5*t2*t3*t10-Iyy6*dQ2*dQ3*t4*t5*t9*2.0+Iyy6*dQ2*dQ5*t4*t6*t11*2.0+Iyy6*dQ3*dQ5*t4*t6*t11*2.0-Iyy6*dQ1*dQ5*t7*t8*t10+Iyy6*dQ2*dQ3*t6*t11*t34*2.0-Iyy6*dQ2*dQ4*t4*t10*t36*2.0-Iyy6*dQ2*dQ3*t6*t11*t35*2.0+Iyy6*dQ2*dQ5*t5*t9*t36*2.0-Iyy6*dQ3*dQ4*t4*t10*t36*2.0+Iyy6*dQ3*dQ5*t5*t9*t36*2.0-Izz6*dQ1*dQ2*t2*t5*t8;
et420 = -Izz6*dQ1*dQ2*t3*t5*t7-Izz6*dQ1*dQ3*t2*t5*t8-Izz6*dQ1*dQ3*t3*t5*t7-Izz6*dQ1*dQ5*t2*t3*t10+Izz6*dQ1*dQ5*t7*t8*t10+dQ2*dQ4*m6*t4*t10*t18*2.0+dQ3*dQ4*m6*t4*t10*t18*2.0+dQ2*dQ5*m6*t5*t9*t21*2.0+dQ3*dQ5*m6*t5*t9*t21*2.0-dQ4*dQ5*m6*t10*t18*t36*2.0+dQ4*dQ5*m6*t10*t21*t36*2.0+Lx3*Lxcm6*dQ2*dQ3*m6*t6*t9*2.0-Lx3*Lycm6*dQ2*dQ3*m6*t9*t11*2.0+Lxcm6*Lycm6*dQ1*dQ4*m6*t2*t3*2.0-Lxcm6*Lycm6*dQ1*dQ4*m6*t7*t8*2.0+Lxcm6*Lycm6*dQ2*dQ5*m6*t4*t36*4.0+Lxcm6*Lycm6*dQ3*dQ5*m6*t4*t36*4.0-Lxcm6*Lycm6*dQ2*dQ3*m6*t34*t35*2.0+Lxcm6*Lycm6*dQ2*dQ3*m6*t34*t36*4.0-Lxcm6*Lycm6*dQ2*dQ3*m6*t35*t36*4.0+Lxcm6*Lz6*dQ4*dQ5*m6*t5*t6*2.0+Lxcm6*Lz6*dQ2*dQ4*m6*t9*t11*2.0;
et421 = Lxcm6*Lz6*dQ3*dQ4*m6*t9*t11*2.0+Lxcm6*Lzcm6*dQ4*dQ5*m6*t5*t6*2.0+Lxcm6*Lzcm6*dQ2*dQ4*m6*t9*t11*2.0+Lxcm6*Lzcm6*dQ3*dQ4*m6*t9*t11*2.0+Lycm6*Lz6*dQ2*dQ4*m6*t6*t9*2.0+Lycm6*Lz6*dQ3*dQ4*m6*t6*t9*2.0-Lycm6*Lz6*dQ4*dQ5*m6*t5*t11*2.0+Lycm6*Lzcm6*dQ2*dQ4*m6*t6*t9*2.0+Lycm6*Lzcm6*dQ3*dQ4*m6*t6*t9*2.0-Lycm6*Lzcm6*dQ4*dQ5*m6*t5*t11*2.0-Ixx6*dQ1*dQ2*t2*t3*t4*t10-Ixx6*dQ1*dQ3*t2*t3*t4*t10-Ixx6*dQ1*dQ5*t2*t4*t5*t8-Ixx6*dQ1*dQ5*t3*t4*t5*t7+Ixx6*dQ1*dQ4*t2*t3*t6*t11*2.0+Ixx6*dQ1*dQ2*t4*t7*t8*t10+Ixx6*dQ1*dQ3*t4*t7*t8*t10-Ixx6*dQ1*dQ4*t6*t7*t8*t11*2.0-Ixx6*dQ1*dQ2*t2*t5*t8*t34*2.0-Ixx6*dQ1*dQ2*t3*t5*t7*t34*2.0-Ixx6*dQ1*dQ3*t2*t5*t8*t34*2.0;
et422 = Ixx6*dQ1*dQ3*t3*t5*t7*t34*-2.0-Ixx6*dQ1*dQ2*t2*t5*t8*t36*2.0-Ixx6*dQ1*dQ2*t3*t5*t7*t36*2.0-Ixx6*dQ1*dQ3*t2*t5*t8*t36*2.0-Ixx6*dQ1*dQ3*t3*t5*t7*t36*2.0+Ixx6*dQ1*dQ5*t2*t3*t10*t36*2.0-Ixx6*dQ2*dQ3*t4*t5*t9*t36*4.0-Ixx6*dQ1*dQ5*t7*t8*t10*t36*2.0-Ixx6*dQ2*dQ3*t6*t11*t34*t35*2.0+Iyy6*dQ1*dQ2*t2*t3*t4*t10+Iyy6*dQ1*dQ3*t2*t3*t4*t10+Iyy6*dQ1*dQ5*t2*t4*t5*t8+Iyy6*dQ1*dQ5*t3*t4*t5*t7-Iyy6*dQ1*dQ4*t2*t3*t6*t11*2.0-Iyy6*dQ1*dQ2*t4*t7*t8*t10-Iyy6*dQ1*dQ3*t4*t7*t8*t10+Iyy6*dQ1*dQ4*t6*t7*t8*t11*2.0+Iyy6*dQ1*dQ2*t2*t5*t8*t34*2.0+Iyy6*dQ1*dQ2*t3*t5*t7*t34*2.0+Iyy6*dQ1*dQ3*t2*t5*t8*t34*2.0+Iyy6*dQ1*dQ3*t3*t5*t7*t34*2.0;
et423 = Iyy6*dQ1*dQ2*t2*t5*t8*t36*2.0+Iyy6*dQ1*dQ2*t3*t5*t7*t36*2.0+Iyy6*dQ1*dQ3*t2*t5*t8*t36*2.0+Iyy6*dQ1*dQ3*t3*t5*t7*t36*2.0-Iyy6*dQ1*dQ5*t2*t3*t10*t36*2.0+Iyy6*dQ2*dQ3*t4*t5*t9*t36*4.0+Iyy6*dQ1*dQ5*t7*t8*t10*t36*2.0+Iyy6*dQ2*dQ3*t6*t11*t34*t35*2.0-Izz6*dQ1*dQ2*t2*t3*t4*t10-Izz6*dQ1*dQ3*t2*t3*t4*t10-Izz6*dQ1*dQ5*t2*t4*t5*t8-Izz6*dQ1*dQ5*t3*t4*t5*t7+Izz6*dQ1*dQ2*t4*t7*t8*t10+Izz6*dQ1*dQ3*t4*t7*t8*t10-dQ1*dQ2*m6*t2*t5*t8*t18*2.0-dQ1*dQ2*m6*t3*t5*t7*t18*2.0-dQ1*dQ3*m6*t2*t5*t8*t18*2.0-dQ1*dQ3*m6*t3*t5*t7*t18*2.0-dQ2*dQ3*m6*t4*t5*t9*t18*2.0-dQ1*dQ5*m6*t2*t3*t10*t21*2.0+dQ2*dQ3*m6*t4*t5*t9*t21*2.0;
et424 = dQ2*dQ5*m6*t4*t6*t11*t18*2.0+dQ3*dQ5*m6*t4*t6*t11*t18*2.0-dQ2*dQ5*m6*t4*t6*t11*t21*2.0-dQ3*dQ5*m6*t4*t6*t11*t21*2.0+dQ1*dQ5*m6*t7*t8*t10*t21*2.0+dQ2*dQ3*m6*t6*t11*t18*t34*2.0-dQ2*dQ4*m6*t4*t10*t18*t36*2.0-dQ2*dQ3*m6*t6*t11*t18*t35*2.0+dQ2*dQ5*m6*t5*t9*t18*t36*2.0-dQ3*dQ4*m6*t4*t10*t18*t36*2.0+dQ3*dQ5*m6*t5*t9*t18*t36*2.0-dQ2*dQ3*m6*t6*t11*t21*t34*2.0+dQ2*dQ4*m6*t4*t10*t21*t36*2.0+dQ2*dQ3*m6*t6*t11*t21*t35*2.0-dQ2*dQ5*m6*t5*t9*t21*t36*2.0+dQ3*dQ4*m6*t4*t10*t21*t36*2.0-dQ3*dQ5*m6*t5*t9*t21*t36*2.0-Lx2*Lxcm6*dQ1*dQ2*m6*t4*t6*t7*2.0+Lx3*Lxcm6*dQ2*dQ3*m6*t4*t5*t11*2.0+Lx4*Lxcm6*dQ2*dQ3*m6*t4*t6*t9*2.0;
et425 = Lx4*Lxcm6*dQ2*dQ3*m6*t5*t11*t34*2.0+Lx3*Lycm6*dQ2*dQ3*m6*t4*t5*t6*2.0+Lx2*Lycm6*dQ1*dQ2*m6*t4*t7*t11*2.0-Lx4*Lycm6*dQ2*dQ3*m6*t4*t9*t11*2.0+Lx4*Lycm6*dQ2*dQ3*m6*t5*t6*t34*2.0-Lxcm6*Lycm6*dQ1*dQ5*m6*t2*t8*t9*2.0-Lxcm6*Lycm6*dQ1*dQ5*m6*t3*t7*t9*2.0-Lxcm6*Lycm6*dQ2*dQ4*m6*t5*t9*t10*2.0-Lxcm6*Lycm6*dQ3*dQ4*m6*t5*t9*t10*2.0+Lxcm6*Lycm6*dQ4*dQ5*m6*t6*t10*t11*4.0-Lxcm6*Lycm6*dQ1*dQ4*m6*t2*t3*t35*2.0-Lxcm6*Lycm6*dQ1*dQ4*m6*t2*t3*t36*4.0+Lxcm6*Lycm6*dQ1*dQ4*m6*t7*t8*t35*2.0+Lxcm6*Lycm6*dQ1*dQ4*m6*t7*t8*t36*4.0+Lxcm6*Lycm6*dQ2*dQ3*m6*t34*t35*t36*4.0-Lxcm6*Lz6*dQ2*dQ3*m6*t5*t10*t11*2.0-Lxcm6*Lz6*dQ2*dQ4*m6*t9*t11*t35*2.0-Lxcm6*Lz6*dQ3*dQ4*m6*t9*t11*t35*2.0;
et426 = Lxcm6*Lzcm6*dQ2*dQ3*m6*t5*t10*t11*-2.0-Lxcm6*Lzcm6*dQ2*dQ4*m6*t9*t11*t35*2.0-Lxcm6*Lzcm6*dQ3*dQ4*m6*t9*t11*t35*2.0-Lycm6*Lz6*dQ2*dQ3*m6*t5*t6*t10*2.0-Lycm6*Lz6*dQ2*dQ5*m6*t9*t10*t11*2.0-Lycm6*Lz6*dQ3*dQ5*m6*t9*t10*t11*2.0-Lycm6*Lz6*dQ2*dQ4*m6*t6*t9*t35*2.0-Lycm6*Lz6*dQ3*dQ4*m6*t6*t9*t35*2.0-Lycm6*Lzcm6*dQ2*dQ3*m6*t5*t6*t10*2.0-Lycm6*Lzcm6*dQ2*dQ5*m6*t9*t10*t11*2.0-Lycm6*Lzcm6*dQ3*dQ5*m6*t9*t10*t11*2.0-Lycm6*Lzcm6*dQ2*dQ4*m6*t6*t9*t35*2.0-Lycm6*Lzcm6*dQ3*dQ4*m6*t6*t9*t35*2.0-Ixx6*dQ1*dQ5*t2*t6*t8*t9*t11*2.0-Ixx6*dQ1*dQ5*t3*t6*t7*t9*t11*2.0-Ixx6*dQ2*dQ4*t5*t6*t9*t10*t11*2.0-Ixx6*dQ3*dQ4*t5*t6*t9*t10*t11*2.0+Ixx6*dQ1*dQ2*t2*t3*t4*t10*t36*2.0;
et427 = Ixx6*dQ1*dQ3*t2*t3*t4*t10*t36*2.0+Ixx6*dQ1*dQ5*t2*t4*t5*t8*t36*2.0+Ixx6*dQ1*dQ5*t3*t4*t5*t7*t36*2.0-Ixx6*dQ1*dQ4*t2*t3*t6*t11*t35*2.0-Ixx6*dQ1*dQ2*t4*t7*t8*t10*t36*2.0-Ixx6*dQ1*dQ3*t4*t7*t8*t10*t36*2.0+Ixx6*dQ1*dQ4*t6*t7*t8*t11*t35*2.0+Ixx6*dQ1*dQ2*t2*t5*t8*t34*t36*4.0+Ixx6*dQ1*dQ2*t3*t5*t7*t34*t36*4.0+Ixx6*dQ1*dQ3*t2*t5*t8*t34*t36*4.0+Ixx6*dQ1*dQ3*t3*t5*t7*t34*t36*4.0+Iyy6*dQ1*dQ5*t2*t6*t8*t9*t11*2.0+Iyy6*dQ1*dQ5*t3*t6*t7*t9*t11*2.0-Iyy6*dQ1*dQ2*t2*t3*t4*t10*t36*2.0-Iyy6*dQ1*dQ3*t2*t3*t4*t10*t36*2.0-Iyy6*dQ1*dQ5*t2*t4*t5*t8*t36*2.0-Iyy6*dQ1*dQ5*t3*t4*t5*t7*t36*2.0+Iyy6*dQ1*dQ4*t2*t3*t6*t11*t35*2.0+Iyy6*dQ1*dQ2*t4*t7*t8*t10*t36*2.0;
et428 = Iyy6*dQ1*dQ3*t4*t7*t8*t10*t36*2.0-Iyy6*dQ1*dQ4*t6*t7*t8*t11*t35*2.0-Iyy6*dQ1*dQ2*t2*t5*t8*t34*t36*4.0-Iyy6*dQ1*dQ2*t3*t5*t7*t34*t36*4.0-Iyy6*dQ1*dQ3*t2*t5*t8*t34*t36*4.0-Iyy6*dQ1*dQ3*t3*t5*t7*t34*t36*4.0-dQ1*dQ2*m6*t2*t3*t4*t10*t21*2.0-dQ1*dQ3*m6*t2*t3*t4*t10*t21*2.0-dQ1*dQ4*m6*t2*t3*t6*t11*t18*2.0-dQ1*dQ5*m6*t2*t4*t5*t8*t21*2.0-dQ1*dQ5*m6*t3*t4*t5*t7*t21*2.0+dQ1*dQ4*m6*t2*t3*t6*t11*t21*2.0+dQ1*dQ2*m6*t4*t7*t8*t10*t21*2.0+dQ1*dQ3*m6*t4*t7*t8*t10*t21*2.0+dQ1*dQ4*m6*t6*t7*t8*t11*t18*2.0-dQ1*dQ4*m6*t6*t7*t8*t11*t21*2.0+dQ1*dQ2*m6*t2*t5*t8*t18*t34*2.0+dQ1*dQ2*m6*t3*t5*t7*t18*t34*2.0;
et429 = dQ1*dQ3*m6*t2*t5*t8*t18*t34*2.0+dQ1*dQ3*m6*t3*t5*t7*t18*t34*2.0+dQ1*dQ2*m6*t2*t5*t8*t18*t36*2.0+dQ1*dQ2*m6*t3*t5*t7*t18*t36*2.0-dQ1*dQ2*m6*t2*t5*t8*t21*t34*2.0-dQ1*dQ2*m6*t3*t5*t7*t21*t34*2.0+dQ1*dQ3*m6*t2*t5*t8*t18*t36*2.0+dQ1*dQ3*m6*t3*t5*t7*t18*t36*2.0-dQ1*dQ3*m6*t2*t5*t8*t21*t34*2.0-dQ1*dQ3*m6*t3*t5*t7*t21*t34*2.0-dQ1*dQ2*m6*t2*t5*t8*t21*t36*2.0-dQ1*dQ2*m6*t3*t5*t7*t21*t36*2.0-dQ1*dQ5*m6*t2*t3*t10*t18*t36*2.0-dQ1*dQ3*m6*t2*t5*t8*t21*t36*2.0-dQ1*dQ3*m6*t3*t5*t7*t21*t36*2.0+dQ2*dQ3*m6*t4*t5*t9*t18*t36*4.0+dQ1*dQ5*m6*t2*t3*t10*t21*t36*2.0-dQ2*dQ3*m6*t4*t5*t9*t21*t36*4.0+dQ1*dQ5*m6*t7*t8*t10*t18*t36*2.0;
et430 = dQ1*dQ5*m6*t7*t8*t10*t21*t36*-2.0+dQ2*dQ3*m6*t6*t11*t18*t34*t35*2.0-dQ2*dQ3*m6*t6*t11*t21*t34*t35*2.0-Ixx6*dQ1*dQ2*t2*t4*t6*t8*t9*t11*2.0-Ixx6*dQ1*dQ2*t3*t4*t6*t7*t9*t11*2.0-Ixx6*dQ1*dQ3*t2*t4*t6*t8*t9*t11*2.0-Ixx6*dQ1*dQ3*t3*t4*t6*t7*t9*t11*2.0+Iyy6*dQ1*dQ2*t2*t4*t6*t8*t9*t11*2.0+Iyy6*dQ1*dQ2*t3*t4*t6*t7*t9*t11*2.0+Iyy6*dQ1*dQ3*t2*t4*t6*t8*t9*t11*2.0+Iyy6*dQ1*dQ3*t3*t4*t6*t7*t9*t11*2.0+dQ1*dQ5*m6*t2*t6*t8*t9*t11*t18*2.0+dQ1*dQ5*m6*t3*t6*t7*t9*t11*t18*2.0-dQ1*dQ5*m6*t2*t6*t8*t9*t11*t21*2.0-dQ1*dQ5*m6*t3*t6*t7*t9*t11*t21*2.0-dQ2*dQ4*m6*t5*t6*t9*t10*t11*t21*2.0-dQ3*dQ4*m6*t5*t6*t9*t10*t11*t21*2.0;
et431 = dQ1*dQ2*m6*t2*t3*t4*t10*t18*t36*-2.0-dQ1*dQ3*m6*t2*t3*t4*t10*t18*t36*2.0+dQ1*dQ2*m6*t2*t3*t4*t10*t21*t36*2.0-dQ1*dQ5*m6*t2*t4*t5*t8*t18*t36*2.0-dQ1*dQ5*m6*t3*t4*t5*t7*t18*t36*2.0+dQ1*dQ3*m6*t2*t3*t4*t10*t21*t36*2.0+dQ1*dQ4*m6*t2*t3*t6*t11*t18*t35*2.0+dQ1*dQ5*m6*t2*t4*t5*t8*t21*t36*2.0+dQ1*dQ5*m6*t3*t4*t5*t7*t21*t36*2.0-dQ1*dQ4*m6*t2*t3*t6*t11*t21*t35*2.0+dQ1*dQ2*m6*t4*t7*t8*t10*t18*t36*2.0+dQ1*dQ3*m6*t4*t7*t8*t10*t18*t36*2.0-dQ1*dQ2*m6*t4*t7*t8*t10*t21*t36*2.0-dQ1*dQ3*m6*t4*t7*t8*t10*t21*t36*2.0-dQ1*dQ4*m6*t6*t7*t8*t11*t18*t35*2.0+dQ1*dQ4*m6*t6*t7*t8*t11*t21*t35*2.0-dQ1*dQ2*m6*t2*t5*t8*t18*t34*t36*4.0;
et432 = dQ1*dQ2*m6*t3*t5*t7*t18*t34*t36*-4.0-dQ1*dQ3*m6*t2*t5*t8*t18*t34*t36*4.0-dQ1*dQ3*m6*t3*t5*t7*t18*t34*t36*4.0+dQ1*dQ2*m6*t2*t5*t8*t21*t34*t36*4.0+dQ1*dQ2*m6*t3*t5*t7*t21*t34*t36*4.0+dQ1*dQ3*m6*t2*t5*t8*t21*t34*t36*4.0+dQ1*dQ3*m6*t3*t5*t7*t21*t34*t36*4.0-Lx3*Lxcm6*dQ1*dQ2*m6*t2*t4*t6*t8*2.0-Lx3*Lxcm6*dQ1*dQ2*m6*t3*t4*t6*t7*2.0-Lx3*Lxcm6*dQ1*dQ3*m6*t2*t4*t6*t8*2.0-Lx3*Lxcm6*dQ1*dQ3*m6*t3*t4*t6*t7*2.0+Lx4*Lxcm6*dQ1*dQ4*m6*t2*t3*t5*t11*2.0+Lx2*Lxcm6*dQ1*dQ2*m6*t5*t7*t9*t11*2.0-Lx4*Lxcm6*dQ1*dQ4*m6*t5*t7*t8*t11*2.0-Lx4*Lxcm6*dQ1*dQ2*m6*t2*t6*t8*t34*2.0-Lx4*Lxcm6*dQ1*dQ2*m6*t3*t6*t7*t34*2.0-Lx4*Lxcm6*dQ1*dQ3*m6*t2*t6*t8*t34*2.0;
et433 = Lx4*Lxcm6*dQ1*dQ3*m6*t3*t6*t7*t34*-2.0+Lx4*Lycm6*dQ1*dQ4*m6*t2*t3*t5*t6*2.0+Lx3*Lycm6*dQ1*dQ2*m6*t2*t4*t8*t11*2.0+Lx3*Lycm6*dQ1*dQ2*m6*t3*t4*t7*t11*2.0+Lx2*Lycm6*dQ1*dQ2*m6*t5*t6*t7*t9*2.0+Lx3*Lycm6*dQ1*dQ3*m6*t2*t4*t8*t11*2.0+Lx3*Lycm6*dQ1*dQ3*m6*t3*t4*t7*t11*2.0-Lx4*Lycm6*dQ1*dQ4*m6*t5*t6*t7*t8*2.0+Lx4*Lycm6*dQ1*dQ2*m6*t2*t8*t11*t34*2.0+Lx4*Lycm6*dQ1*dQ2*m6*t3*t7*t11*t34*2.0+Lx4*Lycm6*dQ1*dQ3*m6*t2*t8*t11*t34*2.0+Lx4*Lycm6*dQ1*dQ3*m6*t3*t7*t11*t34*2.0-Lxcm6*Lycm6*dQ1*dQ2*m6*t2*t4*t8*t9*2.0-Lxcm6*Lycm6*dQ1*dQ2*m6*t3*t4*t7*t9*2.0-Lxcm6*Lycm6*dQ1*dQ3*m6*t2*t4*t8*t9*2.0-Lxcm6*Lycm6*dQ1*dQ3*m6*t3*t4*t7*t9*2.0+Lxcm6*Lycm6*dQ2*dQ4*m6*t4*t6*t10*t11*4.0;
et434 = Lxcm6*Lycm6*dQ2*dQ5*m6*t5*t6*t9*t11*-4.0+Lxcm6*Lycm6*dQ3*dQ4*m6*t4*t6*t10*t11*4.0-Lxcm6*Lycm6*dQ3*dQ5*m6*t5*t6*t9*t11*4.0+Lxcm6*Lycm6*dQ1*dQ5*m6*t2*t8*t9*t36*4.0+Lxcm6*Lycm6*dQ1*dQ5*m6*t3*t7*t9*t36*4.0+Lxcm6*Lycm6*dQ1*dQ4*m6*t2*t3*t35*t36*4.0-Lxcm6*Lycm6*dQ1*dQ4*m6*t7*t8*t35*t36*4.0+Lxcm6*Lz6*dQ1*dQ5*m6*t2*t3*t5*t6*2.0-Lxcm6*Lz6*dQ1*dQ4*m6*t2*t4*t8*t11*2.0-Lxcm6*Lz6*dQ1*dQ4*m6*t3*t4*t7*t11*2.0-Lxcm6*Lz6*dQ1*dQ5*m6*t5*t6*t7*t8*2.0+Lxcm6*Lz6*dQ2*dQ3*m6*t4*t6*t9*t10*2.0+Lxcm6*Lz6*dQ2*dQ3*m6*t5*t10*t11*t34*2.0+Lxcm6*Lzcm6*dQ1*dQ5*m6*t2*t3*t5*t6*2.0-Lxcm6*Lzcm6*dQ1*dQ4*m6*t2*t4*t8*t11*2.0-Lxcm6*Lzcm6*dQ1*dQ4*m6*t3*t4*t7*t11*2.0-Lxcm6*Lzcm6*dQ1*dQ5*m6*t5*t6*t7*t8*2.0;
et435 = Lxcm6*Lzcm6*dQ2*dQ3*m6*t4*t6*t9*t10*2.0+Lxcm6*Lzcm6*dQ2*dQ3*m6*t5*t10*t11*t34*2.0-Lycm6*Lz6*dQ1*dQ4*m6*t2*t4*t6*t8*2.0-Lycm6*Lz6*dQ1*dQ4*m6*t3*t4*t6*t7*2.0-Lycm6*Lz6*dQ1*dQ5*m6*t2*t3*t5*t11*2.0+Lycm6*Lz6*dQ1*dQ5*m6*t5*t7*t8*t11*2.0-Lycm6*Lz6*dQ2*dQ3*m6*t4*t9*t10*t11*2.0+Lycm6*Lz6*dQ2*dQ3*m6*t5*t6*t10*t34*2.0-Lycm6*Lzcm6*dQ1*dQ4*m6*t2*t4*t6*t8*2.0-Lycm6*Lzcm6*dQ1*dQ4*m6*t3*t4*t6*t7*2.0-Lycm6*Lzcm6*dQ1*dQ5*m6*t2*t3*t5*t11*2.0+Lycm6*Lzcm6*dQ1*dQ5*m6*t5*t7*t8*t11*2.0-Lycm6*Lzcm6*dQ2*dQ3*m6*t4*t9*t10*t11*2.0+Lycm6*Lzcm6*dQ2*dQ3*m6*t5*t6*t10*t34*2.0+Lx3*Lxcm6*dQ1*dQ2*m6*t2*t5*t8*t9*t11*2.0+Lx3*Lxcm6*dQ1*dQ2*m6*t3*t5*t7*t9*t11*2.0+Lx3*Lxcm6*dQ1*dQ3*m6*t2*t5*t8*t9*t11*2.0;
et436 = Lx3*Lxcm6*dQ1*dQ3*m6*t3*t5*t7*t9*t11*2.0-Lx4*Lxcm6*dQ1*dQ4*m6*t2*t4*t8*t10*t11*2.0-Lx4*Lxcm6*dQ1*dQ4*m6*t3*t4*t7*t10*t11*2.0+Lx3*Lycm6*dQ1*dQ2*m6*t2*t5*t6*t8*t9*2.0+Lx3*Lycm6*dQ1*dQ2*m6*t3*t5*t6*t7*t9*2.0+Lx3*Lycm6*dQ1*dQ3*m6*t2*t5*t6*t8*t9*2.0+Lx3*Lycm6*dQ1*dQ3*m6*t3*t5*t6*t7*t9*2.0-Lx4*Lycm6*dQ1*dQ4*m6*t2*t4*t6*t8*t10*2.0-Lx4*Lycm6*dQ1*dQ4*m6*t3*t4*t6*t7*t10*2.0-Lxcm6*Lycm6*dQ1*dQ2*m6*t2*t3*t5*t9*t10*2.0-Lxcm6*Lycm6*dQ1*dQ3*m6*t2*t3*t5*t9*t10*2.0+Lxcm6*Lycm6*dQ1*dQ4*m6*t2*t4*t5*t8*t10*2.0+Lxcm6*Lycm6*dQ1*dQ4*m6*t3*t4*t5*t7*t10*2.0-Lxcm6*Lycm6*dQ1*dQ2*m6*t2*t5*t6*t8*t11*4.0-Lxcm6*Lycm6*dQ1*dQ2*m6*t3*t5*t6*t7*t11*4.0;
et437 = Lxcm6*Lycm6*dQ1*dQ3*m6*t2*t5*t6*t8*t11*-4.0-Lxcm6*Lycm6*dQ1*dQ3*m6*t3*t5*t6*t7*t11*4.0+Lxcm6*Lycm6*dQ1*dQ5*m6*t2*t3*t6*t10*t11*4.0-Lxcm6*Lycm6*dQ2*dQ3*m6*t4*t5*t6*t9*t11*8.0+Lxcm6*Lycm6*dQ1*dQ2*m6*t5*t7*t8*t9*t10*2.0+Lxcm6*Lycm6*dQ1*dQ3*m6*t5*t7*t8*t9*t10*2.0-Lxcm6*Lycm6*dQ1*dQ5*m6*t6*t7*t8*t10*t11*4.0-Lxcm6*Lycm6*dQ1*dQ2*m6*t2*t4*t8*t9*t35*2.0-Lxcm6*Lycm6*dQ1*dQ2*m6*t3*t4*t7*t9*t35*2.0+Lxcm6*Lycm6*dQ1*dQ2*m6*t2*t4*t8*t9*t36*4.0+Lxcm6*Lycm6*dQ1*dQ2*m6*t3*t4*t7*t9*t36*4.0-Lxcm6*Lycm6*dQ1*dQ3*m6*t2*t4*t8*t9*t35*2.0-Lxcm6*Lycm6*dQ1*dQ3*m6*t3*t4*t7*t9*t35*2.0+Lxcm6*Lycm6*dQ1*dQ3*m6*t2*t4*t8*t9*t36*4.0+Lxcm6*Lycm6*dQ1*dQ3*m6*t3*t4*t7*t9*t36*4.0;
et438 = Lxcm6*Lz6*dQ1*dQ2*m6*t2*t3*t4*t5*t6*2.0+Lxcm6*Lz6*dQ1*dQ3*m6*t2*t3*t4*t5*t6*2.0-Lxcm6*Lz6*dQ1*dQ2*m6*t4*t5*t6*t7*t8*2.0-Lxcm6*Lz6*dQ1*dQ3*m6*t4*t5*t6*t7*t8*2.0+Lxcm6*Lz6*dQ1*dQ4*m6*t2*t3*t5*t10*t11*2.0-Lxcm6*Lz6*dQ1*dQ5*m6*t2*t4*t6*t8*t10*2.0-Lxcm6*Lz6*dQ1*dQ5*m6*t3*t4*t6*t7*t10*2.0-Lxcm6*Lz6*dQ1*dQ4*m6*t5*t7*t8*t10*t11*2.0-Lxcm6*Lz6*dQ1*dQ2*m6*t2*t3*t9*t11*t35*2.0-Lxcm6*Lz6*dQ1*dQ2*m6*t2*t6*t8*t10*t34*2.0-Lxcm6*Lz6*dQ1*dQ2*m6*t3*t6*t7*t10*t34*2.0-Lxcm6*Lz6*dQ1*dQ3*m6*t2*t3*t9*t11*t35*2.0-Lxcm6*Lz6*dQ1*dQ3*m6*t2*t6*t8*t10*t34*2.0-Lxcm6*Lz6*dQ1*dQ3*m6*t3*t6*t7*t10*t34*2.0+Lxcm6*Lz6*dQ1*dQ4*m6*t2*t4*t8*t11*t35*2.0;
et439 = Lxcm6*Lz6*dQ1*dQ4*m6*t3*t4*t7*t11*t35*2.0+Lxcm6*Lz6*dQ1*dQ2*m6*t7*t8*t9*t11*t35*2.0+Lxcm6*Lz6*dQ1*dQ3*m6*t7*t8*t9*t11*t35*2.0+Lxcm6*Lzcm6*dQ1*dQ2*m6*t2*t3*t4*t5*t6*2.0+Lxcm6*Lzcm6*dQ1*dQ3*m6*t2*t3*t4*t5*t6*2.0-Lxcm6*Lzcm6*dQ1*dQ2*m6*t4*t5*t6*t7*t8*2.0-Lxcm6*Lzcm6*dQ1*dQ3*m6*t4*t5*t6*t7*t8*2.0+Lxcm6*Lzcm6*dQ1*dQ4*m6*t2*t3*t5*t10*t11*2.0-Lxcm6*Lzcm6*dQ1*dQ5*m6*t2*t4*t6*t8*t10*2.0-Lxcm6*Lzcm6*dQ1*dQ5*m6*t3*t4*t6*t7*t10*2.0-Lxcm6*Lzcm6*dQ1*dQ4*m6*t5*t7*t8*t10*t11*2.0-Lxcm6*Lzcm6*dQ1*dQ2*m6*t2*t3*t9*t11*t35*2.0-Lxcm6*Lzcm6*dQ1*dQ2*m6*t2*t6*t8*t10*t34*2.0-Lxcm6*Lzcm6*dQ1*dQ2*m6*t3*t6*t7*t10*t34*2.0-Lxcm6*Lzcm6*dQ1*dQ3*m6*t2*t3*t9*t11*t35*2.0;
et440 = Lxcm6*Lzcm6*dQ1*dQ3*m6*t2*t6*t8*t10*t34*-2.0-Lxcm6*Lzcm6*dQ1*dQ3*m6*t3*t6*t7*t10*t34*2.0+Lxcm6*Lzcm6*dQ1*dQ4*m6*t2*t4*t8*t11*t35*2.0+Lxcm6*Lzcm6*dQ1*dQ4*m6*t3*t4*t7*t11*t35*2.0+Lxcm6*Lzcm6*dQ1*dQ2*m6*t7*t8*t9*t11*t35*2.0+Lxcm6*Lzcm6*dQ1*dQ3*m6*t7*t8*t9*t11*t35*2.0-Lycm6*Lz6*dQ1*dQ2*m6*t2*t3*t4*t5*t11*2.0-Lycm6*Lz6*dQ1*dQ3*m6*t2*t3*t4*t5*t11*2.0+Lycm6*Lz6*dQ1*dQ4*m6*t2*t3*t5*t6*t10*2.0+Lycm6*Lz6*dQ1*dQ2*m6*t4*t5*t7*t8*t11*2.0+Lycm6*Lz6*dQ1*dQ3*m6*t4*t5*t7*t8*t11*2.0-Lycm6*Lz6*dQ1*dQ4*m6*t5*t6*t7*t8*t10*2.0+Lycm6*Lz6*dQ1*dQ5*m6*t2*t4*t8*t10*t11*2.0+Lycm6*Lz6*dQ1*dQ5*m6*t3*t4*t7*t10*t11*2.0-Lycm6*Lz6*dQ1*dQ2*m6*t2*t3*t6*t9*t35*2.0-Lycm6*Lz6*dQ1*dQ3*m6*t2*t3*t6*t9*t35*2.0;
et441 = Lycm6*Lz6*dQ1*dQ4*m6*t2*t4*t6*t8*t35*2.0+Lycm6*Lz6*dQ1*dQ4*m6*t3*t4*t6*t7*t35*2.0+Lycm6*Lz6*dQ1*dQ2*m6*t2*t8*t10*t11*t34*2.0+Lycm6*Lz6*dQ1*dQ2*m6*t3*t7*t10*t11*t34*2.0+Lycm6*Lz6*dQ1*dQ2*m6*t6*t7*t8*t9*t35*2.0+Lycm6*Lz6*dQ1*dQ3*m6*t2*t8*t10*t11*t34*2.0+Lycm6*Lz6*dQ1*dQ3*m6*t3*t7*t10*t11*t34*2.0+Lycm6*Lz6*dQ1*dQ3*m6*t6*t7*t8*t9*t35*2.0-Lycm6*Lzcm6*dQ1*dQ2*m6*t2*t3*t4*t5*t11*2.0-Lycm6*Lzcm6*dQ1*dQ3*m6*t2*t3*t4*t5*t11*2.0+Lycm6*Lzcm6*dQ1*dQ4*m6*t2*t3*t5*t6*t10*2.0+Lycm6*Lzcm6*dQ1*dQ2*m6*t4*t5*t7*t8*t11*2.0+Lycm6*Lzcm6*dQ1*dQ3*m6*t4*t5*t7*t8*t11*2.0-Lycm6*Lzcm6*dQ1*dQ4*m6*t5*t6*t7*t8*t10*2.0+Lycm6*Lzcm6*dQ1*dQ5*m6*t2*t4*t8*t10*t11*2.0+Lycm6*Lzcm6*dQ1*dQ5*m6*t3*t4*t7*t10*t11*2.0;
et442 = Lycm6*Lzcm6*dQ1*dQ2*m6*t2*t3*t6*t9*t35*-2.0-Lycm6*Lzcm6*dQ1*dQ3*m6*t2*t3*t6*t9*t35*2.0+Lycm6*Lzcm6*dQ1*dQ4*m6*t2*t4*t6*t8*t35*2.0+Lycm6*Lzcm6*dQ1*dQ4*m6*t3*t4*t6*t7*t35*2.0+Lycm6*Lzcm6*dQ1*dQ2*m6*t2*t8*t10*t11*t34*2.0+Lycm6*Lzcm6*dQ1*dQ2*m6*t3*t7*t10*t11*t34*2.0+Lycm6*Lzcm6*dQ1*dQ2*m6*t6*t7*t8*t9*t35*2.0+Lycm6*Lzcm6*dQ1*dQ3*m6*t2*t8*t10*t11*t34*2.0+Lycm6*Lzcm6*dQ1*dQ3*m6*t3*t7*t10*t11*t34*2.0+Lycm6*Lzcm6*dQ1*dQ3*m6*t6*t7*t8*t9*t35*2.0-Ixx6*dQ1*dQ2*t2*t3*t5*t6*t9*t10*t11*2.0-Ixx6*dQ1*dQ3*t2*t3*t5*t6*t9*t10*t11*2.0+Ixx6*dQ1*dQ2*t5*t6*t7*t8*t9*t10*t11*2.0+Ixx6*dQ1*dQ3*t5*t6*t7*t8*t9*t10*t11*2.0-Ixx6*dQ1*dQ2*t2*t4*t6*t8*t9*t11*t35*2.0-Ixx6*dQ1*dQ2*t3*t4*t6*t7*t9*t11*t35*2.0;
et443 = Ixx6*dQ1*dQ3*t2*t4*t6*t8*t9*t11*t35*-2.0-Ixx6*dQ1*dQ3*t3*t4*t6*t7*t9*t11*t35*2.0+Iyy6*dQ1*dQ2*t2*t3*t5*t6*t9*t10*t11*2.0+Iyy6*dQ1*dQ3*t2*t3*t5*t6*t9*t10*t11*2.0-Iyy6*dQ1*dQ2*t5*t6*t7*t8*t9*t10*t11*2.0-Iyy6*dQ1*dQ3*t5*t6*t7*t8*t9*t10*t11*2.0+Iyy6*dQ1*dQ2*t2*t4*t6*t8*t9*t11*t35*2.0+Iyy6*dQ1*dQ2*t3*t4*t6*t7*t9*t11*t35*2.0+Iyy6*dQ1*dQ3*t2*t4*t6*t8*t9*t11*t35*2.0+Iyy6*dQ1*dQ3*t3*t4*t6*t7*t9*t11*t35*2.0+dQ1*dQ2*m6*t2*t4*t6*t8*t9*t11*t18*2.0+dQ1*dQ2*m6*t3*t4*t6*t7*t9*t11*t18*2.0+dQ1*dQ3*m6*t2*t4*t6*t8*t9*t11*t18*2.0+dQ1*dQ3*m6*t3*t4*t6*t7*t9*t11*t18*2.0-dQ1*dQ2*m6*t2*t4*t6*t8*t9*t11*t21*2.0-dQ1*dQ2*m6*t3*t4*t6*t7*t9*t11*t21*2.0;
et444 = dQ1*dQ3*m6*t2*t4*t6*t8*t9*t11*t21*-2.0-dQ1*dQ3*m6*t3*t4*t6*t7*t9*t11*t21*2.0+dQ1*dQ2*m6*t2*t3*t5*t6*t9*t10*t11*t18*2.0+dQ1*dQ3*m6*t2*t3*t5*t6*t9*t10*t11*t18*2.0-dQ1*dQ4*m6*t2*t4*t5*t6*t8*t10*t11*t18*2.0-dQ1*dQ4*m6*t3*t4*t5*t6*t7*t10*t11*t18*2.0-dQ1*dQ2*m6*t2*t3*t5*t6*t9*t10*t11*t21*2.0-dQ1*dQ3*m6*t2*t3*t5*t6*t9*t10*t11*t21*2.0+dQ1*dQ4*m6*t2*t4*t5*t6*t8*t10*t11*t21*2.0+dQ1*dQ4*m6*t3*t4*t5*t6*t7*t10*t11*t21*2.0-dQ1*dQ2*m6*t5*t6*t7*t8*t9*t10*t11*t18*2.0-dQ1*dQ3*m6*t5*t6*t7*t8*t9*t10*t11*t18*2.0+dQ1*dQ2*m6*t5*t6*t7*t8*t9*t10*t11*t21*2.0+dQ1*dQ3*m6*t5*t6*t7*t8*t9*t10*t11*t21*2.0;
et445 = dQ1*dQ2*m6*t2*t4*t6*t8*t9*t11*t18*t35*2.0+dQ1*dQ2*m6*t3*t4*t6*t7*t9*t11*t18*t35*2.0+dQ1*dQ3*m6*t2*t4*t6*t8*t9*t11*t18*t35*2.0+dQ1*dQ3*m6*t3*t4*t6*t7*t9*t11*t18*t35*2.0-dQ1*dQ2*m6*t2*t4*t6*t8*t9*t11*t21*t35*2.0-dQ1*dQ2*m6*t3*t4*t6*t7*t9*t11*t21*t35*2.0-dQ1*dQ3*m6*t2*t4*t6*t8*t9*t11*t21*t35*2.0-dQ1*dQ3*m6*t3*t4*t6*t7*t9*t11*t21*t35*2.0+Lx4*Lxcm6*dQ1*dQ2*m6*t2*t4*t5*t8*t9*t11*2.0+Lx4*Lxcm6*dQ1*dQ2*m6*t3*t4*t5*t7*t9*t11*2.0+Lx4*Lxcm6*dQ1*dQ3*m6*t2*t4*t5*t8*t9*t11*2.0+Lx4*Lxcm6*dQ1*dQ3*m6*t3*t4*t5*t7*t9*t11*2.0+Lx4*Lycm6*dQ1*dQ2*m6*t2*t4*t5*t6*t8*t9*2.0+Lx4*Lycm6*dQ1*dQ2*m6*t3*t4*t5*t6*t7*t9*2.0+Lx4*Lycm6*dQ1*dQ3*m6*t2*t4*t5*t6*t8*t9*2.0;
et446 = Lx4*Lycm6*dQ1*dQ3*m6*t3*t4*t5*t6*t7*t9*2.0+Lxcm6*Lycm6*dQ1*dQ2*m6*t2*t3*t4*t6*t10*t11*4.0+Lxcm6*Lycm6*dQ1*dQ3*m6*t2*t3*t4*t6*t10*t11*4.0+Lxcm6*Lycm6*dQ1*dQ5*m6*t2*t4*t5*t6*t8*t11*4.0+Lxcm6*Lycm6*dQ1*dQ5*m6*t3*t4*t5*t6*t7*t11*4.0-Lxcm6*Lycm6*dQ1*dQ2*m6*t4*t6*t7*t8*t10*t11*4.0-Lxcm6*Lycm6*dQ1*dQ3*m6*t4*t6*t7*t8*t10*t11*4.0+Lxcm6*Lycm6*dQ1*dQ2*m6*t2*t3*t5*t9*t10*t36*4.0+Lxcm6*Lycm6*dQ1*dQ2*m6*t2*t5*t6*t8*t11*t34*8.0+Lxcm6*Lycm6*dQ1*dQ2*m6*t3*t5*t6*t7*t11*t34*8.0+Lxcm6*Lycm6*dQ1*dQ3*m6*t2*t3*t5*t9*t10*t36*4.0+Lxcm6*Lycm6*dQ1*dQ3*m6*t2*t5*t6*t8*t11*t34*8.0+Lxcm6*Lycm6*dQ1*dQ3*m6*t3*t5*t6*t7*t11*t34*8.0-Lxcm6*Lycm6*dQ1*dQ4*m6*t2*t4*t5*t8*t10*t36*4.0;
et447 = Lxcm6*Lycm6*dQ1*dQ4*m6*t3*t4*t5*t7*t10*t36*-4.0-Lxcm6*Lycm6*dQ1*dQ2*m6*t5*t7*t8*t9*t10*t36*4.0-Lxcm6*Lycm6*dQ1*dQ3*m6*t5*t7*t8*t9*t10*t36*4.0+Lxcm6*Lycm6*dQ1*dQ2*m6*t2*t4*t8*t9*t35*t36*4.0+Lxcm6*Lycm6*dQ1*dQ2*m6*t3*t4*t7*t9*t35*t36*4.0+Lxcm6*Lycm6*dQ1*dQ3*m6*t2*t4*t8*t9*t35*t36*4.0+Lxcm6*Lycm6*dQ1*dQ3*m6*t3*t4*t7*t9*t35*t36*4.0+Lxcm6*Lz6*dQ1*dQ2*m6*t2*t4*t5*t8*t9*t10*t11*2.0+Lxcm6*Lz6*dQ1*dQ2*m6*t3*t4*t5*t7*t9*t10*t11*2.0+Lxcm6*Lz6*dQ1*dQ3*m6*t2*t4*t5*t8*t9*t10*t11*2.0+Lxcm6*Lz6*dQ1*dQ3*m6*t3*t4*t5*t7*t9*t10*t11*2.0+Lxcm6*Lzcm6*dQ1*dQ2*m6*t2*t4*t5*t8*t9*t10*t11*2.0+Lxcm6*Lzcm6*dQ1*dQ2*m6*t3*t4*t5*t7*t9*t10*t11*2.0+Lxcm6*Lzcm6*dQ1*dQ3*m6*t2*t4*t5*t8*t9*t10*t11*2.0;
et448 = Lxcm6*Lzcm6*dQ1*dQ3*m6*t3*t4*t5*t7*t9*t10*t11*2.0+Lycm6*Lz6*dQ1*dQ2*m6*t2*t4*t5*t6*t8*t9*t10*2.0+Lycm6*Lz6*dQ1*dQ2*m6*t3*t4*t5*t6*t7*t9*t10*2.0+Lycm6*Lz6*dQ1*dQ3*m6*t2*t4*t5*t6*t8*t9*t10*2.0+Lycm6*Lz6*dQ1*dQ3*m6*t3*t4*t5*t6*t7*t9*t10*2.0+Lycm6*Lzcm6*dQ1*dQ2*m6*t2*t4*t5*t6*t8*t9*t10*2.0+Lycm6*Lzcm6*dQ1*dQ2*m6*t3*t4*t5*t6*t7*t9*t10*2.0+Lycm6*Lzcm6*dQ1*dQ3*m6*t2*t4*t5*t6*t8*t9*t10*2.0+Lycm6*Lzcm6*dQ1*dQ3*m6*t3*t4*t5*t6*t7*t9*t10*2.0;
out1 = [et290+et291;et292+et293+et294+et295+et296+et297+et298+et299+et300+et301+et302+et303+et304;et305+et306+et307+et308+et309+et310;et311+et312+et313+et314+et315+et316+et317+et318+et319+et320+et321+et322+et323+et324+et325+et326+et327+et328+et329+et330+et331+et332+et333+et334+et335+et336+et337+et338+et339+et340+et341+et342+et343+et344+et345+et346+et347+et348+et349+et350+et351+et352+et353+et354+et355+et356+et357+et358+et359+et360+et361+et362+et363+et364+et365+et366+et367+et368+et369+et370+et371;et372+et373+et374+et375+et376+et377+et378+et379+et380+et381+et382+et383+et384+et385+et386+et387+et388+et389+et390+et391+et392+et393+et394+et395+et396+et397+et398+et399+et400+et401+et402+et403+et404+et405+et406+et407+et408+et409+et410+et411+et412+et413+et414+et415+et416;et417+et418+et419+et420+et421+et422+et423+et424+et425+et426+et427+et428+et429+et430+et431+et432+et433+et434+et435+et436+et437+et438+et439+et440+et441+et442+et443+et444+et445+et446+et447+et448];
end
